simulink model "Adaptive_BS_jointspace"  (R2021b)
settings: Solver=VariableStepAuto  StartTime=0.0  StopTime=15.0  RelTol=1e1
undefined symbols (not defined in the file): Kd, l1, l2, l3, l4, l5, l6, lambda, m1, m2, m3, m4, m5, m6, q0, r
libraries: roblocks x3
(part 3 of 5)

== matlab function Adaptive_BS_jointspace/ABS control/reg2 ==
  data: q input; Yr output; qd input; qrd input; qrdd input
function Yr = reg(q, qd, qrd, qrdd)

q1 = q(1);
q2 = q(2);
q3 = q(3);
q4 = q(4);
q5 = q(5);
q6 = q(6);

qd1 = qd(1);
qd2 = qd(2);
qd3 = qd(3);
qd4 = qd(4);
qd5 = qd(5);
qd6 = qd(6);

qrd1 = qrd(1);
qrd2 = qrd(2);
qrd3 = qrd(3);
qrd4 = qrd(4);
qrd5 = qrd(5);
qrd6 = qrd(6);

qrdd1 = qrdd(1);
qrdd2 = qrdd(2);
qrdd3 = qrdd(3);
qrdd4 = qrdd(4);
qrdd5 = qrdd(5);
qrdd6 = qrdd(6);

%#codegen
%    This function was generated by the Symbolic Math Toolbox version 9.0.
%    01-Oct-2022 23:52:12

t2 = cos(q1);
t3 = cos(q2);
t4 = cos(q3);
t5 = cos(q4);
t6 = cos(q5);
t7 = cos(q6);
t8 = sin(q1);
t9 = sin(q2);
t10 = sin(q3);
t11 = sin(q4);
t12 = sin(q5);
t13 = sin(q6);
t14 = q2+q3;
t23 = -q5;
t15 = t2.^2;
t16 = t6.^2;
t17 = t8.^2;
t18 = t9.^2;
t19 = t12.^2;
t20 = cos(t14);
t21 = q4+t14;
t22 = sin(t14);
t24 = t2.*t6;
t26 = t2.*t12;
t27 = t6.*t8;
t30 = t8.*t12;
t33 = t3.*6.12e+3;
t34 = t9.*6.12e+3;
t56 = t3.*(1.53e+2./2.5e+2);
t57 = t2.*(1.53e+2./5.0e+2);
t63 = t9.*(1.53e+2./2.5e+2);
t64 = t8.*(1.53e+2./5.0e+2);
t90 = t2.*t3.*(-1.53e+2./2.5e+2);
t91 = t3.*t8.*(-1.53e+2./2.5e+2);
t92 = t2.*1.639e-1;
t93 = t2.*2.8615e-1;
t94 = t8.*1.639e-1;
t95 = t8.*2.8615e-1;
t119 = t3.*6.00372;
t138 = t8.*t9.*t10.*5.723e-1;
t148 = t2.*t3.*t4.*5.723e-1;
t152 = t2.*t3.*t10.*5.723e-1;
t153 = t2.*t4.*t9.*5.723e-1;
t154 = t3.*t4.*t8.*5.723e-1;
t157 = t2.*t9.*t10.*5.723e-1;
t158 = t3.*t8.*t10.*5.723e-1;
t159 = t4.*t8.*t9.*5.723e-1;
t25 = cos(t21);
t28 = q5+t21;
t29 = sin(t21);
t31 = t22.^2;
t41 = t21+t23;
t42 = t20.*5.723e+3;
t43 = t22.*5.723e+3;
t44 = t15+t17;
t71 = t2.*t56;
t74 = t2.*t63;
t75 = t8.*t56;
t79 = t8.*t63;
t109 = t20.*5.723e-1;
t110 = t24.*1.383e-1;
t111 = t24.*5.785e-2;
t112 = t22.*5.723e-1;
t113 = t26.*1.383e-1;
t114 = t27.*1.383e-1;
t115 = t26.*5.785e-2;
t116 = t27.*5.785e-2;
t117 = t30.*1.383e-1;
t118 = t30.*5.785e-2;
t122 = t5.*t20.*9.22e-2;
t123 = t11.*t20.*9.22e-2;
t124 = t5.*t22.*9.22e-2;
t125 = t11.*t22.*9.22e-2;
t127 = -t119;
t147 = t5.*t20.*1.157e-1;
t149 = t11.*t20.*1.157e-1;
t150 = t5.*t22.*1.157e-1;
t155 = t11.*t22.*1.157e-1;
t161 = -t138;
t173 = -t148;
t176 = t2.*t22.*(-5.723e-1);
t178 = t8.*t22.*(-5.723e-1);
t198 = t20.*5.614263;
t217 = t8.*t11.*t20.*(-1.157e-1);
t218 = t2.*t11.*t22.*(-1.157e-1);
t219 = t5.*t8.*t22.*(-1.157e-1);
t220 = t8.*t11.*t22.*(-1.157e-1);
t261 = t57+t91;
t331 = t17.*t20.*t22.*3.2752729e-1;
t338 = t15.*t20.*t22.*3.2752729e-1;
t32 = sin(t28);
t35 = t25.^2;
t36 = t29.^2;
t37 = t7.*t25;
t38 = t13.*t25;
t39 = t7.*t29;
t40 = t13.*t29;
t45 = sin(t41);
t46 = t24.*t25;
t49 = t25.*t26;
t50 = t25.*t27;
t58 = t25.*t30;
t87 = t25.*t29.*2.0;
t96 = t6.*t25.*t29;
t97 = t12.*t25.*t29;
t126 = -t109;
t128 = t25.*1.157e-1;
t129 = t25.*8.195e-2;
t130 = t29.*1.157e-1;
t131 = t29.*8.195e-2;
t137 = -t125;
t139 = t12.*t25.*4.61e-2;
t140 = t6.*t29.*4.61e-2;
t141 = t12.*t29.*4.61e-2;
t145 = t33+t42;
t146 = t34+t43;
t151 = t2.*t112;
t156 = t8.*t112;
t164 = t12.*t25.*5.785e-2;
t167 = t12.*t29.*5.785e-2;
t174 = -t149;
t175 = -t150;
t177 = -t155;
t179 = t15.*t112;
t180 = t17.*t112;
t182 = t8.*t29.*(-8.195e-2);
t184 = t2.*t147;
t185 = t2.*t149;
t186 = t8.*t147;
t187 = t2.*t150;
t188 = t8.*t149;
t189 = t2.*t155;
t190 = t8.*t150;
t193 = t8.*t155;
t208 = t29.*t113;
t210 = t29.*t115;
t211 = t29.*t117;
t212 = t29.*t118;
t213 = (t15.*t44)./5.0e+3;
t214 = (t17.*t44)./5.0e+3;
t222 = -t198;
t230 = t29.*1.135017;
t231 = t29.*8.039295e-1;
t236 = (t19.*t25.*t29)./2.5e+3;
t237 = (t19.*t25.*t29)./5.0e+3;
t253 = t64+t71;
t276 = t56+t109;
t277 = t63+t112;
t299 = t8.*t261;
t335 = t123+t124;
t346 = t15.*t25.*t29.*6.7158025e-3;
t348 = t17.*t25.*t29.*6.7158025e-3;
t376 = t74.*t261;
t377 = t79.*t261;
t487 = t25.*t29.*2.138600833333333e-3;
t508 = t25.*t29.*1.215540833333333e-3;
t509 = t25.*t29.*2.431081666666667e-3;
t513 = t15.*t44.*2.338600833333333e-3;
t514 = t17.*t44.*2.338600833333333e-3;
t47 = t2.*t37;
t48 = t6.*t37;
t51 = t2.*t38;
t52 = t8.*t37;
t53 = t2.*t39;
t54 = t6.*t38;
t55 = t6.*t39;
t59 = t8.*t38;
t60 = t2.*t40;
t61 = t8.*t39;
t62 = t6.*t40;
t65 = t8.*t40;
t66 = t6.*t35;
t67 = t12.*t35;
t68 = t6.*t36;
t69 = t12.*t36;
t70 = t24.*t39;
t72 = t24.*t40;
t73 = t27.*t39;
t76 = t15.*t36;
t78 = t27.*t40;
t80 = t17.*t36;
t81 = t19.*t36;
t82 = -t49;
t83 = -t50;
t98 = -t87;
t120 = t12.*t29.*t37;
t121 = t12.*t29.*t38;
t132 = t24+t58;
t133 = t30+t46;
t134 = t15.*t87;
t135 = t17.*t87;
t136 = t19.*t87;
t142 = -t128;
t143 = -t130;
t144 = -t131;
t163 = t2.*t129;
t165 = t8.*t129;
t166 = t2.*t131;
t168 = t8.*t131;
t181 = -t164;
t201 = t46.*1.383e-1;
t202 = t46.*5.785e-2;
t203 = t49.*1.383e-1;
t204 = t50.*1.383e-1;
t205 = t49.*5.785e-2;
t206 = t50.*5.785e-2;
t207 = t58.*1.383e-1;
t209 = t58.*5.785e-2;
t215 = t15.*t129;
t216 = t17.*t129;
t242 = t36.*t111;
t243 = t36.*t116;
t244 = -t236;
t245 = -t237;
t246 = t32.*6.783615e-1;
t247 = t32.*2.8375425e-1;
t252 = t27.*t36.*(-5.785e-2);
t266 = t45.*6.783615e-1;
t267 = t45.*2.8375425e-1;
t279 = t2.*t253;
t296 = (t2.*t145)./1.0e+4;
t297 = (t8.*t145)./1.0e+4;
t298 = (t2.*t146)./1.0e+4;
t301 = (t8.*t146)./1.0e+4;
t302 = t277.^2;
t317 = (t15.*t146)./1.0e+4;
t322 = (t17.*t146)./1.0e+4;
t324 = -t299;
t343 = t122+t137;
t347 = t112+t129;
t355 = t126+t131;
t359 = t6.*t335;
t360 = t12.*t335;
t363 = t128+t167;
t367 = t74.*t253;
t368 = t79.*t253;
t384 = t9.*t299.*(-1.53e+2./2.5e+2);
t390 = t179+t180;
t408 = t129+t277;
t447 = t180.*t277;
t454 = t15.*t109.*t277;
t459 = t17.*t109.*t277;
t460 = t179.*t277;
t479 = t35.*1.215540833333333e-3;
t490 = t2.*t36.*1.215540833333333e-3;
t492 = t8.*t36.*1.215540833333333e-3;
t510 = t16.*t36.*1.215540833333333e-3;
t516 = -t509;
t517 = -t508;
t527 = t2.*t508;
t528 = t8.*t508;
t542 = t16.*t508;
t543 = t16.*t509;
t567 = t184+t208+t218;
t568 = t184+t210+t218;
t569 = t186+t211+t220;
t570 = t186+t212+t220;
t638 = t92+t154+t161+t182;
t77 = -t48;
t84 = -t60;
t85 = -t61;
t86 = -t62;
t88 = -t68;
t89 = -t69;
t99 = t12.*t68.*2.0;
t100 = t17.*t69;
t101 = t13.*t81;
t102 = -t72;
t103 = -t78;
t105 = t15.*t68;
t106 = t17.*t68;
t107 = t15.*t69;
t108 = t7.*t81;
t160 = t132.^2;
t162 = t81./5.0e+3;
t169 = (t12.*t68)./2.5e+3;
t170 = (t12.*t68)./5.0e+3;
t171 = t26+t83;
t172 = t27+t82;
t191 = t2.*t132;
t192 = t7.*t133;
t194 = t38+t55;
t195 = t39+t54;
t196 = t8.*t133;
t197 = t13.*t133;
t223 = -t203;
t224 = -t204;
t225 = -t205;
t226 = -t206;
t251 = t51+t70;
t254 = t59+t73;
t257 = -t246;
t258 = -t247;
t259 = t8.*t81.*1.383e-1;
t260 = t8.*t29.*t132;
t262 = t2.*t25.*t133;
t263 = t2.*t81.*1.383e-1;
t264 = t8.*t25.*t132;
t265 = t2.*t29.*t133;
t280 = t61.*t132;
t284 = t65.*t132;
t300 = t29.*t30.*t132.*2.0;
t305 = -t297;
t310 = -t298;
t313 = -t301;
t325 = (t12.*t29.*t132)./5.0e+3;
t326 = (t12.*t29.*t133)./5.0e+3;
t329 = (t12.*t25.*t132)./5.0e+3;
t330 = (t6.*t29.*t132)./5.0e+3;
t342 = t35+t76+t80;
t358 = t347.^2;
t364 = t12.*t343;
t370 = t130+t181;
t371 = t110+t207;
t372 = t117+t201;
t373 = t118+t202;
t378 = t132.*t208;
t379 = t363.^2;
t403 = t95+t296;
t405 = t215+t216;
t423 = t144+t276;
t424 = t2.*t25.*t363;
t425 = t8.*t25.*t363;
t426 = t2.*t29.*t363;
t427 = t8.*t29.*t363;
t432 = t408.^2;
t434 = -t2.*(t298-t2.*t9.*(1.53e+2./2.5e+2));
t440 = -t8.*(t301-t8.*t9.*(1.53e+2./2.5e+2));
t462 = t98+t134+t135;
t480 = t112+t363;
t481 = t109+t143+t164;
t488 = t2.*t479;
t489 = t8.*t479;
t491 = t140+t359;
t493 = t215.*t347;
t494 = t216.*t347;
t495 = t15.*t131.*t347;
t497 = t17.*t131.*t347;
t498 = -t490;
t499 = -t492;
t500 = t152+t153+t163;
t503 = t215.*t355;
t504 = t216.*t355;
t507 = t158+t159+t165;
t518 = t12.*t68.*1.015540833333333e-3;
t529 = t279+t324;
t530 = t16.*t490;
t531 = t16.*t492;
t551 = t6.*t15.*t29.*t363.*5.785e-2;
t552 = t6.*t15.*t29.*t363.*2.8925e-2;
t553 = t6.*t17.*t29.*t363.*5.785e-2;
t554 = t6.*t17.*t29.*t363.*2.8925e-2;
t561 = t317+t322;
t574 = t277+t363;
t575 = t143+t164+t276;
t577 = t215.*t408;
t578 = t216.*t408;
t579 = t15.*t131.*t408;
t581 = t17.*t131.*t408;
t582 = t2.*t567;
t583 = t2.*t568;
t584 = t8.*t569;
t585 = t8.*t570;
t586 = t15.*t29.*t408.*(-8.195e-2);
t587 = t17.*t29.*t408.*(-8.195e-2);
t603 = t6.*t25.*t133.*1.215540833333333e-3;
t604 = t6.*t29.*t132.*1.015540833333333e-3;
t605 = t6.*t29.*t133.*1.215540833333333e-3;
t606 = t12.*t29.*t133.*1.015540833333333e-3;
t608 = t25.*t567;
t609 = t25.*t568;
t610 = t25.*t569;
t611 = t25.*t570;
t623 = t94+t157+t166+t173;
t631 = t8.*t29.*t567;
t632 = t8.*t29.*t568;
t634 = t2.*t29.*t569;
t635 = t2.*t29.*t570;
t643 = t15.*t347.*t355;
t646 = t17.*t347.*t355;
t650 = t8.*t638;
t668 = t368+t376;
t671 = t367+t384;
t686 = t111+t209+t217+t219;
t694 = t15.*t347.*t408;
t695 = t17.*t347.*t408;
t696 = t75+t638;
t702 = t15.*t355.*t408;
t703 = t17.*t355.*t408;
t763 = t141+t147+t177+t360;
t811 = t158+t159+t569;
t812 = t158+t159+t570;
t818 = t152+t153+t567;
t819 = t152+t153+t568;
t1021 = t236+t516+t543;
t104 = -t99;
t183 = -t170;
t199 = t172.^2;
t200 = t8.*t162;
t221 = t2.*t162;
t227 = t7.*t160;
t228 = t194.^2;
t229 = t13.*t160;
t232 = t7.*t191;
t233 = t13.*t191;
t234 = t2.*t171;
t235 = t7.*t171;
t238 = t37+t86;
t239 = t40+t77;
t240 = t8.*t172;
t241 = t13.*t171;
t268 = t25.*t194;
t269 = t25.*t195;
t270 = t29.*t194;
t271 = t47+t102;
t272 = t52+t103;
t273 = -t263;
t274 = t8.*t29.*t171;
t275 = -t260;
t278 = t8.*t251;
t281 = t2.*t254;
t282 = t2.*t25.*t172;
t283 = -t262;
t285 = t8.*t25.*t171;
t286 = t2.*t29.*t172;
t287 = -t264;
t288 = -t265;
t292 = t12.*t29.*t195;
t303 = t53.*t172;
t306 = t60.*t172;
t307 = t85.*t132;
t311 = -t300;
t312 = -t284;
t323 = t26.*t29.*t172.*2.0;
t327 = t53+t197;
t332 = -t325;
t333 = -t326;
t334 = t8.*t29.*t254;
t337 = t2.*t29.*t251;
t339 = -t329;
t340 = (t12.*t29.*t171)./5.0e+3;
t341 = (t12.*t29.*t172)./5.0e+3;
t344 = t84+t192;
t349 = (t12.*t25.*t172)./5.0e+3;
t350 = (t6.*t29.*t172)./5.0e+3;
t366 = -t8.*(t60-t192);
t374 = t132.*t171.*2.0;
t375 = t133.*t172.*2.0;
t380 = t113+t224;
t381 = t114+t223;
t382 = t115+t226;
t387 = t172.*t211;
t388 = t2.*t372;
t389 = t2.*t373;
t391 = t132.*t254;
t393 = -t2.*t25.*(t60-t192);
t395 = -t2.*t29.*(t60-t192);
t402 = t74+t310;
t404 = t79+t313;
t406 = t25.*t372;
t407 = t25.*t373;
t409 = t93+t305;
t410 = t172.*t251;
t413 = -t26.*t29.*(t60-t192);
t414 = t2.*t29.*(t60-t192);
t428 = t8.*t29.*t372;
t429 = t12.*t29.*t371;
t430 = t12.*t29.*t372;
t431 = t8.*t29.*t373;
t435 = t2.*t29.*t370;
t436 = t2.*t403;
t437 = t8.*t29.*t370;
t439 = t26.*t29.*(t60-t192);
t443 = t12.*t25.*t371;
t444 = t6.*t29.*t371;
t448 = -t424;
t449 = -t425;
t450 = -t426;
t464 = t26.*t29.*t371;
t475 = -t133.*(t60-t192);
t482 = -t172.*(t60-t192);
t483 = t133.*(t60-t192);
t496 = t480.^2;
t505 = t132.*t372;
t506 = t133.*t371;
t511 = t90+t403;
t525 = t172.*t371;
t540 = t2.*t500;
t541 = t8.*t507;
t555 = t8.*t109.*t403;
t556 = t151.*t403;
t558 = t156.*t403;
t572 = t2.*t29.*t491;
t573 = t8.*t29.*t491;
t580 = t574.^2;
t595 = t74+t500;
t596 = t79+t507;
t619 = -t603;
t620 = -t604;
t621 = -t605;
Yr = ft_1({qd1,qd2,qd3,qd4,qd5,qd6,qrd1,qrd2,qrd3,qrd4,qrd5,qrd6,qrdd1,qrdd2,qrdd3,qrdd4,qrdd5,qrdd6,t100,t101,t1021,t104,t105,t106,t107,t108,t109,t111,t112,t116,t12,t120,t121,t127,t13,t130,t132,t133,t136,t139,t142,t144,t146,t15,t151,t154,t156,t157,t160,t161,t162,t163,t165,t166,t168,t169,t17,t170,t171,t172,t173,t174,t175,t176,t178,t179,t18,t180,t183,t185,t187,t191,t192,t194,t195,t196,t199,t2,t20,t200,t213,t214,t215,t216,t217,t219,t221,t222,t225,t227,t228,t229,t230,t231,t232,t233,t234,t235,t237,t238,t239,t24,t240,t241,t242,t243,t244,t245,t25,t251,t252,t253,t254,t257,t258,t259,t26,t261,t263,t266,t267,t268,t269,t27,t270,t271,t272,t273,t274,t275,t276,t277,t278,t279,t281,t282,t283,t285,t286,t287,t288,t29,t292,t296,t298,t3,t30,t301,t302,t303,t305,t306,t307,t31,t311,t312,t323,t325,t326,t327,t330,t331,t332,t333,t334,t337,t338,t339,t340,t341,t342,t346,t347,t348,t349,t35,t350,t355,t358,t36,t363,t364,t366,t370,t371,t372,t373,t374,t375,t377,t378,t379,t380,t381,t382,t387,t388,t389,t39,t390,t391,t393,t40,t402,t403,t404,t405,t406,t407,t408,t409,t410,t414,t423,t424,t426,t427,t428,t429,t430,t431,t432,t434,t435,t436,t437,t439,t440,t443,t444,t447,t448,t449,t450,t454,t459,t460,t462,t464,t479,t480,t481,t482,t483,t487,t488,t489,t491,t493,t494,t495,t496,t497,t498,t499,t500,t503,t504,t505,t506,t507,t510,t511,t513,t514,t517,t518,t525,t527,t528,t529,t530,t531,t540,t541,t542,t551,t552,t553,t554,t555,t556,t558,t561,t567,t568,t569,t570,t572,t573,t574,t575,t577,t578,t579,t580,t581,t582,t583,t584,t585,t586,t587,t595,t596,t6,t60,t604,t606,t608,t609,t61,t610,t611,t619,t620,t621,t623,t63,t631,t632,t634,t635,t643,t646,t65,t650,t66,t668,t67,t68,t686,t694,t695,t696,t7,t702,t703,t71,t74,t75,t763,t79,t8,t81,t811,t812,t818,t819,t85,t88,t89,t9,t90,t92,t94,t96,t97});
end
function Yr = ft_1(ct)
qd1 = ct{1};
qd2 = ct{2};
qd3 = ct{3};
qd4 = ct{4};
qd5 = ct{5};
qd6 = ct{6};
qrd1 = ct{7};
qrd2 = ct{8};
qrd3 = ct{9};
qrd4 = ct{10};
qrd5 = ct{11};
qrd6 = ct{12};
qrdd1 = ct{13};
qrdd2 = ct{14};
qrdd3 = ct{15};
qrdd4 = ct{16};
qrdd5 = ct{17};
qrdd6 = ct{18};
t100 = ct{19};
t101 = ct{20};
t1021 = ct{21};
t104 = ct{22};
t105 = ct{23};
t106 = ct{24};
t107 = ct{25};
t108 = ct{26};
t109 = ct{27};
t111 = ct{28};
t112 = ct{29};
t116 = ct{30};
t12 = ct{31};
t120 = ct{32};
t121 = ct{33};
t127 = ct{34};
t13 = ct{35};
t130 = ct{36};
t132 = ct{37};
t133 = ct{38};
t136 = ct{39};
t139 = ct{40};
t142 = ct{41};
t144 = ct{42};
t146 = ct{43};
t15 = ct{44};
t151 = ct{45};
t154 = ct{46};
t156 = ct{47};
t157 = ct{48};
t160 = ct{49};
t161 = ct{50};
t162 = ct{51};
t163 = ct{52};
t165 = ct{53};
t166 = ct{54};
t168 = ct{55};
t169 = ct{56};
t17 = ct{57};
t170 = ct{58};
t171 = ct{59};
t172 = ct{60};
t173 = ct{61};
t174 = ct{62};
t175 = ct{63};
t176 = ct{64};
t178 = ct{65};
t179 = ct{66};
t18 = ct{67};
t180 = ct{68};
t183 = ct{69};
t185 = ct{70};
t187 = ct{71};
t191 = ct{72};
t192 = ct{73};
t194 = ct{74};
t195 = ct{75};
t196 = ct{76};
t199 = ct{77};
t2 = ct{78};
t20 = ct{79};
t200 = ct{80};
t213 = ct{81};
t214 = ct{82};
t215 = ct{83};
t216 = ct{84};
t217 = ct{85};
t219 = ct{86};
t221 = ct{87};
t222 = ct{88};
t225 = ct{89};
t227 = ct{90};
t228 = ct{91};
t229 = ct{92};
t230 = ct{93};
t231 = ct{94};
t232 = ct{95};
t233 = ct{96};
t234 = ct{97};
t235 = ct{98};
t237 = ct{99};
t238 = ct{100};
t239 = ct{101};
t24 = ct{102};
t240 = ct{103};
t241 = ct{104};
t242 = ct{105};
t243 = ct{106};
t244 = ct{107};
t245 = ct{108};
t25 = ct{109};
t251 = ct{110};
t252 = ct{111};
t253 = ct{112};
t254 = ct{113};
t257 = ct{114};
t258 = ct{115};
t259 = ct{116};
t26 = ct{117};
t261 = ct{118};
t263 = ct{119};
t266 = ct{120};
t267 = ct{121};
t268 = ct{122};
t269 = ct{123};
t27 = ct{124};
t270 = ct{125};
t271 = ct{126};
t272 = ct{127};
t273 = ct{128};
t274 = ct{129};
t275 = ct{130};
t276 = ct{131};
t277 = ct{132};
t278 = ct{133};
t279 = ct{134};
t281 = ct{135};
t282 = ct{136};
t283 = ct{137};
t285 = ct{138};
t286 = ct{139};
t287 = ct{140};
t288 = ct{141};
t29 = ct{142};
t292 = ct{143};
t296 = ct{144};
t298 = ct{145};
t3 = ct{146};
t30 = ct{147};
t301 = ct{148};
t302 = ct{149};
t303 = ct{150};
t305 = ct{151};
t306 = ct{152};
t307 = ct{153};
t31 = ct{154};
t311 = ct{155};
t312 = ct{156};
t323 = ct{157};
t325 = ct{158};
t326 = ct{159};
t327 = ct{160};
t330 = ct{161};
t331 = ct{162};
t332 = ct{163};
t333 = ct{164};
t334 = ct{165};
t337 = ct{166};
t338 = ct{167};
t339 = ct{168};
t340 = ct{169};
t341 = ct{170};
t342 = ct{171};
t346 = ct{172};
t347 = ct{173};
t348 = ct{174};
t349 = ct{175};
t35 = ct{176};
t350 = ct{177};
t355 = ct{178};
t358 = ct{179};
t36 = ct{180};
t363 = ct{181};
t364 = ct{182};
t366 = ct{183};
t370 = ct{184};
t371 = ct{185};
t372 = ct{186};
t373 = ct{187};
t374 = ct{188};
t375 = ct{189};
t377 = ct{190};
t378 = ct{191};
t379 = ct{192};
t380 = ct{193};
t381 = ct{194};
t382 = ct{195};
t387 = ct{196};
t388 = ct{197};
t389 = ct{198};
t39 = ct{199};
t390 = ct{200};
t391 = ct{201};
t393 = ct{202};
t40 = ct{203};
t402 = ct{204};
t403 = ct{205};
t404 = ct{206};
t405 = ct{207};
t406 = ct{208};
t407 = ct{209};
t408 = ct{210};
t409 = ct{211};
t410 = ct{212};
t414 = ct{213};
t423 = ct{214};
t424 = ct{215};
t426 = ct{216};
t427 = ct{217};
t428 = ct{218};
t429 = ct{219};
t430 = ct{220};
t431 = ct{221};
t432 = ct{222};
t434 = ct{223};
t435 = ct{224};
t436 = ct{225};
t437 = ct{226};
t439 = ct{227};
t440 = ct{228};
t443 = ct{229};
t444 = ct{230};
t447 = ct{231};
t448 = ct{232};
t449 = ct{233};
t450 = ct{234};
t454 = ct{235};
t459 = ct{236};
t460 = ct{237};
t462 = ct{238};
t464 = ct{239};
t479 = ct{240};
t480 = ct{241};
t481 = ct{242};
t482 = ct{243};
t483 = ct{244};
t487 = ct{245};
t488 = ct{246};
t489 = ct{247};
t491 = ct{248};
t493 = ct{249};
t494 = ct{250};
t495 = ct{251};
t496 = ct{252};
t497 = ct{253};
t498 = ct{254};
t499 = ct{255};
t500 = ct{256};
t503 = ct{257};
t504 = ct{258};
t505 = ct{259};
t506 = ct{260};
t507 = ct{261};
t510 = ct{262};
t511 = ct{263};
t513 = ct{264};
t514 = ct{265};
t517 = ct{266};
t518 = ct{267};
t525 = ct{268};
t527 = ct{269};
t528 = ct{270};
t529 = ct{271};
t530 = ct{272};
t531 = ct{273};
t540 = ct{274};
t541 = ct{275};
t542 = ct{276};
t551 = ct{277};
t552 = ct{278};
t553 = ct{279};
t554 = ct{280};
t555 = ct{281};
t556 = ct{282};
t558 = ct{283};
t561 = ct{284};
t567 = ct{285};
t568 = ct{286};
t569 = ct{287};
t570 = ct{288};
t572 = ct{289};
t573 = ct{290};
t574 = ct{291};
t575 = ct{292};
t577 = ct{293};
t578 = ct{294};
t579 = ct{295};
t580 = ct{296};
t581 = ct{297};
t582 = ct{298};
t583 = ct{299};
t584 = ct{300};
t585 = ct{301};
t586 = ct{302};
t587 = ct{303};
t595 = ct{304};
t596 = ct{305};
t6 = ct{306};
t60 = ct{307};
t604 = ct{308};
t606 = ct{309};
t608 = ct{310};
t609 = ct{311};
t61 = ct{312};
t610 = ct{313};
t611 = ct{314};
t619 = ct{315};
t620 = ct{316};
t621 = ct{317};
t623 = ct{318};
t63 = ct{319};
t631 = ct{320};
t632 = ct{321};
t634 = ct{322};
t635 = ct{323};
t643 = ct{324};
t646 = ct{325};
t65 = ct{326};
t650 = ct{327};
t66 = ct{328};
t668 = ct{329};
t67 = ct{330};
t68 = ct{331};
t686 = ct{332};
t694 = ct{333};
t695 = ct{334};
t696 = ct{335};
t7 = ct{336};
t702 = ct{337};
t703 = ct{338};
t71 = ct{339};
t74 = ct{340};
t75 = ct{341};
t763 = ct{342};
t79 = ct{343};
t8 = ct{344};
t81 = ct{345};
t811 = ct{346};
t812 = ct{347};
t818 = ct{348};
t819 = ct{349};
t85 = ct{350};
t88 = ct{351};
t89 = ct{352};
t9 = ct{353};
t90 = ct{354};
t92 = ct{355};
t94 = ct{356};
t96 = ct{357};
t97 = ct{358};
t626 = t6.*t25.*t171.*1.215540833333333e-3;
t627 = t6.*t29.*t171.*1.215540833333333e-3;
t628 = t6.*t29.*t172.*1.015540833333333e-3;
t629 = t298.*t403;
t630 = t12.*t29.*t171.*1.015540833333333e-3;
t633 = -t608;
t639 = t132.*t491;
t642 = t2.*t623;
t644 = t8.*t277.*t403;
t647 = -t634;
t648 = -t635;
t649 = t172.*t491;
t652 = t176+t500;
t653 = t178+t507;
t656 = t8.*t25.*t500.*4.0975e-2;
t657 = t12.*t39.*t194.*8.084033333333334e-4;
t658 = t12.*t39.*t194.*1.616806666666667e-3;
t659 = t2.*t25.*t507.*4.0975e-2;
t663 = t6.*t15.*t29.*t480.*5.785e-2;
t664 = t6.*t15.*t29.*t480.*2.8925e-2;
t666 = t6.*t17.*t29.*t480.*5.785e-2;
t667 = t6.*t17.*t29.*t480.*2.8925e-2;
t670 = -t650;
t681 = t116+t185+t187+t225;
t683 = t15.*t363.*t370;
t684 = t17.*t363.*t370;
t685 = t217+t219+t371;
t689 = (t8.*t363.*t373)./2.0;
t701 = t7.*t132.*t194.*8.084033333333334e-4;
t704 = t90+t623;
t705 = t25.*t342.*1.215540833333333e-3;
t706 = t29.*t342.*6.077704166666666e-4;
t707 = t29.*t342.*1.215540833333333e-3;
t719 = t6.*t15.*t29.*t574.*5.785e-2;
t720 = t6.*t15.*t29.*t574.*2.8925e-2;
t722 = t6.*t17.*t29.*t574.*5.785e-2;
t723 = t6.*t17.*t29.*t574.*2.8925e-2;
t726 = t7.*t172.*t194.*8.084033333333334e-4;
t730 = t25.*t686;
t733 = t29.*t686;
t739 = t8.*t696;
t751 = t12.*t39.*(t60-t192).*(-8.084033333333334e-4);
t760 = t194.*t251.*8.084033333333334e-4;
t761 = t194.*t254.*8.084033333333334e-4;
t766 = t763.^2;
t770 = t434+t440;
t774 = t139+t174+t175+t364;
t775 = t15.*t363.*t480;
t776 = t17.*t363.*t480;
t781 = t15.*t363.*t481;
t782 = t15.*t370.*t480;
t783 = t17.*t363.*t481;
t784 = t17.*t370.*t480;
t795 = (t8.*t373.*t480)./2.0;
t813 = t25.*t462.*6.077704166666666e-4;
t814 = t25.*t462.*1.215540833333333e-3;
t816 = t194.*(t60-t192).*(-8.084033333333334e-4);
t820 = t2.*t25.*t763;
t821 = t8.*t25.*t763;
t822 = t2.*t29.*t763;
t823 = t8.*t29.*t763;
t824 = t194.*(t60-t192).*8.084033333333334e-4;
t827 = t2.*t29.*t462.*1.215540833333333e-3;
t828 = t8.*t29.*t462.*1.215540833333333e-3;
t834 = t2.*t818;
t835 = t2.*t819;
t840 = t8.*t811;
t841 = t8.*t812;
t846 = t163.*t696;
t847 = t165.*t696;
t848 = t166.*t696;
t853 = t15.*t363.*t574;
t854 = t17.*t363.*t574;
t858 = (t2.*t408.*t507)./2.0;
t859 = t15.*t370.*t574;
t860 = t17.*t370.*t574;
t862 = (t8.*t408.*t500)./2.0;
t863 = t112+t763;
t864 = (t8.*t373.*t574)./2.0;
t882 = t142+t763;
t887 = t74+t818;
t888 = t74+t819;
t889 = t15.*t480.*t481;
t890 = t17.*t480.*t481;
t891 = t79+t811;
t892 = t79+t812;
t899 = t305+t696;
t911 = t178+t811;
t912 = t178+t812;
t914 = t277+t763;
t916 = t176+t818;
t917 = t176+t819;
t928 = t2.*t347.*t696;
t929 = t15.*t480.*t574;
t932 = t17.*t480.*t574;
t934 = t2.*t355.*t696;
t935 = t15.*t481.*t574;
t936 = t17.*t481.*t574;
t940 = (t8.*t480.*t568)./2.0;
t941 = (t2.*t480.*t570)./2.0;
t966 = t162+t479+t510;
t977 = t92+t154+t161+t686;
t983 = t2.*t408.*t696;
t985 = (t2.*t570.*t574)./2.0;
t992 = (t8.*t568.*t574)./2.0;
t993 = t582+t584;
t994 = t583+t585;
t1007 = (t8.*t372.*t763)./2.0;
t1027 = t507.*t696;
t1039 = (t8.*t363.*t819)./2.0;
t1041 = (t2.*t363.*t812)./2.0;
t1079 = (t25.*t1021)./2.0;
t1086 = t15.*t491.*t763;
t1087 = t17.*t491.*t763;
t1142 = (t2.*t574.*t812)./2.0;
t1146 = (t8.*t574.*t819)./2.0;
t1259 = (t8.*t763.*t818)./2.0;
t1260 = (t2.*t763.*t811)./2.0;
t248 = t7.*t199;
t249 = t238.^2;
t250 = t13.*t199;
t255 = t7.*t240;
t256 = t13.*t240;
t289 = t12.*t268;
t290 = t6.*t270;
t291 = t12.*t270;
t293 = t25.*t238;
t294 = t25.*t239;
t295 = t29.*t238;
t304 = t8.*t271;
t308 = t2.*t272;
t309 = -t281;
t319 = t12.*t29.*t239;
t321 = -t292;
t345 = t65+t235;
t351 = -t340;
t352 = t8.*t29.*t272;
t353 = -t334;
t354 = t8.*t327;
t356 = t2.*t29.*t271;
t357 = -t337;
t361 = t85+t241;
t383 = -t2.*(t61-t241);
t385 = t2.*t25.*t327;
t386 = t2.*t29.*t327;
t392 = t26.*t29.*t327;
t397 = t8.*t380;
t398 = t8.*t382;
t400 = t191+t240;
t401 = t196+t234;
t411 = t132.*t272;
t412 = -t391;
t416 = -t8.*t25.*(t61-t241);
t420 = -t8.*t29.*(t61-t241);
t421 = t25.*t380;
t422 = t25.*t382;
t433 = t172.*t271;
t441 = -t29.*t30.*(t61-t241);
t442 = t8.*t29.*(t61-t241);
t445 = t12.*t29.*t380;
t446 = t12.*t29.*t381;
t451 = t8.*t409;
t455 = t2.*t29.*t380;
t456 = t12.*t25.*t381;
t457 = t6.*t29.*t381;
t458 = t2.*t29.*t382;
t461 = -t429;
t463 = t29.*t30.*(t61-t241);
t465 = -t443;
t466 = -t444;
t468 = t133.*t327;
t470 = t29.*t30.*t381;
t473 = -t464;
t474 = t172.*t327;
t485 = -t132.*(t61-t241);
t486 = t81+t160+t199;
t501 = -t171.*(t61-t241);
t512 = t75+t409;
t515 = t132.*t381;
t522 = t171.*(t61-t241);
t526 = -t506;
t538 = t171.*t381;
t539 = t172.*t380;
t548 = t2.*t511;
t549 = -t525;
t563 = t2.*t109.*t409;
t564 = t151.*t409;
t565 = t156.*t409;
t571 = t178.*t409;
t576 = -t573;
t591 = t228.*8.084033333333334e-4;
t592 = t242+t407;
t612 = t96+t274+t288;
t615 = t97+t275+t286;
t625 = t8.*t596;
t636 = t2.*t595;
t640 = -t628;
t641 = t301.*t409;
t651 = t2.*t277.*t409;
t660 = t120+t303+t307;
t661 = t121+t306+t312;
t662 = -t656;
t665 = -t658;
t669 = -t659;
t672 = t12.*t40.*t238.*8.084033333333334e-4;
t673 = t12.*t40.*t238.*1.616806666666667e-3;
t674 = t136+t311+t323;
t677 = t2.*t652;
t678 = t8.*t653;
t680 = t185+t187+t381;
t691 = (t2.*t363.*t382)./2.0;
t692 = -t689;
t710 = -t701;
t712 = t25.*t681;
t714 = t29.*t681;
t715 = -t707;
t716 = -t706;
t727 = t12.*t40.*t327.*8.084033333333334e-4;
t728 = t13.*t132.*t238.*8.084033333333334e-4;
t729 = t25.*t685;
t731 = t2.*t705;
t732 = t29.*t685;
t734 = t8.*t705;
t735 = t2.*t707;
t736 = t8.*t707;
t737 = t2.*t704;
t738 = t2.*t25.*t596.*4.0975e-2;
t742 = -t726;
t746 = t194.*t239.*8.084033333333334e-4;
t747 = t194.*t239.*1.616806666666667e-3;
t748 = t195.*t238.*8.084033333333334e-4;
t749 = t195.*t238.*1.616806666666667e-3;
t750 = t8.*t25.*t595.*4.0975e-2;
t753 = t2.*t730;
t755 = t13.*t172.*t238.*8.084033333333334e-4;
t757 = t2.*t733;
t759 = -t739;
t762 = t12.*t40.*(t61-t241).*(-8.084033333333334e-4);
t764 = t104+t374+t375;
t768 = t238.*t271.*8.084033333333334e-4;
t769 = t238.*t272.*8.084033333333334e-4;
t796 = t195.*t327.*8.084033333333334e-4;
t801 = -t782;
t802 = (t2.*t382.*t480)./2.0;
t803 = -t784;
t804 = -t795;
t806 = t402+t500;
t809 = t404+t507;
t815 = t238.*t327.*8.084033333333334e-4;
t829 = t239.*(t60-t192).*(-8.084033333333334e-4);
t831 = t195.*(t61-t241).*(-8.084033333333334e-4);
t836 = t2.*t29.*t774;
t837 = t8.*t29.*t774;
t838 = -t821;
t839 = -t822;
t843 = t163.*t704;
t844 = t165.*t704;
t845 = t168.*t704;
t849 = t238.*(t61-t241).*(-8.084033333333334e-4);
t851 = t25.*t739.*(-8.195e-2);
t870 = -t862;
t871 = (t2.*t382.*t574)./2.0;
t872 = -t864;
t873 = t66+t88+t105+t106+t283+t285;
t875 = (t8.*t347.*t595)./2.0;
t876 = t67+t89+t100+t107+t282+t287;
t877 = t406+t572;
t878 = (t2.*t347.*t596)./2.0;
t879 = t109+t774;
t881 = t863.^2;
t885 = t130+t774;
t893 = t296+t704;
t900 = t2.*t887;
t901 = t2.*t888;
t902 = t8.*t891;
t903 = t8.*t892;
t909 = t8.*t899;
t919 = t540+t541;
t921 = t276+t774;
t922 = t26.*t29.*t882;
t923 = t914.^2;
t924 = t29.*t30.*t882;
t925 = t8.*t347.*t704;
t926 = t2.*t916;
t927 = t2.*t917;
t930 = t8.*t911;
t931 = t8.*t912;
t933 = t8.*t355.*t704;
t946 = -t940;
t960 = t132.*t882;
t961 = t133.*t882;
t968 = t94+t157+t173+t681;
t969 = t171.*t882;
t970 = t172.*t882;
t976 = t92+t154+t161+t685;
t982 = t8.*t408.*t704;
t990 = t427+t730;
t1000 = t8.*t977;
t1002 = -t992;
t1012 = (t2.*t380.*t763)./2.0;
t1013 = -t1007;
t1019 = (t29.*t966)./2.0;
t1028 = t404+t811;
t1029 = t404+t812;
t1033 = t500.*t704;
t1037 = t402+t818;
t1038 = t402+t819;
t1045 = -t1027;
t1047 = t620+t630;
t1050 = -t1039;
t1052 = t75+t977;
t1054 = -t1041;
t1077 = t2.*(t604-t630).*(-1.0./2.0);
t1080 = (t2.*(t604-t630))./2.0;
t1082 = (t8.*t372.*t863)./2.0;
t1085 = t642+t670;
t1090 = (t2.*t380.*t863)./2.0;
t1092 = t596.*t696;
t1095 = t595.*t704;
t1100 = (t8.*t363.*t888)./2.0;
t1101 = t1086./2.0;
t1103 = t1087./2.0;
t1104 = (t2.*t363.*t892)./2.0;
t1119 = (t8.*t372.*t914)./2.0;
t1120 = (t2.*t380.*t914)./2.0;
t1122 = t341+t527+t621;
t1123 = t332+t528+t627;
t1140 = t15.*t491.*t863;
t1141 = t17.*t491.*t863;
t1148 = -t1142;
t1151 = -t1146;
t1153 = (t8.*t480.*t888)./2.0;
t1156 = (t2.*t480.*t892)./2.0;
t1185 = (t8.*t567.*t863)./2.0;
t1188 = (t2.*t569.*t863)./2.0;
t1190 = t15.*t491.*t914;
t1192 = t17.*t491.*t914;
t1235 = (t8.*t567.*t914)./2.0;
t1236 = (t2.*t569.*t914)./2.0;
t1245 = t15.*t763.*t774;
t1246 = t17.*t763.*t774;
t1261 = -t1260;
t1294 = t15.*t763.*t863;
t1295 = t17.*t763.*t863;
t1297 = t834+t840;
t1298 = t835+t841;
t1304 = t15.*t774.*t863;
t1306 = t17.*t774.*t863;
t1321 = (t8.*t763.*t887)./2.0;
t1323 = (t2.*t763.*t891)./2.0;
t1331 = t15.*t763.*t914;
t1332 = t17.*t763.*t914;
t1336 = t17.*t774.*t914;
t1337 = t15.*t774.*t914;
t1350 = (t8.*t818.*t914)./2.0;
t1351 = (t2.*t811.*t914)./2.0;
t1356 = (t8.*t863.*t887)./2.0;
t1358 = (t2.*t863.*t891)./2.0;
t1364 = t15.*t863.*t914;
t1365 = t17.*t863.*t914;
t1414 = t437+t449+t611+t733;
t1503 = t221+t349+t488+t498+t530+t619;
t1505 = t200+t339+t489+t499+t531+t626;
t314 = t12.*t293;
t315 = t6.*t295;
t316 = -t290;
t318 = t12.*t295;
t320 = -t291;
t328 = -t308;
t336 = -t319;
t362 = -t352;
t365 = t2.*t345;
t369 = -t356;
t394 = -t385;
t396 = t8.*t25.*t345;
t399 = t8.*t29.*t345;
t415 = t29.*t30.*t345;
t418 = -t397;
t419 = -t398;
t438 = -t411;
t452 = t232+t255;
t453 = t233+t256;
t467 = -t446;
t469 = -t451;
t471 = -t456;
t472 = -t457;
t476 = -t468;
t477 = t132.*t345;
t478 = -t470;
t484 = t171.*t345;
t519 = t278+t309;
t520 = (t12.*t25.*t400)./5.0e+3;
t521 = (t6.*t29.*t400)./5.0e+3;
t523 = (t12.*t29.*t400)./5.0e+3;
t524 = (t12.*t29.*t401)./5.0e+3;
t533 = (t12.*t25.*t400)./1.0e+4;
t534 = (t6.*t29.*t400)./1.0e+4;
t537 = (t12.*t29.*t401)./1.0e+4;
t544 = (t26.*t29.*t400)./5.0e+3;
t545 = (t29.*t30.*t400)./5.0e+3;
t550 = t8.*t512;
t560 = -t539;
t588 = (t132.*t400)./5.0e+3;
t589 = (t133.*t400)./5.0e+3;
t590 = (t132.*t401)./5.0e+3;
t597 = (t12.*t25.*t486)./5.0e+3;
t598 = (t6.*t29.*t486)./5.0e+3;
t599 = (t12.*t29.*t486)./5.0e+3;
t600 = (t171.*t400)./5.0e+3;
t601 = (t172.*t400)./5.0e+3;
t602 = (t172.*t401)./5.0e+3;
t607 = t249.*8.084033333333334e-4;
t613 = (t12.*t25.*t486)./1.0e+4;
t614 = (t6.*t29.*t486)./1.0e+4;
t616 = t252+t422;
t622 = (t26.*t29.*t486)./5.0e+3;
t624 = (t29.*t30.*t486)./5.0e+3;
t645 = t146.*t451.*(-1.0e-4);
t654 = t354+t383;
t675 = (t132.*t486)./5.0e+3;
t676 = (t133.*t486)./5.0e+3;
t679 = -t672;
t687 = (t171.*t486)./5.0e+3;
t688 = (t172.*t486)./5.0e+3;
t693 = -t691;
t697 = (t12.*t25.*t615)./5.0e+3;
t698 = (t6.*t29.*t615)./5.0e+3;
t699 = (t12.*t29.*t612)./5.0e+3;
t700 = (t12.*t29.*t615)./5.0e+3;
t709 = (t12.*t25.*t615)./1.0e+4;
t711 = t25.*t680;
t713 = t29.*t680;
t721 = (t26.*t29.*t615)./5.0e+3;
t724 = (t29.*t30.*t615)./5.0e+3;
t741 = t8.*t712;
t744 = t8.*t714;
t745 = -t714;
t752 = t2.*t729;
t754 = t12.*t39.*t345.*8.084033333333334e-4;
t756 = t2.*t732;
t758 = -t750;
t765 = (t12.*t29.*t674)./5.0e+3;
t767 = (t12.*t29.*t674)./1.0e+4;
t771 = (t132.*t612)./5.0e+3;
t772 = (t132.*t615)./5.0e+3;
t773 = (t133.*t615)./5.0e+3;
t777 = t428+t455;
t778 = t431+t458;
t785 = t6.*t25.*t401.*6.077704166666666e-4;
t786 = t6.*t25.*t401.*1.215540833333333e-3;
t787 = t6.*t29.*t400.*5.077704166666666e-4;
t788 = t6.*t29.*t400.*1.015540833333333e-3;
t789 = t6.*t29.*t401.*1.215540833333333e-3;
t790 = (t172.*t612)./5.0e+3;
t791 = t12.*t29.*t401.*5.077704166666666e-4;
t792 = t12.*t29.*t401.*1.015540833333333e-3;
t793 = (t171.*t615)./5.0e+3;
t794 = (t172.*t615)./5.0e+3;
t805 = -t796;
t807 = t24.*t29.*t401.*1.215540833333333e-3;
t808 = t27.*t29.*t401.*1.215540833333333e-3;
t810 = -t802;
t817 = t194.*t345.*8.084033333333334e-4;
t826 = t8.*t809;
t830 = t239.*t345.*8.084033333333334e-4;
t832 = t2.*t806;
t833 = (t132.*t674)./5.0e+3;
t850 = (t172.*t674)./5.0e+3;
t852 = -t837;
t855 = t133.*t400.*1.015540833333333e-3;
t856 = t132.*t401.*1.015540833333333e-3;
t857 = t133.*t401.*1.215540833333333e-3;
t861 = (t12.*t29.*t764)./5.0e+3;
t865 = t171.*t400.*1.015540833333333e-3;
t866 = t171.*t401.*1.215540833333333e-3;
t867 = t172.*t401.*1.015540833333333e-3;
t869 = (t12.*t29.*t764)./1.0e+4;
t880 = -t871;
t883 = -t875;
t884 = -t878;
t886 = t421+t576;
t906 = (t132.*t764)./5.0e+3;
t907 = t293+t386+t442;
t908 = t2.*t893;
t913 = (t172.*t764)./5.0e+3;
t915 = t515+t549;
t937 = t6.*t25.*t612.*6.077704166666666e-4;
t938 = t6.*t25.*t612.*1.215540833333333e-3;
t939 = t6.*t29.*t612.*1.215540833333333e-3;
t942 = -t924;
t945 = (t12.*t29.*t876)./5.0e+3;
t948 = t558+t564;
t950 = (t12.*t29.*t876)./1.0e+4;
t951 = t24.*t29.*t612.*1.215540833333333e-3;
t952 = t27.*t29.*t612.*1.215540833333333e-3;
t954 = t555+t563;
t955 = t556+t571;
t962 = t132.*t885;
t967 = t94+t157+t173+t680;
t971 = -t961;
Yr = ft_2({qd1,qd2,qd3,qd4,qd5,qd6,qrd1,qrd2,qrd3,qrd4,qrd5,qrd6,qrdd1,qrdd2,qrdd3,qrdd4,qrdd5,qrdd6,t1000,t1002,t1007,t101,t1012,t1013,t1019,t1028,t1029,t1033,t1037,t1038,t1039,t1041,t1045,t1050,t1052,t1054,t1077,t1079,t108,t1082,t1085,t1086,t1087,t1090,t1092,t1095,t1100,t1101,t1103,t1104,t111,t1119,t1120,t1122,t1123,t1140,t1141,t1142,t1146,t1148,t1151,t1153,t1156,t116,t1185,t1188,t1190,t1192,t12,t1235,t1236,t1245,t1246,t1259,t1260,t1261,t127,t1294,t1295,t1297,t1298,t13,t1304,t1306,t132,t1321,t1323,t133,t1331,t1332,t1336,t1337,t1350,t1351,t1356,t1358,t1364,t1365,t1414,t144,t15,t1503,t1505,t162,t169,t17,t170,t171,t172,t179,t18,t180,t183,t192,t194,t195,t2,t20,t200,t213,t214,t215,t216,t221,t222,t227,t229,t230,t231,t237,t238,t239,t24,t241,t243,t244,t245,t248,t25,t250,t251,t253,t254,t257,t258,t259,t26,t261,t263,t266,t267,t268,t269,t27,t270,t271,t272,t273,t276,t277,t279,t289,t29,t291,t294,t295,t296,t298,t3,t30,t301,t302,t304,t305,t31,t314,t315,t316,t318,t320,t321,t325,t326,t327,t328,t330,t331,t332,t333,t334,t336,t337,t338,t339,t341,t345,t346,t347,t348,t349,t35,t350,t351,t352,t353,t356,t357,t358,t36,t362,t363,t365,t366,t369,t370,t372,t373,t377,t378,t379,t380,t382,t385,t387,t388,t389,t39,t390,t392,t393,t394,t396,t399,t40,t403,t405,t408,t409,t410,t412,t414,t415,t416,t418,t419,t422,t423,t424,t426,t429,t430,t432,t433,t435,t436,t438,t439,t444,t445,t446,t447,t448,t450,t452,t453,t454,t456,t459,t460,t461,t463,t465,t466,t467,t469,t471,t472,t473,t474,t476,t477,t478,t480,t481,t482,t483,t484,t485,t487,t491,t493,t494,t495,t496,t497,t500,t503,t504,t505,t507,t513,t514,t517,t518,t519,t520,t521,t522,t523,t524,t526,t529,t533,t534,t537,t538,t542,t544,t545,t548,t550,t551,t552,t553,t554,t560,t561,t567,t568,t569,t570,t574,t575,t577,t578,t579,t580,t581,t586,t587,t588,t589,t590,t591,t592,t595,t596,t597,t598,t599,t6,t60,t600,t601,t602,t604,t606,t607,t609,t61,t610,t612,t613,t614,t615,t622,t624,t625,t629,t63,t630,t631,t632,t633,t636,t639,t640,t643,t644,t645,t646,t647,t648,t649,t651,t654,t656,t657,t659,t660,t661,t662,t663,t664,t665,t666,t667,t668,t669,t673,t675,t676,t677,t678,t679,t68,t683,t684,t687,t688,t689,t691,t692,t693,t694,t695,t696,t697,t698,t699,t7,t700,t702,t703,t704,t705,t706,t709,t71,t710,t711,t712,t713,t714,t715,t716,t719,t720,t721,t722,t723,t724,t726,t727,t728,t729,t731,t732,t734,t735,t736,t737,t738,t741,t742,t744,t745,t746,t747,t748,t749,t75,t751,t752,t753,t754,t755,t756,t757,t758,t759,t760,t761,t762,t763,t765,t766,t767,t768,t769,t771,t772,t773,t774,t775,t776,t777,t778,t781,t782,t783,t784,t785,t786,t787,t788,t789,t790,t791,t792,t793,t794,t795,t8,t801,t802,t803,t804,t805,t807,t808,t810,t811,t812,t813,t814,t815,t817,t818,t819,t820,t823,t824,t826,t827,t828,t829,t830,t831,t832,t833,t836,t838,t839,t843,t844,t845,t846,t848,t849,t850,t851,t852,t853,t854,t855,t856,t857,t858,t859,t860,t861,t863,t864,t865,t866,t867,t869,t870,t871,t872,t873,t875,t876,t877,t878,t879,t880,t881,t883,t884,t885,t886,t887,t888,t889,t890,t891,t892,t9,t90,t900,t901,t902,t903,t906,t907,t908,t909,t913,t914,t915,t919,t921,t922,t923,t925,t926,t927,t928,t929,t930,t931,t932,t933,t934,t935,t936,t937,t938,t939,t940,t941,t942,t945,t946,t948,t950,t951,t952,t954,t955,t960,t962,t966,t967,t968,t969,t970,t971,t976,t982,t983,t985,t990,t992,t993,t994});
end
function Yr = ft_2(ct)
qd1 = ct{1};
qd2 = ct{2};
qd3 = ct{3};
qd4 = ct{4};
qd5 = ct{5};
qd6 = ct{6};
qrd1 = ct{7};
qrd2 = ct{8};
qrd3 = ct{9};
qrd4 = ct{10};
qrd5 = ct{11};
qrd6 = ct{12};
qrdd1 = ct{13};
qrdd2 = ct{14};
qrdd3 = ct{15};
qrdd4 = ct{16};
qrdd5 = ct{17};
qrdd6 = ct{18};
t1000 = ct{19};
t1002 = ct{20};
t1007 = ct{21};
t101 = ct{22};
t1012 = ct{23};
t1013 = ct{24};
t1019 = ct{25};
t1028 = ct{26};
t1029 = ct{27};
t1033 = ct{28};
t1037 = ct{29};
t1038 = ct{30};
t1039 = ct{31};
t1041 = ct{32};
t1045 = ct{33};
t1050 = ct{34};
t1052 = ct{35};
t1054 = ct{36};
t1077 = ct{37};
t1079 = ct{38};
t108 = ct{39};
t1082 = ct{40};
t1085 = ct{41};
t1086 = ct{42};
t1087 = ct{43};
t1090 = ct{44};
t1092 = ct{45};
t1095 = ct{46};
t1100 = ct{47};
t1101 = ct{48};
t1103 = ct{49};
t1104 = ct{50};
t111 = ct{51};
t1119 = ct{52};
t1120 = ct{53};
t1122 = ct{54};
t1123 = ct{55};
t1140 = ct{56};
t1141 = ct{57};
t1142 = ct{58};
t1146 = ct{59};
t1148 = ct{60};
t1151 = ct{61};
t1153 = ct{62};
t1156 = ct{63};
t116 = ct{64};
t1185 = ct{65};
t1188 = ct{66};
t1190 = ct{67};
t1192 = ct{68};
t12 = ct{69};
t1235 = ct{70};
t1236 = ct{71};
t1245 = ct{72};
t1246 = ct{73};
t1259 = ct{74};
t1260 = ct{75};
t1261 = ct{76};
t127 = ct{77};
t1294 = ct{78};
t1295 = ct{79};
t1297 = ct{80};
t1298 = ct{81};
t13 = ct{82};
t1304 = ct{83};
t1306 = ct{84};
t132 = ct{85};
t1321 = ct{86};
t1323 = ct{87};
t133 = ct{88};
t1331 = ct{89};
t1332 = ct{90};
t1336 = ct{91};
t1337 = ct{92};
t1350 = ct{93};
t1351 = ct{94};
t1356 = ct{95};
t1358 = ct{96};
t1364 = ct{97};
t1365 = ct{98};
t1414 = ct{99};
t144 = ct{100};
t15 = ct{101};
t1503 = ct{102};
t1505 = ct{103};
t162 = ct{104};
t169 = ct{105};
t17 = ct{106};
t170 = ct{107};
t171 = ct{108};
t172 = ct{109};
t179 = ct{110};
t18 = ct{111};
t180 = ct{112};
t183 = ct{113};
t192 = ct{114};
t194 = ct{115};
t195 = ct{116};
t2 = ct{117};
t20 = ct{118};
t200 = ct{119};
t213 = ct{120};
t214 = ct{121};
t215 = ct{122};
t216 = ct{123};
t221 = ct{124};
t222 = ct{125};
t227 = ct{126};
t229 = ct{127};
t230 = ct{128};
t231 = ct{129};
t237 = ct{130};
t238 = ct{131};
t239 = ct{132};
t24 = ct{133};
t241 = ct{134};
t243 = ct{135};
t244 = ct{136};
t245 = ct{137};
t248 = ct{138};
t25 = ct{139};
t250 = ct{140};
t251 = ct{141};
t253 = ct{142};
t254 = ct{143};
t257 = ct{144};
t258 = ct{145};
t259 = ct{146};
t26 = ct{147};
t261 = ct{148};
t263 = ct{149};
t266 = ct{150};
t267 = ct{151};
t268 = ct{152};
t269 = ct{153};
t27 = ct{154};
t270 = ct{155};
t271 = ct{156};
t272 = ct{157};
t273 = ct{158};
t276 = ct{159};
t277 = ct{160};
t279 = ct{161};
t289 = ct{162};
t29 = ct{163};
t291 = ct{164};
t294 = ct{165};
t295 = ct{166};
t296 = ct{167};
t298 = ct{168};
t3 = ct{169};
t30 = ct{170};
t301 = ct{171};
t302 = ct{172};
t304 = ct{173};
t305 = ct{174};
t31 = ct{175};
t314 = ct{176};
t315 = ct{177};
t316 = ct{178};
t318 = ct{179};
t320 = ct{180};
t321 = ct{181};
t325 = ct{182};
t326 = ct{183};
t327 = ct{184};
t328 = ct{185};
t330 = ct{186};
t331 = ct{187};
t332 = ct{188};
t333 = ct{189};
t334 = ct{190};
t336 = ct{191};
t337 = ct{192};
t338 = ct{193};
t339 = ct{194};
t341 = ct{195};
t345 = ct{196};
t346 = ct{197};
t347 = ct{198};
t348 = ct{199};
t349 = ct{200};
t35 = ct{201};
t350 = ct{202};
t351 = ct{203};
t352 = ct{204};
t353 = ct{205};
t356 = ct{206};
t357 = ct{207};
t358 = ct{208};
t36 = ct{209};
t362 = ct{210};
t363 = ct{211};
t365 = ct{212};
t366 = ct{213};
t369 = ct{214};
t370 = ct{215};
t372 = ct{216};
t373 = ct{217};
t377 = ct{218};
t378 = ct{219};
t379 = ct{220};
t380 = ct{221};
t382 = ct{222};
t385 = ct{223};
t387 = ct{224};
t388 = ct{225};
t389 = ct{226};
t39 = ct{227};
t390 = ct{228};
t392 = ct{229};
t393 = ct{230};
t394 = ct{231};
t396 = ct{232};
t399 = ct{233};
t40 = ct{234};
t403 = ct{235};
t405 = ct{236};
t408 = ct{237};
t409 = ct{238};
t410 = ct{239};
t412 = ct{240};
t414 = ct{241};
t415 = ct{242};
t416 = ct{243};
t418 = ct{244};
t419 = ct{245};
t422 = ct{246};
t423 = ct{247};
t424 = ct{248};
t426 = ct{249};
t429 = ct{250};
t430 = ct{251};
t432 = ct{252};
t433 = ct{253};
t435 = ct{254};
t436 = ct{255};
t438 = ct{256};
t439 = ct{257};
t444 = ct{258};
t445 = ct{259};
t446 = ct{260};
t447 = ct{261};
t448 = ct{262};
t450 = ct{263};
t452 = ct{264};
t453 = ct{265};
t454 = ct{266};
t456 = ct{267};
t459 = ct{268};
t460 = ct{269};
t461 = ct{270};
t463 = ct{271};
t465 = ct{272};
t466 = ct{273};
t467 = ct{274};
t469 = ct{275};
t471 = ct{276};
t472 = ct{277};
t473 = ct{278};
t474 = ct{279};
t476 = ct{280};
t477 = ct{281};
t478 = ct{282};
t480 = ct{283};
t481 = ct{284};
t482 = ct{285};
t483 = ct{286};
t484 = ct{287};
t485 = ct{288};
t487 = ct{289};
t491 = ct{290};
t493 = ct{291};
t494 = ct{292};
t495 = ct{293};
t496 = ct{294};
t497 = ct{295};
t500 = ct{296};
t503 = ct{297};
t504 = ct{298};
t505 = ct{299};
t507 = ct{300};
t513 = ct{301};
t514 = ct{302};
t517 = ct{303};
t518 = ct{304};
t519 = ct{305};
t520 = ct{306};
t521 = ct{307};
t522 = ct{308};
t523 = ct{309};
t524 = ct{310};
t526 = ct{311};
t529 = ct{312};
t533 = ct{313};
t534 = ct{314};
t537 = ct{315};
t538 = ct{316};
t542 = ct{317};
t544 = ct{318};
t545 = ct{319};
t548 = ct{320};
t550 = ct{321};
t551 = ct{322};
t552 = ct{323};
t553 = ct{324};
t554 = ct{325};
t560 = ct{326};
t561 = ct{327};
t567 = ct{328};
t568 = ct{329};
t569 = ct{330};
t570 = ct{331};
t574 = ct{332};
t575 = ct{333};
t577 = ct{334};
t578 = ct{335};
t579 = ct{336};
t580 = ct{337};
t581 = ct{338};
t586 = ct{339};
t587 = ct{340};
t588 = ct{341};
t589 = ct{342};
t590 = ct{343};
t591 = ct{344};
t592 = ct{345};
t595 = ct{346};
t596 = ct{347};
t597 = ct{348};
t598 = ct{349};
t599 = ct{350};
t6 = ct{351};
t60 = ct{352};
t600 = ct{353};
t601 = ct{354};
t602 = ct{355};
t604 = ct{356};
t606 = ct{357};
t607 = ct{358};
t609 = ct{359};
t61 = ct{360};
t610 = ct{361};
t612 = ct{362};
t613 = ct{363};
t614 = ct{364};
t615 = ct{365};
t622 = ct{366};
t624 = ct{367};
t625 = ct{368};
t629 = ct{369};
t63 = ct{370};
t630 = ct{371};
t631 = ct{372};
t632 = ct{373};
t633 = ct{374};
t636 = ct{375};
t639 = ct{376};
t640 = ct{377};
t643 = ct{378};
t644 = ct{379};
t645 = ct{380};
t646 = ct{381};
t647 = ct{382};
t648 = ct{383};
t649 = ct{384};
t651 = ct{385};
t654 = ct{386};
t656 = ct{387};
t657 = ct{388};
t659 = ct{389};
t660 = ct{390};
t661 = ct{391};
t662 = ct{392};
t663 = ct{393};
t664 = ct{394};
t665 = ct{395};
t666 = ct{396};
t667 = ct{397};
t668 = ct{398};
t669 = ct{399};
t673 = ct{400};
t675 = ct{401};
t676 = ct{402};
t677 = ct{403};
t678 = ct{404};
t679 = ct{405};
t68 = ct{406};
t683 = ct{407};
t684 = ct{408};
t687 = ct{409};
t688 = ct{410};
t689 = ct{411};
t691 = ct{412};
t692 = ct{413};
t693 = ct{414};
t694 = ct{415};
t695 = ct{416};
t696 = ct{417};
t697 = ct{418};
t698 = ct{419};
t699 = ct{420};
t7 = ct{421};
t700 = ct{422};
t702 = ct{423};
t703 = ct{424};
t704 = ct{425};
t705 = ct{426};
t706 = ct{427};
t709 = ct{428};
t71 = ct{429};
t710 = ct{430};
t711 = ct{431};
t712 = ct{432};
t713 = ct{433};
t714 = ct{434};
t715 = ct{435};
t716 = ct{436};
t719 = ct{437};
t720 = ct{438};
t721 = ct{439};
t722 = ct{440};
t723 = ct{441};
t724 = ct{442};
t726 = ct{443};
t727 = ct{444};
t728 = ct{445};
t729 = ct{446};
t731 = ct{447};
t732 = ct{448};
t734 = ct{449};
t735 = ct{450};
t736 = ct{451};
t737 = ct{452};
t738 = ct{453};
t741 = ct{454};
t742 = ct{455};
t744 = ct{456};
t745 = ct{457};
t746 = ct{458};
t747 = ct{459};
t748 = ct{460};
t749 = ct{461};
t75 = ct{462};
t751 = ct{463};
t752 = ct{464};
t753 = ct{465};
t754 = ct{466};
t755 = ct{467};
t756 = ct{468};
t757 = ct{469};
t758 = ct{470};
t759 = ct{471};
t760 = ct{472};
t761 = ct{473};
t762 = ct{474};
t763 = ct{475};
t765 = ct{476};
t766 = ct{477};
t767 = ct{478};
t768 = ct{479};
t769 = ct{480};
t771 = ct{481};
t772 = ct{482};
t773 = ct{483};
t774 = ct{484};
t775 = ct{485};
t776 = ct{486};
t777 = ct{487};
t778 = ct{488};
t781 = ct{489};
t782 = ct{490};
t783 = ct{491};
t784 = ct{492};
t785 = ct{493};
t786 = ct{494};
t787 = ct{495};
t788 = ct{496};
t789 = ct{497};
t790 = ct{498};
t791 = ct{499};
t792 = ct{500};
t793 = ct{501};
t794 = ct{502};
t795 = ct{503};
t8 = ct{504};
t801 = ct{505};
t802 = ct{506};
t803 = ct{507};
t804 = ct{508};
t805 = ct{509};
t807 = ct{510};
t808 = ct{511};
t810 = ct{512};
t811 = ct{513};
t812 = ct{514};
t813 = ct{515};
t814 = ct{516};
t815 = ct{517};
t817 = ct{518};
t818 = ct{519};
t819 = ct{520};
t820 = ct{521};
t823 = ct{522};
t824 = ct{523};
t826 = ct{524};
t827 = ct{525};
t828 = ct{526};
t829 = ct{527};
t830 = ct{528};
t831 = ct{529};
t832 = ct{530};
t833 = ct{531};
t836 = ct{532};
t838 = ct{533};
t839 = ct{534};
t843 = ct{535};
t844 = ct{536};
t845 = ct{537};
t846 = ct{538};
t848 = ct{539};
t849 = ct{540};
t850 = ct{541};
t851 = ct{542};
t852 = ct{543};
t853 = ct{544};
t854 = ct{545};
t855 = ct{546};
t856 = ct{547};
t857 = ct{548};
t858 = ct{549};
t859 = ct{550};
t860 = ct{551};
t861 = ct{552};
t863 = ct{553};
t864 = ct{554};
t865 = ct{555};
t866 = ct{556};
t867 = ct{557};
t869 = ct{558};
t870 = ct{559};
t871 = ct{560};
t872 = ct{561};
t873 = ct{562};
t875 = ct{563};
t876 = ct{564};
t877 = ct{565};
t878 = ct{566};
t879 = ct{567};
t880 = ct{568};
t881 = ct{569};
t883 = ct{570};
t884 = ct{571};
t885 = ct{572};
t886 = ct{573};
t887 = ct{574};
t888 = ct{575};
t889 = ct{576};
t890 = ct{577};
t891 = ct{578};
t892 = ct{579};
t9 = ct{580};
t90 = ct{581};
t900 = ct{582};
t901 = ct{583};
t902 = ct{584};
t903 = ct{585};
t906 = ct{586};
t907 = ct{587};
t908 = ct{588};
t909 = ct{589};
t913 = ct{590};
t914 = ct{591};
t915 = ct{592};
t919 = ct{593};
t921 = ct{594};
t922 = ct{595};
t923 = ct{596};
t925 = ct{597};
t926 = ct{598};
t927 = ct{599};
t928 = ct{600};
t929 = ct{601};
t930 = ct{602};
t931 = ct{603};
t932 = ct{604};
t933 = ct{605};
t934 = ct{606};
t935 = ct{607};
t936 = ct{608};
t937 = ct{609};
t938 = ct{610};
t939 = ct{611};
t940 = ct{612};
t941 = ct{613};
t942 = ct{614};
t945 = ct{615};
t946 = ct{616};
t948 = ct{617};
t950 = ct{618};
t951 = ct{619};
t952 = ct{620};
t954 = ct{621};
t955 = ct{622};
t960 = ct{623};
t962 = ct{624};
t966 = ct{625};
t967 = ct{626};
t968 = ct{627};
t969 = ct{628};
t970 = ct{629};
t971 = ct{630};
t976 = ct{631};
t982 = ct{632};
t983 = ct{633};
t985 = ct{634};
t990 = ct{635};
t992 = ct{636};
t993 = ct{637};
t994 = ct{638};
t978 = t172.*t885;
t979 = t132.*t612.*1.015540833333333e-3;
t980 = t133.*t612.*1.215540833333333e-3;
t981 = t133.*t615.*1.015540833333333e-3;
t984 = -t969;
t989 = t2.*t968;
t991 = (t132.*t876)./5.0e+3;
t995 = t171.*t612.*1.215540833333333e-3;
t996 = t172.*t612.*1.015540833333333e-3;
t997 = t171.*t615.*1.015540833333333e-3;
t998 = t450+t712;
t999 = t8.*t976;
t1004 = (t172.*t876)./5.0e+3;
t1006 = -t1000;
t1015 = -t1012;
t1022 = -t1019;
t1031 = t194.*t660.*8.084033333333334e-4;
t1046 = t606+t640;
t1049 = t90+t968;
t1051 = t75+t976;
t1053 = t238.*t661.*8.084033333333334e-4;
t1057 = t2.*t1037;
t1058 = t2.*t1038;
t1059 = t625+t636;
t1061 = t8.*t1028;
t1062 = t8.*t1029;
t1073 = t8.*t1052;
t1076 = t644+t651;
t1083 = t656+t669;
t1088 = -t1082;
t1089 = t327.*t661.*8.084033333333334e-4;
t1096 = t29.*t111.*t990;
t1097 = -t1090;
t1098 = t660.*(t60-t192).*(-8.084033333333334e-4);
t1099 = t345.*t660.*8.084033333333334e-4;
t1102 = -t29.*t116.*(t426-t712);
t1105 = -t1092;
t1107 = -t1100;
t1110 = -t1104;
t1111 = t661.*(t61-t241).*(-8.084033333333334e-4);
t1113 = t677+t678;
t1116 = t6.*t29.*t873.*6.077704166666666e-4;
t1117 = t6.*t29.*t873.*1.215540833333333e-3;
t1121 = -t1119;
t1124 = -t1120;
t1126 = t24.*t29.*t1052.*2.8925e-2;
t1135 = t2.*t1123;
t1136 = t8.*t1122;
t1154 = t1140./2.0;
t1155 = t1141./2.0;
t1157 = t133.*t873.*1.215540833333333e-3;
t1161 = -t1156;
t1164 = t2.*t363.*t990;
t1166 = t305+t1052;
t1168 = t169+t665+t673;
t1170 = t171.*t873.*1.215540833333333e-3;
t1171 = -t8.*t363.*(t426-t712);
t1172 = t2.*t370.*t990;
t1173 = -t8.*t370.*(t426-t712);
t1176 = (t2.*t25.*t1122)./2.0;
t1177 = (t8.*t25.*t1123)./2.0;
t1183 = t8.*t370.*(t426-t712);
t1189 = t461+t960;
t1193 = -t1185;
t1194 = -t1188;
t1197 = t737+t759;
t1207 = t1190./2.0;
t1209 = t1192./2.0;
t1221 = t382.*t1052;
t1223 = t2.*t363.*t1052;
t1228 = t2.*t370.*t1052;
t1234 = t729+t823;
t1237 = t2.*t480.*t990;
t1240 = -t1235;
t1241 = -t1236;
t1242 = -t8.*t480.*(t426-t712);
t1243 = t2.*t481.*t990;
t1244 = -t8.*t481.*(t426-t712);
t1257 = t405.*t1085;
t1263 = t2.*t480.*t1052;
t1264 = t244+t747+t749;
t1265 = t2.*t574.*t990;
t1268 = (t570.*t990)./2.0;
t1269 = -t8.*t574.*(t426-t712);
t1273 = t2.*t481.*t1052;
t1274 = t568.*(t426-t712).*(-1.0./2.0);
t1303 = t15.*t763.*t879;
t1305 = t17.*t763.*t879;
t1308 = t570.*t1052;
t1312 = t844+t846;
t1320 = t2.*t574.*t1052;
t1326 = -t1323;
t1342 = t380.*(t429-t960).*(-1.0./2.0);
t1344 = t15.*t863.*t879;
t1346 = t17.*t863.*t879;
t1349 = t372.*(t446-t970).*(-1.0./2.0);
t1352 = -t1350;
t1354 = -t1351;
t1362 = -t1358;
t1366 = t900+t902;
t1367 = t901+t903;
t1368 = t17.*t879.*t914;
t1369 = t15.*t879.*t914;
t1370 = t341+t815+t824;
t1372 = (t812.*t990)./2.0;
t1378 = t819.*(t426-t712).*(-1.0./2.0);
t1379 = t2.*t491.*(t429-t960).*(-1.0./2.0);
t1385 = t8.*t491.*(t446-t970).*(-1.0./2.0);
t1388 = t812.*t1052;
t1391 = t925+t928;
t1392 = t926+t930;
t1393 = t927+t931;
t1394 = t569.*(t429-t960).*(-1.0./2.0);
t1397 = (t569.*(t429-t960))./2.0;
t1403 = t567.*(t446-t970).*(-1.0./2.0);
t1407 = (t567.*(t446-t970))./2.0;
t1408 = (t892.*t990)./2.0;
t1413 = t888.*(t426-t712).*(-1.0./2.0);
t1422 = t892.*t1052;
t1435 = t487+t843+t851;
t1438 = t982+t983;
t1453 = t919.*t1085;
t1454 = -t2.*t763.*(t429-t960);
t1457 = -t2.*t774.*(t429-t960);
t1461 = -t8.*t763.*(t446-t970);
t1462 = -t8.*t774.*(t446-t970);
t1463 = t990.*t1052;
t1469 = t811.*(t429-t960).*(-1.0./2.0);
t1470 = (t811.*(t429-t960))./2.0;
t1474 = t818.*(t446-t970).*(-1.0./2.0);
t1476 = t238.*(-t269-t295+t352+t356+t385+t8.*t25.*(t61-t241)).*(-4.042016666666667e-4);
t1477 = t238.*(-t269-t295+t352+t356+t385+t8.*t25.*(t61-t241)).*(-8.084033333333334e-4);
t1479 = (t818.*(t446-t970))./2.0;
t1483 = -t2.*t863.*(t429-t960);
t1484 = -t2.*t879.*(t429-t960);
t1488 = -t8.*t863.*(t446-t970);
t1494 = -t8.*t879.*(t446-t970);
t1495 = t327.*(-t269-t295+t352+t356+t385+t8.*t25.*(t61-t241)).*(-8.084033333333334e-4);
t1497 = t891.*(t429-t960).*(-1.0./2.0);
t1498 = t327.*(-t269-t295+t352+t356+t385+t8.*t25.*(t61-t241)).*8.084033333333334e-4;
t1499 = (t2.*t363.*t1414)./2.0;
t1500 = (t891.*(t429-t960))./2.0;
t1501 = t8.*t363.*(t424-t435-t609+t714).*(-1.0./2.0);
t1504 = (t8.*t363.*(t424-t435-t609+t714))./2.0;
t1506 = t887.*(t446-t970).*(-1.0./2.0);
t1510 = (t887.*(t446-t970))./2.0;
t1511 = (t61-t241).*(-t269-t295+t352+t356+t385+t8.*t25.*(t61-t241)).*8.084033333333334e-4;
t1513 = -t2.*t914.*(t429-t960);
t1515 = t8.*t1503;
t1516 = t2.*t1505;
t1525 = -t8.*t914.*(t446-t970);
t1537 = (t2.*t29.*t1503)./2.0;
t1538 = (t8.*t29.*t1505)./2.0;
t1542 = (t2.*t480.*t1414)./2.0;
t1543 = t8.*t480.*(t424-t435-t609+t714).*(-1.0./2.0);
t1545 = (t8.*t480.*(t424-t435-t609+t714))./2.0;
t1558 = (t2.*t574.*t1414)./2.0;
t1561 = t8.*t574.*(t424-t435-t609+t714).*(-1.0./2.0);
t1568 = (t8.*t574.*(t424-t435-t609+t714))./2.0;
t1579 = t487+t1033+t1045;
t1600 = t659+t662+t845+t848;
t1628 = t990.*t1414;
t1635 = (t426-t712).*(t424-t435-t609+t714);
t1654 = (t1052.*t1414)./2.0;
t1658 = t2.*t763.*(t444-t445-t639+t969).*(-1.0./2.0);
t1671 = t2.*t863.*(t444-t445-t639+t969).*(-1.0./2.0);
t1676 = t333+t350+t727+t742+t751+t755;
t1685 = t8.*(t326-t350+t726-t727-t755+t12.*t39.*(t60-t192).*8.084033333333334e-4).*(-1.0./2.0);
t1687 = t2.*t914.*(t444-t445-t639+t969).*(-1.0./2.0);
t1691 = (t8.*(t326-t350+t726-t727-t755+t12.*t39.*(t60-t192).*8.084033333333334e-4))./2.0;
t1712 = t172.*(t326-t350+t726-t727-t755+t12.*t39.*(t60-t192).*8.084033333333334e-4).*(-1.0./2.0);
t1777 = (t429-t960).*(t444-t445-t639+t969);
t1831 = t941+t946+t1039+t1054;
t1836 = -qd1.*(t940-t941+t1041+t1050);
t417 = -t396;
t502 = -t484;
t532 = -t520;
t535 = -t523;
t536 = -t524;
t546 = -t533;
t547 = -t537;
t557 = -t544;
t559 = -t545;
t562 = t304+t328;
t566 = -t550;
t593 = -t589;
t594 = -t590;
t617 = -t600;
t618 = -t602;
t637 = -t624;
t655 = t365+t366;
t682 = -t676;
t690 = -t687;
t708 = -t697;
t717 = t388+t418;
t718 = t389+t419;
t725 = -t709;
t740 = t8.*t711;
t743 = t8.*t713;
t779 = -t772;
t780 = -t773;
t797 = t436+t469;
t798 = -t792;
t799 = -t791;
t800 = -t793;
t825 = -t817;
t842 = -t830;
t868 = -t861;
t874 = -t869;
t894 = t194.*t452.*4.042016666666667e-4;
t895 = t194.*t452.*8.084033333333334e-4;
t896 = t268+t399+t414;
t904 = t238.*t453.*4.042016666666667e-4;
t905 = t238.*t453.*8.084033333333334e-4;
t910 = -t906;
t918 = -t908;
t920 = -t913;
t943 = t194.*t519.*4.042016666666667e-4;
t944 = t194.*t519.*8.084033333333334e-4;
t949 = -t945;
t953 = t327.*t453.*8.084033333333334e-4;
t956 = -t950;
t957 = t452.*(t60-t192).*(-8.084033333333334e-4);
t958 = t345.*t452.*8.084033333333334e-4;
t959 = qd3.*t954;
t963 = t453.*(t61-t241).*(-8.084033333333334e-4);
t974 = t12.*t40.*t654.*4.042016666666667e-4;
t975 = t12.*t40.*t654.*8.084033333333334e-4;
t986 = -t980;
t987 = -t981;
t988 = t2.*t967;
t1001 = -t991;
t1003 = -t997;
t1005 = -t999;
t1008 = t519.*(t60-t192).*(-8.084033333333334e-4);
t1009 = t318+t474+t485;
t1010 = t320+t477+t482;
t1011 = t345.*t519.*8.084033333333334e-4;
t1014 = t519.*(t60-t192).*8.084033333333334e-4;
t1018 = t13.*t132.*t654.*8.084033333333334e-4;
t1023 = t195.*t654.*4.042016666666667e-4;
t1024 = t195.*t654.*8.084033333333334e-4;
t1032 = t13.*t172.*t654.*8.084033333333334e-4;
t1040 = -t1031;
t1042 = t238.*t654.*8.084033333333334e-4;
t1048 = t90+t967;
t1067 = t629+t645;
t1069 = t2.*t1049;
t1070 = t271.*t654.*8.084033333333334e-4;
t1071 = t272.*t654.*8.084033333333334e-4;
t1072 = t8.*t1051;
t1075 = -t1073;
t1078 = (t8.*t1046)./2.0;
t1084 = t327.*t654.*8.084033333333334e-4;
t1091 = qd1.*t1083;
t1106 = t654.*(t61-t241).*(-8.084033333333334e-4);
t1112 = t162+t591+t607;
t1118 = -t25.*(t523-t789);
t1125 = t27.*t29.*t1049.*2.8925e-2;
t1127 = t25.*(t520-t786).*(-1.0./2.0);
t1129 = t29.*(t523-t789).*(-1.0./2.0);
t1131 = -t1126;
t1132 = (t25.*(t520-t786))./2.0;
t1133 = t8.*(t544-t807).*(-1.0./2.0);
t1134 = t2.*(t545-t808).*(-1.0./2.0);
t1138 = (t8.*(t544-t807))./2.0;
t1139 = (t2.*(t545-t808))./2.0;
t1147 = -t1136;
t1152 = t12.*t40.*t907.*8.084033333333334e-4;
t1159 = t296+t1049;
t1160 = t2.*t29.*(t544-t807).*(-1.0./2.0);
t1162 = t8.*t29.*(t545-t808).*(-1.0./2.0);
t1163 = -t1157;
t1165 = t305+t1051;
t1167 = (t2.*t29.*(t544-t807))./2.0;
t1169 = (t8.*t29.*(t545-t808))./2.0;
t1178 = t588+t866;
t1179 = t601+t857;
t1180 = -t1172;
t1182 = t8.*t1166;
t1184 = t738+t758;
t1187 = t744+t757;
t1204 = t13.*t132.*t907.*8.084033333333334e-4;
t1205 = t467+t970;
t1206 = t378+t387+t473+t478;
t1210 = t195.*t907.*4.042016666666667e-4;
t1211 = t195.*t907.*8.084033333333334e-4;
t1214 = t13.*t172.*t907.*8.084033333333334e-4;
t1216 = t373.*t1049;
t1219 = t238.*t907.*8.084033333333334e-4;
t1220 = t380.*t1051;
t1222 = t8.*t363.*t1049;
t1224 = (t12.*t29.*t1168)./2.0;
t1227 = t8.*t370.*t1049;
t1230 = t271.*t907.*8.084033333333334e-4;
t1231 = t272.*t907.*8.084033333333334e-4;
t1238 = t711+t839;
t1247 = t12.*t39.*(t291-t477+t172.*(t60-t192)).*(-4.042016666666667e-4);
t1248 = t12.*t39.*(t291-t477+t172.*(t60-t192)).*(-8.084033333333334e-4);
t1251 = t327.*t907.*8.084033333333334e-4;
t1258 = t907.*(t61-t241).*(-8.084033333333334e-4);
t1262 = -t1257;
t1266 = t1257./2.0;
t1267 = t8.*t480.*t1049;
t1272 = t8.*t481.*t1049;
t1275 = t7.*t132.*(t291-t477+t172.*(t60-t192)).*(-8.084033333333334e-4);
t1276 = -t1268;
t1279 = t101+t229+t250+t315+t476+t522;
t1280 = t194.*(t291-t477+t172.*(t60-t192)).*(-8.084033333333334e-4);
t1283 = t826+t832;
t1284 = t7.*t172.*(t291-t477+t172.*(t60-t192)).*(-8.084033333333334e-4);
t1287 = t194.*(t291-t477+t172.*(t60-t192)).*8.084033333333334e-4;
t1292 = t239.*(t291-t477+t172.*(t60-t192)).*(-4.042016666666667e-4);
t1293 = t239.*(t291-t477+t172.*(t60-t192)).*(-8.084033333333334e-4);
t1296 = (t2.*t491.*t1051)./2.0;
t1301 = t251.*(t291-t477+t172.*(t60-t192)).*(-8.084033333333334e-4);
t1302 = t254.*(t291-t477+t172.*(t60-t192)).*(-8.084033333333334e-4);
t1307 = t569.*t1051;
t1309 = t251.*(t291-t477+t172.*(t60-t192)).*8.084033333333334e-4;
t1311 = t568.*t1049;
t1316 = (t25.*t1264)./2.0;
t1317 = t8.*t574.*t1049;
t1318 = -t1308;
t1325 = (t12.*t29.*t1264)./2.0;
t1329 = t855+t867;
t1330 = t856+t865;
t1333 = (t60-t192).*(t291-t477+t172.*(t60-t192)).*8.084033333333334e-4;
t1334 = t345.*(t291-t477+t172.*(t60-t192)).*(-8.084033333333334e-4);
t1335 = t269+t295+t362+t369+t394+t416;
t1348 = t405.*t1197;
t1371 = t505+t526+t538+t560;
t1375 = -t1372;
t1377 = t8.*t1370;
t1381 = t2.*t763.*t1051;
t1382 = -t2.*(t332+t817+t238.*(t61-t241).*8.084033333333334e-4);
t1384 = t2.*t774.*t1051;
t1386 = t289+t336+t410+t412+t415+t439;
t1387 = t811.*t1051;
t1390 = t819.*t1049;
t1395 = -t1388;
t1398 = (t2.*t25.*t1370)./2.0;
t1399 = t314+t321+t392+t433+t438+t463;
t1400 = t2.*t491.*t1234;
t1404 = (t26.*t29.*t1370)./2.0;
t1406 = t8.*t25.*(t332+t817+t238.*(t61-t241).*8.084033333333334e-4).*(-1.0./2.0);
t1411 = -t1408;
t1412 = t29.*t30.*(t332+t817+t238.*(t61-t241).*8.084033333333334e-4).*(-1.0./2.0);
t1415 = t435+t448+t609+t745;
t1417 = t2.*t863.*t1051;
t1418 = (t569.*t1234)./2.0;
t1419 = (t133.*t1370)./2.0;
t1420 = (t915.*t993)./2.0;
t1421 = t891.*t1051;
t1426 = t888.*t1049;
t1427 = t2.*t879.*t1051;
t1431 = -t1422;
t1433 = t171.*(t332+t817+t238.*(t61-t241).*8.084033333333334e-4).*(-1.0./2.0);
t1434 = (t171.*(t332+t817+t238.*(t61-t241).*8.084033333333334e-4))./2.0;
t1439 = t2.*t914.*t1051;
t1440 = qd1.*t1435;
t1452 = t989+t1006;
t1455 = -t1453;
t1458 = t8.*(t981-t996).*(-1.0./2.0);
t1460 = (t8.*(t981-t996))./2.0;
t1464 = t194.*(-t270-t294+t334+t337+t396+t2.*t25.*(t60-t192)).*(-4.042016666666667e-4);
t1465 = t194.*(-t270-t294+t334+t337+t396+t2.*t25.*(t60-t192)).*(-8.084033333333334e-4);
t1466 = -t1049.*(t426-t712);
t1468 = -t405.*(t908-t909);
t1473 = t2.*t763.*t1234;
t1481 = t2.*t774.*t1234;
t1485 = t1057+t1061;
t1486 = t1058+t1062;
t1487 = (t811.*t1234)./2.0;
t1489 = (t60-t192).*(-t270-t294+t334+t337+t396+t2.*t25.*(t60-t192)).*8.084033333333334e-4;
t1490 = t345.*(-t270-t294+t334+t337+t396+t2.*t25.*(t60-t192)).*(-8.084033333333334e-4);
t1491 = t700+t705+t939;
t1492 = t345.*(-t270-t294+t334+t337+t396+t2.*t25.*(t60-t192)).*8.084033333333334e-4;
t1502 = -t1499;
t1512 = t919.*t1197;
t1514 = t2.*t863.*t1234;
t1518 = t915.*(t387+t473+t478+t26.*t29.*t132.*1.383e-1);
t1520 = t2.*t879.*t1234;
t1521 = t445+t466+t639+t984;
t1522 = t430+t472+t649+t971;
t1523 = -t1515;
t1524 = -t1516;
t1528 = t1515./2.0;
t1529 = t1516./2.0;
t1531 = (t891.*t1234)./2.0;
t1539 = t2.*t914.*t1234;
t1544 = -t1542;
t1563 = -t1051.*(t429-t960);
t1564 = -t1558;
t1567 = t632+t648+t741+t753;
t1569 = t915.*t1297;
t1571 = t259+t465+t942+t962;
t1574 = t273+t471+t922+t978;
t1576 = t1085.*t1197;
t1577 = t1051.*t1234;
t1580 = (t1113.*t1197)./2.0;
t1582 = qd1.*t1579;
t1597 = -t919.*(t908-t909);
t1608 = t633+t713+t820+t836;
t1612 = t610+t732+t838+t852;
t1614 = t487+t1095+t1105;
t1615 = (t915.*t1392)./2.0;
t1616 = -t1234.*(t429-t960);
t1634 = -t1628;
t1641 = -t1085.*(t908-t909);
t1645 = t1085.*(t908-t909);
t1650 = -t1113.*(t908-t909);
t1656 = -t1654;
t1657 = t1049.*(t424-t435-t609+t714).*(-1.0./2.0);
t1673 = -t1197.*(t908-t909);
t1675 = t1197.*(t908-t909);
t1677 = t330+t351+t710+t728+t754+t762;
t1693 = t8.*t763.*(t263+t456-t922-t978).*(-1.0./2.0);
t1695 = (t8.*t763.*(t263+t456-t922-t978))./2.0;
t1698 = t858+t870+t875+t884;
t1705 = t221+t349+t760+t768+t805+t829;
t1711 = t8.*t863.*(t263+t456-t922-t978).*(-1.0./2.0);
t1716 = (t8.*t863.*(t263+t456-t922-t978))./2.0;
t1733 = t1051.*(t444-t445-t639+t969).*(-1.0./2.0);
t1735 = (t1051.*(t444-t445-t639+t969))./2.0;
t1740 = t8.*t914.*(t263+t456-t922-t978).*(-1.0./2.0);
t1811 = (t446-t970).*(t263+t456-t922-t978);
t1867 = t985+t1002+t1100+t1110;
t1921 = t697+t715+t814+t938+t945+t1117;
t1922 = t858+t870+t878+t883+t933+t934;
t1930 = t1142+t1151+t1153+t1161;
t1956 = t1188+t1193+t1259+t1261;
t1957 = -qd1.*(t1185+t1194-t1259+t1260);
t1960 = t1236+t1240+t1321+t1326;
t1961 = -qd1.*(t1235+t1241-t1321+t1323);
t1966 = t1351+t1352+t1356+t1362;
t1967 = -qd1.*(t1350+t1354-t1356+t1358);
t897 = -t895;
t898 = -t894;
t947 = t548+t566;
t964 = t238.*t562.*4.042016666666667e-4;
t965 = t238.*t562.*8.084033333333334e-4;
t972 = t12.*t39.*t655.*4.042016666666667e-4;
t973 = t12.*t39.*t655.*8.084033333333334e-4;
t1016 = t390.*t797;
t1017 = t7.*t132.*t655.*8.084033333333334e-4;
t1020 = t327.*t562.*8.084033333333334e-4;
t1025 = t194.*t655.*8.084033333333334e-4;
t1030 = t7.*t172.*t655.*8.084033333333334e-4;
t1034 = -t1024;
t1035 = -t1023;
t1043 = t239.*t655.*4.042016666666667e-4;
t1044 = t239.*t655.*8.084033333333334e-4;
t1055 = t562.*(t61-t241).*(-8.084033333333334e-4);
t1056 = -t1042;
t1060 = t251.*t655.*8.084033333333334e-4;
t1063 = t254.*t655.*8.084033333333334e-4;
t1064 = t562.*(t61-t241).*8.084033333333334e-4;
t1068 = t2.*t1048;
t1074 = -t1072;
t1081 = -t1078;
t1093 = t655.*(t60-t192).*(-8.084033333333334e-4);
t1094 = t345.*t655.*8.084033333333334e-4;
t1108 = t532+t786;
t1109 = t535+t789;
t1114 = t557+t807;
t1115 = t559+t808;
t1130 = -t1125;
t1137 = (t29.*t1112)./2.0;
t1143 = t12.*t39.*t896.*8.084033333333334e-4;
t1144 = (t12.*t25.*t1112)./2.0;
t1158 = t296+t1048;
t1175 = t2.*t1159;
t1181 = t8.*t1165;
t1186 = t743+t756;
t1191 = t7.*t132.*t896.*8.084033333333334e-4;
t1196 = -t1182;
t1199 = t2.*t1178;
t1200 = qd1.*t1184;
t1201 = t8.*t1179;
t1202 = t194.*t896.*8.084033333333334e-4;
t1203 = t7.*t172.*t896.*8.084033333333334e-4;
t1212 = t239.*t896.*4.042016666666667e-4;
t1213 = t239.*t896.*8.084033333333334e-4;
t1215 = t372.*t1048;
t1217 = t251.*t896.*8.084033333333334e-4;
t1218 = t254.*t896.*8.084033333333334e-4;
t1225 = t2.*t29.*t1179;
t1226 = t8.*t29.*t1178;
t1232 = (t2.*t25.*t1179)./2.0;
t1233 = (t8.*t25.*t1178)./2.0;
t1249 = t12.*t40.*t1009.*4.042016666666667e-4;
t1250 = t12.*t40.*t1009.*8.084033333333334e-4;
t1252 = t896.*(t60-t192).*(-8.084033333333334e-4);
t1253 = t345.*t896.*8.084033333333334e-4;
t1254 = t896.*(t60-t192).*8.084033333333334e-4;
t1255 = t788+t798;
t1271 = -t1266;
t1277 = t13.*t132.*t1009.*8.084033333333334e-4;
t1278 = t108+t227+t248+t316+t483+t502;
t1281 = t195.*t1009.*4.042016666666667e-4;
Yr = ft_3({qd1,qd2,qd3,qd4,qd5,qd6,qrd1,qrd2,qrd3,qrd4,qrd5,qrd6,qrdd1,qrdd2,qrdd3,qrdd4,qrdd5,qrdd6,t1001,t1002,t1003,t1004,t1005,t1007,t1009,t1011,t1012,t1013,t1014,t1015,t1016,t1017,t1018,t1019,t1020,t1022,t1025,t1030,t1032,t1034,t1035,t1040,t1041,t1042,t1043,t1044,t1046,t1048,t1049,t1050,t1051,t1052,t1053,t1056,t1059,t1060,t1063,t1064,t1067,t1068,t1069,t1070,t1071,t1074,t1075,t1076,t1077,t1078,t1079,t1082,t1083,t1084,t1085,t1086,t1087,t1088,t1089,t1090,t1091,t1093,t1094,t1096,t1097,t1098,t1099,t1101,t1102,t1103,t1104,t1106,t1107,t1109,t1111,t1112,t1113,t1116,t1118,t1119,t1120,t1121,t1122,t1123,t1124,t1125,t1126,t1129,t1130,t1131,t1132,t1133,t1134,t1135,t1137,t1138,t1139,t1140,t1141,t1143,t1144,t1146,t1147,t1148,t1152,t1153,t1154,t1155,t1156,t1158,t1161,t1163,t1164,t1167,t1168,t1169,t1170,t1171,t1175,t1176,t1177,t1180,t1181,t1183,t1184,t1185,t1186,t1187,t1190,t1191,t1192,t1194,t1196,t1197,t1199,t12,t1200,t1201,t1202,t1203,t1204,t1207,t1209,t1210,t1211,t1212,t1213,t1214,t1215,t1216,t1217,t1218,t1219,t1220,t1221,t1222,t1223,t1224,t1225,t1226,t1227,t1228,t1230,t1231,t1232,t1233,t1234,t1235,t1237,t1238,t1241,t1242,t1243,t1244,t1245,t1246,t1247,t1248,t1249,t1250,t1251,t1253,t1254,t1255,t1257,t1258,t1259,t1260,t1261,t1262,t1263,t1265,t1266,t1267,t1268,t1269,t127,t1271,t1272,t1273,t1274,t1275,t1276,t1277,t1278,t1279,t1281,t1283,t1284,t1287,t1292,t1293,t1294,t1295,t1296,t1297,t1298,t13,t1302,t1303,t1304,t1305,t1306,t1307,t1309,t1311,t1312,t1316,t1317,t1318,t132,t1320,t1321,t1323,t1325,t1326,t1329,t133,t1330,t1331,t1332,t1333,t1334,t1336,t1337,t1342,t1344,t1346,t1348,t1349,t1350,t1354,t1356,t1358,t1362,t1364,t1365,t1366,t1367,t1368,t1369,t1370,t1371,t1372,t1375,t1377,t1378,t1379,t1381,t1384,t1385,t1386,t1387,t1390,t1391,t1392,t1393,t1394,t1395,t1397,t1398,t1399,t1400,t1403,t1404,t1406,t1407,t1408,t1411,t1412,t1413,t1414,t1417,t1418,t1419,t1420,t1421,t1426,t1427,t1431,t1434,t1435,t1438,t1439,t144,t1440,t1452,t1454,t1455,t1457,t1460,t1461,t1462,t1463,t1464,t1465,t1466,t1468,t1469,t1470,t1473,t1474,t1476,t1477,t1479,t1481,t1483,t1484,t1485,t1486,t1487,t1488,t1489,t1491,t1492,t1494,t1497,t1498,t1499,t15,t1500,t1501,t1502,t1504,t1506,t1510,t1511,t1512,t1513,t1514,t1515,t1516,t1518,t1520,t1522,t1523,t1524,t1525,t1528,t1529,t1531,t1537,t1538,t1539,t1542,t1543,t1544,t1545,t1558,t1561,t1564,t1567,t1568,t1569,t1571,t1576,t1577,t1579,t1580,t1582,t1597,t1600,t1608,t1612,t1614,t1615,t1634,t1635,t1645,t1650,t1654,t1656,t1657,t1658,t1671,t1675,t1677,t1685,t1687,t1691,t1693,t1695,t1698,t17,t170,t1705,t171,t1711,t1712,t1716,t172,t1733,t1735,t1740,t1777,t179,t18,t180,t1811,t183,t1831,t1836,t1867,t192,t1921,t1922,t1930,t194,t195,t1956,t1957,t1960,t1961,t1966,t1967,t2,t20,t200,t213,t214,t215,t216,t222,t230,t231,t237,t238,t241,t243,t245,t25,t253,t254,t257,t258,t26,t261,t263,t266,t267,t269,t270,t271,t272,t276,t277,t279,t29,t291,t294,t295,t298,t3,t30,t301,t302,t31,t325,t326,t327,t331,t332,t334,t337,t338,t339,t345,t346,t347,t348,t35,t350,t352,t353,t356,t357,t358,t36,t363,t372,t373,t377,t379,t380,t382,t385,t387,t39,t390,t393,t396,t40,t403,t408,t409,t417,t422,t423,t424,t426,t429,t432,t435,t444,t445,t446,t447,t452,t453,t454,t456,t459,t460,t473,t477,t478,t480,t491,t493,t494,t495,t496,t497,t500,t503,t504,t507,t513,t514,t517,t518,t520,t521,t523,t529,t533,t534,t535,t536,t542,t544,t545,t546,t547,t551,t552,t553,t554,t561,t567,t568,t569,t570,t574,t575,t577,t578,t579,t580,t581,t586,t587,t588,t589,t590,t592,t593,t594,t595,t596,t597,t598,t599,t6,t60,t600,t601,t602,t604,t609,t61,t612,t613,t614,t615,t617,t618,t622,t624,t63,t630,t631,t637,t639,t643,t646,t647,t657,t660,t661,t663,t664,t666,t667,t668,t675,t676,t679,t68,t682,t683,t684,t687,t688,t689,t690,t691,t692,t693,t694,t695,t696,t697,t698,t699,t7,t700,t702,t703,t704,t706,t708,t709,t71,t712,t714,t716,t717,t718,t719,t720,t721,t722,t723,t724,t725,t726,t727,t731,t734,t735,t736,t740,t746,t748,t75,t752,t755,t761,t763,t765,t766,t767,t769,t771,t772,t773,t774,t775,t776,t777,t778,t779,t780,t781,t782,t783,t784,t785,t787,t789,t790,t791,t794,t795,t797,t799,t8,t800,t801,t802,t803,t804,t810,t811,t812,t813,t817,t818,t819,t825,t827,t828,t831,t833,t842,t845,t848,t849,t850,t853,t854,t859,t860,t863,t864,t868,t869,t871,t872,t874,t877,t879,t880,t881,t886,t887,t888,t889,t890,t891,t892,t896,t897,t898,t9,t904,t905,t906,t907,t908,t909,t910,t913,t914,t915,t918,t920,t921,t922,t923,t929,t932,t933,t934,t935,t936,t937,t940,t941,t943,t944,t945,t946,t947,t948,t949,t950,t951,t952,t953,t954,t955,t956,t957,t958,t959,t960,t963,t964,t965,t966,t969,t970,t972,t973,t974,t975,t978,t979,t981,t985,t986,t987,t988,t990,t992,t993,t994,t995,t996});
end
function Yr = ft_3(ct)
qd1 = ct{1};
qd2 = ct{2};
qd3 = ct{3};
qd4 = ct{4};
qd5 = ct{5};
qd6 = ct{6};
qrd1 = ct{7};
qrd2 = ct{8};
qrd3 = ct{9};
qrd4 = ct{10};
qrd5 = ct{11};
qrd6 = ct{12};
qrdd1 = ct{13};
qrdd2 = ct{14};
qrdd3 = ct{15};
qrdd4 = ct{16};
qrdd5 = ct{17};
qrdd6 = ct{18};
t1001 = ct{19};
t1002 = ct{20};
t1003 = ct{21};
t1004 = ct{22};
t1005 = ct{23};
t1007 = ct{24};
t1009 = ct{25};
t1011 = ct{26};
t1012 = ct{27};
t1013 = ct{28};
t1014 = ct{29};
t1015 = ct{30};
t1016 = ct{31};
t1017 = ct{32};
t1018 = ct{33};
t1019 = ct{34};
t1020 = ct{35};
t1022 = ct{36};
t1025 = ct{37};
t1030 = ct{38};
t1032 = ct{39};
t1034 = ct{40};
t1035 = ct{41};
t1040 = ct{42};
t1041 = ct{43};
t1042 = ct{44};
t1043 = ct{45};
t1044 = ct{46};
t1046 = ct{47};
t1048 = ct{48};
t1049 = ct{49};
t1050 = ct{50};
t1051 = ct{51};
t1052 = ct{52};
t1053 = ct{53};
t1056 = ct{54};
t1059 = ct{55};
t1060 = ct{56};
t1063 = ct{57};
t1064 = ct{58};
t1067 = ct{59};
t1068 = ct{60};
t1069 = ct{61};
t1070 = ct{62};
t1071 = ct{63};
t1074 = ct{64};
t1075 = ct{65};
t1076 = ct{66};
t1077 = ct{67};
t1078 = ct{68};
t1079 = ct{69};
t1082 = ct{70};
t1083 = ct{71};
t1084 = ct{72};
t1085 = ct{73};
t1086 = ct{74};
t1087 = ct{75};
t1088 = ct{76};
t1089 = ct{77};
t1090 = ct{78};
t1091 = ct{79};
t1093 = ct{80};
t1094 = ct{81};
t1096 = ct{82};
t1097 = ct{83};
t1098 = ct{84};
t1099 = ct{85};
t1101 = ct{86};
t1102 = ct{87};
t1103 = ct{88};
t1104 = ct{89};
t1106 = ct{90};
t1107 = ct{91};
t1109 = ct{92};
t1111 = ct{93};
t1112 = ct{94};
t1113 = ct{95};
t1116 = ct{96};
t1118 = ct{97};
t1119 = ct{98};
t1120 = ct{99};
t1121 = ct{100};
t1122 = ct{101};
t1123 = ct{102};
t1124 = ct{103};
t1125 = ct{104};
t1126 = ct{105};
t1129 = ct{106};
t1130 = ct{107};
t1131 = ct{108};
t1132 = ct{109};
t1133 = ct{110};
t1134 = ct{111};
t1135 = ct{112};
t1137 = ct{113};
t1138 = ct{114};
t1139 = ct{115};
t1140 = ct{116};
t1141 = ct{117};
t1143 = ct{118};
t1144 = ct{119};
t1146 = ct{120};
t1147 = ct{121};
t1148 = ct{122};
t1152 = ct{123};
t1153 = ct{124};
t1154 = ct{125};
t1155 = ct{126};
t1156 = ct{127};
t1158 = ct{128};
t1161 = ct{129};
t1163 = ct{130};
t1164 = ct{131};
t1167 = ct{132};
t1168 = ct{133};
t1169 = ct{134};
t1170 = ct{135};
t1171 = ct{136};
t1175 = ct{137};
t1176 = ct{138};
t1177 = ct{139};
t1180 = ct{140};
t1181 = ct{141};
t1183 = ct{142};
t1184 = ct{143};
t1185 = ct{144};
t1186 = ct{145};
t1187 = ct{146};
t1190 = ct{147};
t1191 = ct{148};
t1192 = ct{149};
t1194 = ct{150};
t1196 = ct{151};
t1197 = ct{152};
t1199 = ct{153};
t12 = ct{154};
t1200 = ct{155};
t1201 = ct{156};
t1202 = ct{157};
t1203 = ct{158};
t1204 = ct{159};
t1207 = ct{160};
t1209 = ct{161};
t1210 = ct{162};
t1211 = ct{163};
t1212 = ct{164};
t1213 = ct{165};
t1214 = ct{166};
t1215 = ct{167};
t1216 = ct{168};
t1217 = ct{169};
t1218 = ct{170};
t1219 = ct{171};
t1220 = ct{172};
t1221 = ct{173};
t1222 = ct{174};
t1223 = ct{175};
t1224 = ct{176};
t1225 = ct{177};
t1226 = ct{178};
t1227 = ct{179};
t1228 = ct{180};
t1230 = ct{181};
t1231 = ct{182};
t1232 = ct{183};
t1233 = ct{184};
t1234 = ct{185};
t1235 = ct{186};
t1237 = ct{187};
t1238 = ct{188};
t1241 = ct{189};
t1242 = ct{190};
t1243 = ct{191};
t1244 = ct{192};
t1245 = ct{193};
t1246 = ct{194};
t1247 = ct{195};
t1248 = ct{196};
t1249 = ct{197};
t1250 = ct{198};
t1251 = ct{199};
t1253 = ct{200};
t1254 = ct{201};
t1255 = ct{202};
t1257 = ct{203};
t1258 = ct{204};
t1259 = ct{205};
t1260 = ct{206};
t1261 = ct{207};
t1262 = ct{208};
t1263 = ct{209};
t1265 = ct{210};
t1266 = ct{211};
t1267 = ct{212};
t1268 = ct{213};
t1269 = ct{214};
t127 = ct{215};
t1271 = ct{216};
t1272 = ct{217};
t1273 = ct{218};
t1274 = ct{219};
t1275 = ct{220};
t1276 = ct{221};
t1277 = ct{222};
t1278 = ct{223};
t1279 = ct{224};
t1281 = ct{225};
t1283 = ct{226};
t1284 = ct{227};
t1287 = ct{228};
t1292 = ct{229};
t1293 = ct{230};
t1294 = ct{231};
t1295 = ct{232};
t1296 = ct{233};
t1297 = ct{234};
t1298 = ct{235};
t13 = ct{236};
t1302 = ct{237};
t1303 = ct{238};
t1304 = ct{239};
t1305 = ct{240};
t1306 = ct{241};
t1307 = ct{242};
t1309 = ct{243};
t1311 = ct{244};
t1312 = ct{245};
t1316 = ct{246};
t1317 = ct{247};
t1318 = ct{248};
t132 = ct{249};
t1320 = ct{250};
t1321 = ct{251};
t1323 = ct{252};
t1325 = ct{253};
t1326 = ct{254};
t1329 = ct{255};
t133 = ct{256};
t1330 = ct{257};
t1331 = ct{258};
t1332 = ct{259};
t1333 = ct{260};
t1334 = ct{261};
t1336 = ct{262};
t1337 = ct{263};
t1342 = ct{264};
t1344 = ct{265};
t1346 = ct{266};
t1348 = ct{267};
t1349 = ct{268};
t1350 = ct{269};
t1354 = ct{270};
t1356 = ct{271};
t1358 = ct{272};
t1362 = ct{273};
t1364 = ct{274};
t1365 = ct{275};
t1366 = ct{276};
t1367 = ct{277};
t1368 = ct{278};
t1369 = ct{279};
t1370 = ct{280};
t1371 = ct{281};
t1372 = ct{282};
t1375 = ct{283};
t1377 = ct{284};
t1378 = ct{285};
t1379 = ct{286};
t1381 = ct{287};
t1384 = ct{288};
t1385 = ct{289};
t1386 = ct{290};
t1387 = ct{291};
t1390 = ct{292};
t1391 = ct{293};
t1392 = ct{294};
t1393 = ct{295};
t1394 = ct{296};
t1395 = ct{297};
t1397 = ct{298};
t1398 = ct{299};
t1399 = ct{300};
t1400 = ct{301};
t1403 = ct{302};
t1404 = ct{303};
t1406 = ct{304};
t1407 = ct{305};
t1408 = ct{306};
t1411 = ct{307};
t1412 = ct{308};
t1413 = ct{309};
t1414 = ct{310};
t1417 = ct{311};
t1418 = ct{312};
t1419 = ct{313};
t1420 = ct{314};
t1421 = ct{315};
t1426 = ct{316};
t1427 = ct{317};
t1431 = ct{318};
t1434 = ct{319};
t1435 = ct{320};
t1438 = ct{321};
t1439 = ct{322};
t144 = ct{323};
t1440 = ct{324};
t1452 = ct{325};
t1454 = ct{326};
t1455 = ct{327};
t1457 = ct{328};
t1460 = ct{329};
t1461 = ct{330};
t1462 = ct{331};
t1463 = ct{332};
t1464 = ct{333};
t1465 = ct{334};
t1466 = ct{335};
t1468 = ct{336};
t1469 = ct{337};
t1470 = ct{338};
t1473 = ct{339};
t1474 = ct{340};
t1476 = ct{341};
t1477 = ct{342};
t1479 = ct{343};
t1481 = ct{344};
t1483 = ct{345};
t1484 = ct{346};
t1485 = ct{347};
t1486 = ct{348};
t1487 = ct{349};
t1488 = ct{350};
t1489 = ct{351};
t1491 = ct{352};
t1492 = ct{353};
t1494 = ct{354};
t1497 = ct{355};
t1498 = ct{356};
t1499 = ct{357};
t15 = ct{358};
t1500 = ct{359};
t1501 = ct{360};
t1502 = ct{361};
t1504 = ct{362};
t1506 = ct{363};
t1510 = ct{364};
t1511 = ct{365};
t1512 = ct{366};
t1513 = ct{367};
t1514 = ct{368};
t1515 = ct{369};
t1516 = ct{370};
t1518 = ct{371};
t1520 = ct{372};
t1522 = ct{373};
t1523 = ct{374};
t1524 = ct{375};
t1525 = ct{376};
t1528 = ct{377};
t1529 = ct{378};
t1531 = ct{379};
t1537 = ct{380};
t1538 = ct{381};
t1539 = ct{382};
t1542 = ct{383};
t1543 = ct{384};
t1544 = ct{385};
t1545 = ct{386};
t1558 = ct{387};
t1561 = ct{388};
t1564 = ct{389};
t1567 = ct{390};
t1568 = ct{391};
t1569 = ct{392};
t1571 = ct{393};
t1576 = ct{394};
t1577 = ct{395};
t1579 = ct{396};
t1580 = ct{397};
t1582 = ct{398};
t1597 = ct{399};
t1600 = ct{400};
t1608 = ct{401};
t1612 = ct{402};
t1614 = ct{403};
t1615 = ct{404};
t1634 = ct{405};
t1635 = ct{406};
t1645 = ct{407};
t1650 = ct{408};
t1654 = ct{409};
t1656 = ct{410};
t1657 = ct{411};
t1658 = ct{412};
t1671 = ct{413};
t1675 = ct{414};
t1677 = ct{415};
t1685 = ct{416};
t1687 = ct{417};
t1691 = ct{418};
t1693 = ct{419};
t1695 = ct{420};
t1698 = ct{421};
t17 = ct{422};
t170 = ct{423};
t1705 = ct{424};
t171 = ct{425};
t1711 = ct{426};
t1712 = ct{427};
t1716 = ct{428};
t172 = ct{429};
t1733 = ct{430};
t1735 = ct{431};
t1740 = ct{432};
t1777 = ct{433};
t179 = ct{434};
t18 = ct{435};
t180 = ct{436};
t1811 = ct{437};
t183 = ct{438};
t1831 = ct{439};
t1836 = ct{440};
t1867 = ct{441};
t192 = ct{442};
t1921 = ct{443};
t1922 = ct{444};
t1930 = ct{445};
t194 = ct{446};
t195 = ct{447};
t1956 = ct{448};
t1957 = ct{449};
t1960 = ct{450};
t1961 = ct{451};
t1966 = ct{452};
t1967 = ct{453};
t2 = ct{454};
t20 = ct{455};
t200 = ct{456};
t213 = ct{457};
t214 = ct{458};
t215 = ct{459};
t216 = ct{460};
t222 = ct{461};
t230 = ct{462};
t231 = ct{463};
t237 = ct{464};
t238 = ct{465};
t241 = ct{466};
t243 = ct{467};
t245 = ct{468};
t25 = ct{469};
t253 = ct{470};
t254 = ct{471};
t257 = ct{472};
t258 = ct{473};
t26 = ct{474};
t261 = ct{475};
t263 = ct{476};
t266 = ct{477};
t267 = ct{478};
t269 = ct{479};
t270 = ct{480};
t271 = ct{481};
t272 = ct{482};
t276 = ct{483};
t277 = ct{484};
t279 = ct{485};
t29 = ct{486};
t291 = ct{487};
t294 = ct{488};
t295 = ct{489};
t298 = ct{490};
t3 = ct{491};
t30 = ct{492};
t301 = ct{493};
t302 = ct{494};
t31 = ct{495};
t325 = ct{496};
t326 = ct{497};
t327 = ct{498};
t331 = ct{499};
t332 = ct{500};
t334 = ct{501};
t337 = ct{502};
t338 = ct{503};
t339 = ct{504};
t345 = ct{505};
t346 = ct{506};
t347 = ct{507};
t348 = ct{508};
t35 = ct{509};
t350 = ct{510};
t352 = ct{511};
t353 = ct{512};
t356 = ct{513};
t357 = ct{514};
t358 = ct{515};
t36 = ct{516};
t363 = ct{517};
t372 = ct{518};
t373 = ct{519};
t377 = ct{520};
t379 = ct{521};
t380 = ct{522};
t382 = ct{523};
t385 = ct{524};
t387 = ct{525};
t39 = ct{526};
t390 = ct{527};
t393 = ct{528};
t396 = ct{529};
t40 = ct{530};
t403 = ct{531};
t408 = ct{532};
t409 = ct{533};
t417 = ct{534};
t422 = ct{535};
t423 = ct{536};
t424 = ct{537};
t426 = ct{538};
t429 = ct{539};
t432 = ct{540};
t435 = ct{541};
t444 = ct{542};
t445 = ct{543};
t446 = ct{544};
t447 = ct{545};
t452 = ct{546};
t453 = ct{547};
t454 = ct{548};
t456 = ct{549};
t459 = ct{550};
t460 = ct{551};
t473 = ct{552};
t477 = ct{553};
t478 = ct{554};
t480 = ct{555};
t491 = ct{556};
t493 = ct{557};
t494 = ct{558};
t495 = ct{559};
t496 = ct{560};
t497 = ct{561};
t500 = ct{562};
t503 = ct{563};
t504 = ct{564};
t507 = ct{565};
t513 = ct{566};
t514 = ct{567};
t517 = ct{568};
t518 = ct{569};
t520 = ct{570};
t521 = ct{571};
t523 = ct{572};
t529 = ct{573};
t533 = ct{574};
t534 = ct{575};
t535 = ct{576};
t536 = ct{577};
t542 = ct{578};
t544 = ct{579};
t545 = ct{580};
t546 = ct{581};
t547 = ct{582};
t551 = ct{583};
t552 = ct{584};
t553 = ct{585};
t554 = ct{586};
t561 = ct{587};
t567 = ct{588};
t568 = ct{589};
t569 = ct{590};
t570 = ct{591};
t574 = ct{592};
t575 = ct{593};
t577 = ct{594};
t578 = ct{595};
t579 = ct{596};
t580 = ct{597};
t581 = ct{598};
t586 = ct{599};
t587 = ct{600};
t588 = ct{601};
t589 = ct{602};
t590 = ct{603};
t592 = ct{604};
t593 = ct{605};
t594 = ct{606};
t595 = ct{607};
t596 = ct{608};
t597 = ct{609};
t598 = ct{610};
t599 = ct{611};
t6 = ct{612};
t60 = ct{613};
t600 = ct{614};
t601 = ct{615};
t602 = ct{616};
t604 = ct{617};
t609 = ct{618};
t61 = ct{619};
t612 = ct{620};
t613 = ct{621};
t614 = ct{622};
t615 = ct{623};
t617 = ct{624};
t618 = ct{625};
t622 = ct{626};
t624 = ct{627};
t63 = ct{628};
t630 = ct{629};
t631 = ct{630};
t637 = ct{631};
t639 = ct{632};
t643 = ct{633};
t646 = ct{634};
t647 = ct{635};
t657 = ct{636};
t660 = ct{637};
t661 = ct{638};
t663 = ct{639};
t664 = ct{640};
t666 = ct{641};
t667 = ct{642};
t668 = ct{643};
t675 = ct{644};
t676 = ct{645};
t679 = ct{646};
t68 = ct{647};
t682 = ct{648};
t683 = ct{649};
t684 = ct{650};
t687 = ct{651};
t688 = ct{652};
t689 = ct{653};
t690 = ct{654};
t691 = ct{655};
t692 = ct{656};
t693 = ct{657};
t694 = ct{658};
t695 = ct{659};
t696 = ct{660};
t697 = ct{661};
t698 = ct{662};
t699 = ct{663};
t7 = ct{664};
t700 = ct{665};
t702 = ct{666};
t703 = ct{667};
t704 = ct{668};
t706 = ct{669};
t708 = ct{670};
t709 = ct{671};
t71 = ct{672};
t712 = ct{673};
t714 = ct{674};
t716 = ct{675};
t717 = ct{676};
t718 = ct{677};
t719 = ct{678};
t720 = ct{679};
t721 = ct{680};
t722 = ct{681};
t723 = ct{682};
t724 = ct{683};
t725 = ct{684};
t726 = ct{685};
t727 = ct{686};
t731 = ct{687};
t734 = ct{688};
t735 = ct{689};
t736 = ct{690};
t740 = ct{691};
t746 = ct{692};
t748 = ct{693};
t75 = ct{694};
t752 = ct{695};
t755 = ct{696};
t761 = ct{697};
t763 = ct{698};
t765 = ct{699};
t766 = ct{700};
t767 = ct{701};
t769 = ct{702};
t771 = ct{703};
t772 = ct{704};
t773 = ct{705};
t774 = ct{706};
t775 = ct{707};
t776 = ct{708};
t777 = ct{709};
t778 = ct{710};
t779 = ct{711};
t780 = ct{712};
t781 = ct{713};
t782 = ct{714};
t783 = ct{715};
t784 = ct{716};
t785 = ct{717};
t787 = ct{718};
t789 = ct{719};
t790 = ct{720};
t791 = ct{721};
t794 = ct{722};
t795 = ct{723};
t797 = ct{724};
t799 = ct{725};
t8 = ct{726};
t800 = ct{727};
t801 = ct{728};
t802 = ct{729};
t803 = ct{730};
t804 = ct{731};
t810 = ct{732};
t811 = ct{733};
t812 = ct{734};
t813 = ct{735};
t817 = ct{736};
t818 = ct{737};
t819 = ct{738};
t825 = ct{739};
t827 = ct{740};
t828 = ct{741};
t831 = ct{742};
t833 = ct{743};
t842 = ct{744};
t845 = ct{745};
t848 = ct{746};
t849 = ct{747};
t850 = ct{748};
t853 = ct{749};
t854 = ct{750};
t859 = ct{751};
t860 = ct{752};
t863 = ct{753};
t864 = ct{754};
t868 = ct{755};
t869 = ct{756};
t871 = ct{757};
t872 = ct{758};
t874 = ct{759};
t877 = ct{760};
t879 = ct{761};
t880 = ct{762};
t881 = ct{763};
t886 = ct{764};
t887 = ct{765};
t888 = ct{766};
t889 = ct{767};
t890 = ct{768};
t891 = ct{769};
t892 = ct{770};
t896 = ct{771};
t897 = ct{772};
t898 = ct{773};
t9 = ct{774};
t904 = ct{775};
t905 = ct{776};
t906 = ct{777};
t907 = ct{778};
t908 = ct{779};
t909 = ct{780};
t910 = ct{781};
t913 = ct{782};
t914 = ct{783};
t915 = ct{784};
t918 = ct{785};
t920 = ct{786};
t921 = ct{787};
t922 = ct{788};
t923 = ct{789};
t929 = ct{790};
t932 = ct{791};
t933 = ct{792};
t934 = ct{793};
t935 = ct{794};
t936 = ct{795};
t937 = ct{796};
t940 = ct{797};
t941 = ct{798};
t943 = ct{799};
t944 = ct{800};
t945 = ct{801};
t946 = ct{802};
t947 = ct{803};
t948 = ct{804};
t949 = ct{805};
t950 = ct{806};
t951 = ct{807};
t952 = ct{808};
t953 = ct{809};
t954 = ct{810};
t955 = ct{811};
t956 = ct{812};
t957 = ct{813};
t958 = ct{814};
t959 = ct{815};
t960 = ct{816};
t963 = ct{817};
t964 = ct{818};
t965 = ct{819};
t966 = ct{820};
t969 = ct{821};
t970 = ct{822};
t972 = ct{823};
t973 = ct{824};
t974 = ct{825};
t975 = ct{826};
t978 = ct{827};
t979 = ct{828};
t981 = ct{829};
t985 = ct{830};
t986 = ct{831};
t987 = ct{832};
t988 = ct{833};
t990 = ct{834};
t992 = ct{835};
t993 = ct{836};
t994 = ct{837};
t995 = ct{838};
t996 = ct{839};
t1282 = t195.*t1009.*8.084033333333334e-4;
t1285 = t13.*t172.*t1009.*8.084033333333334e-4;
t1290 = (t8.*t491.*t1048)./2.0;
t1291 = t238.*t1009.*8.084033333333334e-4;
t1300 = -t1296;
t1310 = t567.*t1048;
t1313 = (t717.*t915)./2.0;
t1314 = t271.*t1009.*8.084033333333334e-4;
t1315 = t272.*t1009.*8.084033333333334e-4;
t1327 = t270+t294+t353+t357+t393+t417;
t1328 = t327.*t1009.*8.084033333333334e-4;
t1338 = t1009.*(t61-t241).*(-8.084033333333334e-4);
t1340 = (t2.*t1330)./2.0;
t1341 = (t8.*t1329)./2.0;
t1345 = t2.*t29.*t1329;
t1347 = t8.*t29.*t1330;
t1355 = -t1348;
t1360 = t1348./2.0;
t1373 = t909+t918;
t1374 = t325+t825+t849;
t1380 = t8.*t763.*t1048;
t1383 = t8.*t774.*t1048;
t1389 = t818.*t1048;
t1401 = -t1398;
t1402 = t8.*t491.*t1238;
t1405 = -t1400;
t1409 = -t1404;
t1416 = t8.*t863.*t1048;
t1423 = -t1419;
t1424 = t8.*t879.*t1048;
t1425 = t887.*t1048;
t1428 = (t567.*t1238)./2.0;
t1429 = -t1420;
t1437 = t718.*t1187;
t1441 = t8.*t914.*t1048;
t1445 = t979+t1003;
t1446 = t987+t996;
t1449 = t238.*t1279.*4.042016666666667e-4;
t1450 = t238.*t1279.*8.084033333333334e-4;
t1451 = t988+t1005;
t1467 = t327.*t1279.*8.084033333333334e-4;
t1475 = t8.*t763.*t1238;
t1478 = t1279.*(t61-t241).*(-8.084033333333334e-4);
t1482 = t8.*t774.*t1238;
t1493 = (t818.*t1238)./2.0;
t1509 = t1069+t1075;
t1517 = t8.*t863.*t1238;
t1519 = -t1512;
t1526 = t8.*t879.*t1238;
t1527 = (t29.*t1491)./2.0;
t1532 = -t1529;
t1533 = (t887.*t1238)./2.0;
t1535 = t194.*t1386.*4.042016666666667e-4;
t1536 = t194.*t1386.*8.084033333333334e-4;
t1540 = t495+t497+t1262;
t1541 = t8.*t914.*t1238;
t1546 = t238.*t1399.*4.042016666666667e-4;
t1547 = t238.*t1399.*8.084033333333334e-4;
t1549 = (t994.*t1187)./2.0;
t1552 = t735+t794+t986;
t1553 = t736+t779+t995;
t1556 = t1386.*(t60-t192).*(-8.084033333333334e-4);
t1557 = t345.*t1386.*8.084033333333334e-4;
t1559 = t1386.*(t60-t192).*8.084033333333334e-4;
t1565 = t327.*t1399.*8.084033333333334e-4;
t1566 = t631+t647+t740+t752;
t1570 = -t1048.*(t446-t970);
t1572 = t1399.*(t61-t241).*(-8.084033333333334e-4);
t1578 = t1048.*t1238;
t1581 = -t1580;
t1591 = t915.*t1371;
t1599 = t718.*t1452;
t1603 = (t1085.*t1283)./2.0;
t1617 = qd1.*t1614;
t1618 = -t1238.*(t446-t970);
t1625 = t845+t848+t1184;
t1627 = t1187.*t1298;
t1659 = (t8.*t763.*t1522)./2.0;
t1663 = t994.*t1452;
t1669 = (t915.*t1485)./2.0;
t1672 = (t8.*t863.*t1522)./2.0;
t1678 = t643+t646+t1455;
t1679 = (t2.*t763.*t1571)./2.0;
t1680 = t518+t1216+t1221;
t1684 = (t1187.*t1393)./2.0;
t1686 = (t2.*t1677)./2.0;
t1688 = (t8.*t914.*t1522)./2.0;
t1704 = qd1.*t1698;
t1706 = (t2.*t863.*t1571)./2.0;
t1707 = (t132.*t1677)./2.0;
t1709 = -t1283.*(t908-t909);
t1710 = t200+t339+t761+t769+t831+t842;
t1715 = t8.*t1705;
t1731 = t1187.*t1452;
t1734 = (t1048.*t1522)./2.0;
t1736 = (t2.*t914.*t1571)./2.0;
t1738 = (t2.*t29.*t1705)./2.0;
t1747 = (t8.*t763.*t1608)./2.0;
t1751 = (t172.*t1705)./2.0;
t1752 = (t2.*t763.*t1612)./2.0;
t1755 = t346+t348+t1650;
t1759 = (t1187.*t1486)./2.0;
t1764 = (t1051.*t1571)./2.0;
t1767 = (t8.*t863.*t1608)./2.0;
t1769 = t1048.*(t263+t456-t922-t978).*(-1.0./2.0);
t1771 = (t1048.*(t263+t456-t922-t978))./2.0;
t1773 = t1298.*t1452;
t1774 = (t2.*t863.*t1612)./2.0;
t1779 = -t1522.*(t446-t970);
t1781 = (t8.*t914.*t1608)./2.0;
t1786 = (t2.*t914.*t1612)./2.0;
t1805 = t1187.*t1567;
t1809 = -t1571.*(t429-t960);
t1810 = (t1048.*t1608)./2.0;
t1815 = (t1051.*t1612)./2.0;
t1819 = -t2.*(-t675+t1009.*(t61-t241).*8.084033333333334e-4+t345.*(t291-t477+t172.*(t60-t192)).*8.084033333333334e-4);
t1820 = (t1234.*t1571)./2.0;
t1822 = t1238.*(t263+t456-t922-t978).*(-1.0./2.0);
t1823 = (t1238.*(t263+t456-t922-t978))./2.0;
t1826 = t8.*t25.*(-t675+t1009.*(t61-t241).*8.084033333333334e-4+t345.*(t291-t477+t172.*(t60-t192)).*8.084033333333334e-4).*(-1.0./2.0);
t1828 = (t8.*t25.*(-t675+t1009.*(t61-t241).*8.084033333333334e-4+t345.*(t291-t477+t172.*(t60-t192)).*8.084033333333334e-4))./2.0;
t1829 = t29.*t30.*(-t675+t1009.*(t61-t241).*8.084033333333334e-4+t345.*(t291-t477+t172.*(t60-t192)).*8.084033333333334e-4).*(-1.0./2.0);
t1830 = (t29.*t30.*(-t675+t1009.*(t61-t241).*8.084033333333334e-4+t345.*(t291-t477+t172.*(t60-t192)).*8.084033333333334e-4))./2.0;
t1839 = t171.*(-t675+t1009.*(t61-t241).*8.084033333333334e-4+t345.*(t291-t477+t172.*(t60-t192)).*8.084033333333334e-4).*(-1.0./2.0);
t1840 = (t171.*(-t675+t1009.*(t61-t241).*8.084033333333334e-4+t345.*(t291-t477+t172.*(t60-t192)).*8.084033333333334e-4))./2.0;
t1847 = t1612.*(t429-t960).*(-1.0./2.0);
t1848 = t1608.*(t446-t970).*(-1.0./2.0);
t1851 = (t1612.*(t429-t960))./2.0;
t1852 = (t1608.*(t446-t970))./2.0;
t1853 = t1238.*t1608;
t1855 = t1234.*t1612;
t1857 = t237+t517+t542+t1311+t1318;
t1863 = (t1452.*t1486)./2.0;
t1868 = qd1.*t1867;
t1873 = (t1452.*t1567)./2.0;
t1884 = t513+t514+t694+t695+t1576;
t1885 = t493+t494+t513+t514+t1645;
t1898 = t237+t517+t542+t1390+t1395;
t1914 = t237+t517+t542+t1426+t1431;
t1918 = t513+t514+t577+t578+t1675;
t1933 = qd1.*t1930;
t1936 = (t25.*t1921)./2.0;
t1943 = t724+t734+t828+t952+t1001+t1170;
t1944 = t721+t731+t827+t951+t1004+t1163;
t2027 = t941+t946+t1041+t1050+t1227+t1228+t1515+t1524;
t2028 = t985+t1002+t1104+t1107+t1227+t1228+t1515+t1524;
t2030 = t1146+t1148+t1153+t1161+t1272+t1273+t1516+t1523;
t2050 = t692+t693+t709+t716+t787+t799+t813+t937+t950+t1116+t1125+t1126+t1274+t1276+t1656+t1657;
t2055 = t709+t716+t787+t799+t804+t810+t813+t937+t950+t1116+t1125+t1126+t1375+t1378+t1656+t1657;
t2060 = t709+t716+t787+t799+t813+t872+t880+t937+t950+t1116+t1125+t1126+t1411+t1413+t1656+t1657;
t1026 = -t1016;
t1036 = -t1025;
t1065 = -t1060;
t1066 = -t1063;
t1128 = t390.*t947;
t1145 = t6.*t1137;
t1149 = -t1143;
t1150 = -t1144;
t1174 = t2.*t1158;
t1195 = -t1181;
t1198 = -t1191;
t1208 = -t1203;
t1229 = -t1225;
t1239 = -t1233;
t1256 = -t1253;
t1270 = t25.*t1255;
t1288 = -t1282;
t1289 = -t1281;
t1299 = -t1290;
t1319 = -t1313;
t1322 = -t1315;
t1324 = -t1310;
t1339 = -t947.*(t2.*(t298-t2.*t9.*(1.53e+2./2.5e+2))+t8.*(t301-t8.*t9.*(1.53e+2./2.5e+2)));
t1343 = t797.*t947;
t1353 = -t1345;
t1357 = t1345./2.0;
t1359 = t1347./2.0;
t1363 = -t1360;
t1396 = -t1389;
t1410 = -t1402;
t1430 = -t1428;
t1432 = -t1425;
t1436 = t717.*t1186;
t1442 = -t1437;
t1443 = t194.*t1278.*4.042016666666667e-4;
t1444 = t194.*t1278.*8.084033333333334e-4;
t1456 = (t2.*t1445)./2.0;
t1471 = t1278.*(t60-t192).*(-8.084033333333334e-4);
t1472 = t345.*t1278.*8.084033333333334e-4;
t1496 = -t1493;
t1507 = t915.*t1186;
t1508 = t1068+t1074;
t1530 = -t1527;
t1534 = -t1533;
t1548 = (t993.*t1186)./2.0;
t1551 = -t1549;
t1554 = t2.*t1553;
t1555 = t8.*t1552;
t1560 = -t1557;
t1573 = (t2.*t25.*t1552)./2.0;
t1575 = (t8.*t25.*t1553)./2.0;
t1593 = t1175+t1196;
t1595 = t579+t581+t1355;
t1596 = -t1591;
t1598 = t717.*t1451;
t1602 = -t1599;
t1606 = t1599./2.0;
t1607 = -t1603;
t1611 = (t1186.*(t387+t473+t478+t26.*t29.*t132.*1.383e-1))./2.0;
t1619 = t601+t1084+t1093;
t1620 = t588+t1094+t1106;
t1624 = t718.*t1509;
t1626 = t1186.*t1297;
t1642 = t915.*t1451;
t1662 = t993.*t1451;
t1664 = -t1663;
t1666 = t1663./2.0;
t1670 = -t1669;
t1681 = -t1679;
t1682 = qd3.*t1678;
t1683 = (t1186.*t1392)./2.0;
t1690 = -t1684;
t1692 = -t1686;
t1694 = qd1.*t1680;
t1697 = t994.*t1509;
t1708 = -t1706;
t1719 = -t1715;
t1720 = t2.*t1710;
t1721 = (t915.*t1566)./2.0;
t1724 = t1715./2.0;
t1730 = t1186.*t1451;
t1732 = t700+t1202+t1219;
t1737 = -t1734;
t1739 = -t1738;
t1741 = (t8.*t29.*t1710)./2.0;
t1743 = (t1451.*(t387+t473+t478+t26.*t29.*t132.*1.383e-1))./2.0;
t1749 = -t1747;
t1753 = (t132.*t1710)./2.0;
t1754 = -t1751;
t1756 = -t1752;
t1757 = t702+t703+t1519;
t1758 = (t1186.*t1485)./2.0;
t1761 = -t1759;
t1766 = t1187.*t1509;
t1768 = -t1764;
t1770 = -t1767;
t1772 = t1297.*t1451;
t1775 = t599+t1287+t1291;
t1776 = -t1774;
t1780 = t794+t1251+t1254;
t1783 = -t1781;
t1790 = -t1786;
t1792 = -t2.*(t779+t1253+t907.*(t61-t241).*8.084033333333334e-4);
t1795 = t2.*(t779+t1253+t907.*(t61-t241).*8.084033333333334e-4);
t1800 = t8.*t25.*(t779+t1253+t907.*(t61-t241).*8.084033333333334e-4).*(-1.0./2.0);
t1802 = (t8.*t25.*(t779+t1253+t907.*(t61-t241).*8.084033333333334e-4))./2.0;
t1803 = t29.*t30.*(t779+t1253+t907.*(t61-t241).*8.084033333333334e-4).*(-1.0./2.0);
t1804 = t1186.*t1566;
t1807 = t1298.*t1509;
t1812 = t346+t348+t1709;
t1813 = (t1371.*t1451)./2.0;
t1816 = t688+t1328+t1333;
t1817 = t675+t1334+t1338;
t1821 = -t1820;
t1841 = t183+t657+t679+t1215+t1220;
t1844 = qd1.*(-t170+t657+t679+t1215+t1220);
t1846 = (t1393.*t1509)./2.0;
t1854 = -t1853;
t1856 = -t1855;
t1858 = qd1.*t1857;
t1862 = (t1451.*t1485)./2.0;
t1866 = t1452.*t1509;
t1871 = t520+t944+t965+t1034+t1044;
t1872 = (t1451.*t1566)./2.0;
t1875 = -t1873;
t1880 = t521+t536+t897+t905+t973+t975;
t1893 = (t1509.*t1567)./2.0;
t1900 = qd1.*t1898;
t1916 = qd1.*t1914;
t1919 = t593+t618+t953+t957+t1030+t1032;
t1920 = t594+t617+t958+t963+t1017+t1018;
t1923 = t8.*(t589+t602-t953-t1030-t1032+t452.*(t60-t192).*8.084033333333334e-4).*(-1.0./2.0);
t1924 = t2.*(t590+t600-t958-t1017-t1018+t453.*(t61-t241).*8.084033333333334e-4).*(-1.0./2.0);
t1927 = -t8.*t29.*(t590+t600-t958-t1017-t1018+t453.*(t61-t241).*8.084033333333334e-4);
t1931 = -t2.*t29.*(t589+t602-t953-t1030-t1032+t452.*(t60-t192).*8.084033333333334e-4);
t1932 = t8.*t29.*(t590+t600-t958-t1017-t1018+t453.*(t61-t241).*8.084033333333334e-4);
t1935 = t2.*t29.*(t589+t602-t953-t1030-t1032+t452.*(t60-t192).*8.084033333333334e-4).*(-1.0./2.0);
t1937 = (t2.*t29.*(t589+t602-t953-t1030-t1032+t452.*(t60-t192).*8.084033333333334e-4))./2.0;
t1941 = t132.*(t590+t600-t958-t1017-t1018+t453.*(t61-t241).*8.084033333333334e-4).*(-1.0./2.0);
t1942 = t172.*(t589+t602-t953-t1030-t1032+t452.*(t60-t192).*8.084033333333334e-4).*(-1.0./2.0);
t1945 = t8.*t1944;
t1946 = t2.*t1943;
t1953 = (t2.*t29.*t1944)./2.0;
t1954 = (t8.*t29.*t1943)./2.0;
t1958 = t546+t785+t1528+t1532;
t1964 = t8.*(t773-t790-t1089+t1203-t1214+t660.*(t60-t192).*8.084033333333334e-4).*(-1.0./2.0);
t1970 = t889+t890+t1134+t1138+t1773;
t1977 = t708+t949+t1211+t1213+t1465+t1477;
t1979 = t25.*(t697+t945-t1211-t1213+t194.*(-t270-t294+t334+t337+t396+t2.*t25.*(t60-t192)).*8.084033333333334e-4+t238.*(-t269-t295+t352+t356+t385+t8.*t25.*(t61-t241)).*8.084033333333334e-4).*(-1.0./2.0);
t1980 = (t25.*(t697+t945-t1211-t1213+t194.*(-t270-t294+t334+t337+t396+t2.*t25.*(t60-t192)).*8.084033333333334e-4+t238.*(-t269-t295+t352+t356+t385+t8.*t25.*(t61-t241)).*8.084033333333334e-4))./2.0;
t1981 = t12.*t29.*(t697+t945-t1211-t1213+t194.*(-t270-t294+t334+t337+t396+t2.*t25.*(t60-t192)).*8.084033333333334e-4+t238.*(-t269-t295+t352+t356+t385+t8.*t25.*(t61-t241)).*8.084033333333334e-4).*(-1.0./2.0);
t1985 = t8.*(t676+t913-t1285-t1467+t1278.*(t60-t192).*8.084033333333334e-4+t7.*t172.*(t291-t477+t172.*(t60-t192)).*8.084033333333334e-4).*(-1.0./2.0);
t1988 = t721+t1004+t1217+t1230+t1489+t1498;
t1989 = t724+t1001+t1218+t1231+t1492+t1511;
t1997 = t172.*(t676+t913-t1285-t1467+t1278.*(t60-t192).*8.084033333333334e-4+t7.*t172.*(t291-t477+t172.*(t60-t192)).*8.084033333333334e-4).*(-1.0./2.0);
t2010 = t622+t850+t1309+t1314+t1559+t1565;
t2015 = -t2.*(t624-t833+t1315+t1557+t1399.*(t61-t241).*8.084033333333334e-4+t254.*(t291-t477+t172.*(t60-t192)).*8.084033333333334e-4);
t2017 = t2.*(t624-t833+t1315+t1557+t1399.*(t61-t241).*8.084033333333334e-4+t254.*(t291-t477+t172.*(t60-t192)).*8.084033333333334e-4).*(-1.0./2.0);
t2018 = (t2.*(t624-t833+t1315+t1557+t1399.*(t61-t241).*8.084033333333334e-4+t254.*(t291-t477+t172.*(t60-t192)).*8.084033333333334e-4))./2.0;
t2021 = t8.*t29.*(t624-t833+t1315+t1557+t1399.*(t61-t241).*8.084033333333334e-4+t254.*(t291-t477+t172.*(t60-t192)).*8.084033333333334e-4).*(-1.0./2.0);
t2022 = (t8.*t29.*(t624-t833+t1315+t1557+t1399.*(t61-t241).*8.084033333333334e-4+t254.*(t291-t477+t172.*(t60-t192)).*8.084033333333334e-4))./2.0;
t2025 = t132.*(t624-t833+t1315+t1557+t1399.*(t61-t241).*8.084033333333334e-4+t254.*(t291-t477+t172.*(t60-t192)).*8.084033333333334e-4).*(-1.0./2.0);
t2051 = -qd1.*(t689+t691+t706+t725-t787+t791-t813-t937+t956-t1116+t1130+t1131+t1268+t1654+(t568.*(t426-t712))./2.0+(t1049.*(t424-t435-t609+t714))./2.0);
t2056 = -qd1.*(t706+t725-t787+t791+t795+t802-t813-t937+t956-t1116+t1130+t1131+t1372+t1654+(t819.*(t426-t712))./2.0+(t1049.*(t424-t435-t609+t714))./2.0);
t2061 = -qd1.*(t706+t725-t787+t791-t813+t864+t871-t937+t956-t1116+t1130+t1131+t1408+t1654+(t888.*(t426-t712))./2.0+(t1049.*(t424-t435-t609+t714))./2.0);
t2071 = t689+t691+t1022+t1077+t1078+t1079+t1130+t1131+t1176+t1177+t1274+t1276+t1537+t1538+t1656+t1657;
t2078 = t795+t802+t1022+t1077+t1078+t1079+t1130+t1131+t1176+t1177+t1375+t1378+t1537+t1538+t1656+t1657;
t2079 = t864+t871+t1022+t1077+t1078+t1079+t1130+t1131+t1176+t1177+t1411+t1413+t1537+t1538+t1656+t1657;
t1286 = t1270./2.0;
t1361 = -t1357;
t1376 = t454+t459+t1026;
t1447 = -t1444;
t1448 = -t1443;
t1459 = -t1456;
t1480 = t331+t338+t1339;
t1550 = -t1548;
t1562 = -t1555;
t1583 = t523+t1036+t1042;
t1592 = t1174+t1195;
t1601 = -t1598;
t1604 = t213+t214+t447+t460+t1343;
t1605 = t1598./2.0;
t1610 = -t1606;
t1613 = -t1611;
t1621 = t8.*t1619;
t1622 = t2.*t1620;
t1623 = t717.*t1508;
t1629 = t2.*t29.*t1619;
t1631 = -t1624;
t1633 = t1624./2.0;
t1637 = t8.*t29.*t1620;
t1640 = (t2.*t25.*t1619)./2.0;
t1643 = (t26.*t29.*t1619)./2.0;
t1644 = (t8.*t25.*t1620)./2.0;
t1648 = (t29.*t30.*t1620)./2.0;
t1651 = t172.*t1619;
t1652 = t132.*t1620;
t1653 = (t133.*t1619)./2.0;
t1660 = (t171.*t1620)./2.0;
t1665 = t1662./2.0;
t1668 = -t1666;
t1674 = t915.*t1508;
t1689 = -t1683;
t1696 = t993.*t1508;
t1699 = -t1697;
t1701 = t1697./2.0;
t1714 = t718.*t1593;
t1725 = -t1721;
t1728 = -t1724;
t1729 = t1720./2.0;
t1742 = -t1741;
t1744 = -t1743;
t1745 = (t29.*t1732)./2.0;
t1748 = (t12.*t25.*t1732)./2.0;
t1760 = -t1758;
t1762 = qd3.*t1757;
t1765 = t1186.*t1508;
t1778 = (t1508.*(t387+t473+t478+t26.*t29.*t132.*1.383e-1))./2.0;
t1782 = t772+t1256+t1258;
t1784 = (t29.*t1775)./2.0;
t1785 = t8.*t1780;
t1788 = (t12.*t25.*t1775)./2.0;
t1794 = t994.*t1593;
t1797 = (t2.*t25.*t1780)./2.0;
t1799 = (t26.*t29.*t1780)./2.0;
t1806 = t1297.*t1508;
t1808 = -t1804;
t1814 = -t1813;
t1818 = t8.*t1816;
t1824 = (t2.*t25.*t1816)./2.0;
t1827 = (t26.*t29.*t1816)./2.0;
t1833 = t1187.*t1593;
t1834 = (t133.*t1816)./2.0;
t1837 = (t1371.*t1508)./2.0;
t1845 = (t1392.*t1508)./2.0;
t1850 = -t1846;
t1860 = t1298.*t1593;
t1861 = -t1858;
t1864 = -t1862;
t1865 = t1451.*t1508;
t1874 = -t1872;
t1877 = t1393.*t1593;
t1879 = (t25.*t1871)./2.0;
t1881 = (t12.*t29.*t1871)./2.0;
t1883 = t25.*t1880;
t1887 = t245+t746+t748+t1307+t1324;
t1889 = (t12.*t29.*t1880)./2.0;
t1892 = (t1508.*t1566)./2.0;
t1895 = -t1893;
t1897 = t1452.*t1593;
t1899 = t544+t1014+t1020+t1065+t1070;
t1901 = t545+t1011+t1064+t1066+t1071;
t1907 = t1486.*t1593;
t1911 = t1509.*t1593;
t1926 = (t1567.*t1593)./2.0;
t1934 = t1932.*(-1.0./2.0);
t1938 = t245+t746+t748+t1387+t1396;
t1947 = -t1945;
t1948 = t1945./2.0;
t1949 = t1946./2.0;
t1950 = t245+t746+t748+t1421+t1432;
t1959 = t698+t699+t1040+t1053+t1149+t1152;
t1962 = t780+t790+t1089+t1098+t1208+t1214;
t1963 = t771+t800+t1099+t1111+t1198+t1204;
t1968 = t782+t784+t1133+t1139+t1664;
t1971 = qd3.*t1970;
t1972 = t935+t936+t1134+t1138+t1807;
t1982 = t682+t920+t1284+t1285+t1467+t1471;
t1983 = t690+t910+t1275+t1277+t1472+t1478;
t1984 = t929+t932+t1199+t1201+t1866;
t1986 = t2.*(t687+t906-t1277-t1472+t1279.*(t61-t241).*8.084033333333334e-4+t7.*t132.*(t291-t477+t172.*(t60-t192)).*8.084033333333334e-4).*(-1.0./2.0);
t1990 = t8.*t1988;
t1992 = t2.*t1989;
t1996 = t132.*(t687+t906-t1277-t1472+t1279.*(t61-t241).*8.084033333333334e-4+t7.*t132.*(t291-t477+t172.*(t60-t192)).*8.084033333333334e-4).*(-1.0./2.0);
t1998 = t597+t765+t1288+t1293+t1536+t1547;
t1999 = (t2.*t29.*t1988)./2.0;
t2001 = (t8.*t29.*t1989)./2.0;
t2006 = (t172.*t1988)./2.0;
t2007 = (t132.*t1989)./2.0;
t2011 = t495+t497+t1271+t1363+t1580+t1607;
t2012 = t8.*t2010;
t2013 = t637+t833+t1302+t1322+t1560+t1572;
t2019 = (t2.*t29.*t2010)./2.0;
t2023 = t586+t587+t1266+t1360+t1580+t1607;
t2024 = (t172.*t2010)./2.0;
t2029 = t503+t504+t1266+t1360+t1581+t1597+t1607;
t2035 = t1185+t1194+t1259+t1261+t1383+t1384+t1719+t1720;
t2037 = t1235+t1241+t1321+t1326+t1383+t1384+t1719+t1720;
t2043 = t1350+t1354+t1356+t1362+t1424+t1427+t1719+t1720;
t2046 = -qd1.*(-t614+t869-t1249+t1443-t1449+t1733+t1734+(t380.*(t429-t960))./2.0+(t372.*(t446-t970))./2.0+t12.*t39.*(t291-t477+t172.*(t60-t192)).*4.042016666666667e-4);
t2047 = qd1.*(-t614+t869-t1249+t1443-t1449+t1733+t1734+(t380.*(t429-t960))./2.0+(t372.*(t446-t970))./2.0+t12.*t39.*(t291-t477+t172.*(t60-t192)).*4.042016666666667e-4);
t2052 = t613+t767+t1289+t1292+t1394+t1407+t1535+t1546+t1768+t1771;
t2057 = t613+t767+t1289+t1292+t1469+t1479+t1535+t1546+t1768+t1771;
t2064 = t613+t767+t1289+t1292+t1497+t1510+t1535+t1546+t1768+t1771;
t2067 = t1145+t1224+t1342+t1349+t1423+t1434+t1707+t1712+t1735+t1737;
t2068 = qd6.*(t1224+t1342+t1349+t1423+t1434+t1707+t1712+t1735+t1737+(t6.*t29.*t1112)./2.0);
t2069 = t1150+t1325+t1397+t1403+t1409+t1412+t1753+t1754+t1764+t1769;
t2070 = -qd6.*(t1144-t1325+t1394+t1404+t1407+t1751-t1753+t1768+t1771+(t29.*t30.*(t332+t817+t238.*(t61-t241).*8.084033333333334e-4))./2.0);
t2072 = t1150+t1325+t1409+t1412+t1470+t1474+t1753+t1754+t1764+t1769;
t2073 = -qd6.*(t1144-t1325+t1404+t1469+t1479+t1751-t1753+t1768+t1771+(t29.*t30.*(t332+t817+t238.*(t61-t241).*8.084033333333334e-4))./2.0);
t2074 = t1150+t1325+t1409+t1412+t1500+t1506+t1753+t1754+t1764+t1769;
t2075 = -qd6.*(t1144-t1325+t1404+t1497+t1510+t1751-t1753+t1768+t1771+(t29.*t30.*(t332+t817+t238.*(t61-t241).*8.084033333333334e-4))./2.0);
t2084 = t534+t547+t725+t898+t904+t956+t972+t974+t1007+t1012+t1210+t1212+t1299+t1300+t1418+t1430+t1464+t1476+t1810+t1815;
t2087 = t534+t547+t725+t898+t904+t956+t972+t974+t1082+t1090+t1210+t1212+t1299+t1300+t1464+t1476+t1487+t1496+t1810+t1815;
t2090 = t534+t547+t725+t898+t904+t956+t972+t974+t1119+t1120+t1210+t1212+t1299+t1300+t1464+t1476+t1531+t1534+t1810+t1815;
t2094 = t1530+t1573+t1575+t1634+t1635+t1805+t1936+t1953+t1954;
t1584 = t25.*t1583;
t1585 = t12.*t29.*t1583;
t1587 = (t29.*t1583)./2.0;
t1609 = -t1605;
t1630 = -t1623;
t1632 = t1623./2.0;
t1636 = -t1629;
t1639 = -t1633;
t1646 = -t1643;
t1647 = -t1644;
t1649 = -t1648;
t1655 = -t1653;
t1661 = -t1660;
t1667 = -t1665;
t1700 = t1696./2.0;
t1703 = -t1701;
t1713 = t717.*t1592;
t1718 = -t1714;
t1723 = t1714./2.0;
t1746 = -t1745;
t1750 = -t1748;
t1763 = t915.*t1592;
t1787 = -t1784;
t1789 = t6.*t1784;
t1791 = -t1785;
t1793 = t993.*t1592;
t1796 = -t1794;
t1798 = -t1797;
t1801 = -t1799;
t1825 = -t1824;
t1832 = t1186.*t1592;
t1835 = -t1834;
t1838 = -t1837;
t1842 = (t1592.*(t387+t473+t478+t26.*t29.*t132.*1.383e-1))./2.0;
t1849 = -t1845;
t1859 = t1297.*t1592;
t1869 = (t1371.*t1592)./2.0;
t1876 = t1392.*t1592;
t1878 = -t1877;
t1882 = -t1881;
t1886 = t1883./2.0;
t1890 = qd1.*t1887;
t1894 = -t1892;
t1896 = t1451.*t1592;
Yr = ft_4({qd1,qd2,qd3,qd4,qd5,qd6,qrd1,qrd2,qrd3,qrd4,qrd5,qrd6,qrdd1,qrdd2,qrdd3,qrdd4,qrdd5,qrdd6,t1007,t1009,t1012,t1013,t1015,t1016,t1017,t1018,t1019,t1022,t1025,t1030,t1032,t1035,t1041,t1043,t1046,t1048,t1049,t1050,t1051,t1052,t1056,t1059,t1067,t1076,t1077,t1078,t1079,t1082,t1083,t1085,t1086,t1087,t1088,t1089,t1090,t1091,t1096,t1097,t1101,t1102,t1103,t1104,t1107,t1109,t1112,t1113,t1116,t1118,t1119,t1120,t1121,t1122,t1123,t1124,t1125,t1126,t1128,t1129,t1130,t1131,t1132,t1133,t1134,t1135,t1137,t1138,t1139,t1140,t1141,t1144,t1146,t1147,t1148,t1153,t1154,t1155,t1156,t1164,t1167,t1168,t1169,t1171,t1176,t1177,t1180,t1183,t1184,t1185,t1186,t1187,t1190,t1192,t1194,t1197,t1199,t12,t1200,t1201,t1203,t1207,t1209,t1210,t1211,t1212,t1213,t1214,t1215,t1220,t1222,t1223,t1224,t1225,t1226,t1227,t1228,t1229,t1232,t1234,t1235,t1237,t1238,t1239,t1241,t1242,t1243,t1244,t1245,t1246,t1247,t1248,t1249,t1250,t1253,t1257,t1259,t1260,t1263,t1265,t1266,t1267,t1268,t1269,t127,t1270,t1272,t1273,t1277,t1278,t1279,t1283,t1285,t1286,t1290,t1294,t1295,t1296,t1299,t1300,t1303,t1304,t1305,t1306,t1312,t1313,t1316,t1317,t1319,t132,t1320,t1321,t1323,t1325,t133,t1331,t1332,t1336,t1337,t1340,t1341,t1342,t1344,t1346,t1347,t1349,t1350,t1353,t1354,t1355,t1356,t1358,t1359,t1360,t1361,t1364,t1365,t1366,t1367,t1368,t1369,t1370,t1371,t1372,t1375,t1376,t1377,t1378,t1379,t1380,t1381,t1383,t1384,t1385,t1391,t1392,t1393,t1394,t1398,t1400,t1401,t1402,t1404,t1406,t1407,t1408,t1411,t1413,t1414,t1416,t1417,t1418,t1420,t1423,t1424,t1427,t1428,t1429,t1430,t1434,t1435,t1436,t1438,t1439,t144,t1440,t1441,t1442,t1443,t1445,t1447,t1448,t1449,t1450,t1451,t1452,t1454,t1457,t1459,t1460,t1461,t1462,t1463,t1466,t1467,t1468,t1469,t1472,t1473,t1475,t1479,t1480,t1481,t1482,t1483,t1484,t1485,t1486,t1487,t1488,t1491,t1493,t1494,t1496,t1497,t1499,t15,t1501,t1502,t1504,t1507,t1508,t1509,t1510,t1513,t1514,t1515,t1516,t1517,t1518,t1520,t1522,t1523,t1524,t1525,t1526,t1528,t1529,t1531,t1533,t1534,t1537,t1538,t1539,t1540,t1541,t1542,t1543,t1544,t1545,t1548,t1549,t1550,t1551,t1552,t1553,t1554,t1558,t1561,t1562,t1564,t1566,t1567,t1568,t1569,t1571,t1577,t1578,t1579,t1580,t1581,t1582,t1583,t1584,t1585,t1587,t1591,t1592,t1593,t1595,t1596,t1597,t1598,t1600,t1601,t1602,t1603,t1604,t1607,t1608,t1609,t1610,t1611,t1612,t1613,t1614,t1615,t1617,t1621,t1622,t1623,t1625,t1626,t1627,t1630,t1631,t1632,t1636,t1637,t1639,t1640,t1642,t1643,t1646,t1647,t1648,t1649,t1651,t1652,t1653,t1654,t1655,t1656,t1657,t1658,t1659,t1660,t1661,t1662,t1664,t1665,t1666,t1667,t1668,t1669,t1670,t1671,t1672,t1674,t1677,t1678,t1679,t1680,t1681,t1682,t1683,t1684,t1685,t1686,t1687,t1688,t1689,t1690,t1691,t1692,t1693,t1694,t1695,t1696,t1698,t1699,t17,t170,t1700,t1701,t1703,t1704,t1706,t1707,t1708,t171,t1711,t1712,t1713,t1716,t1718,t1719,t172,t1720,t1721,t1723,t1725,t1728,t1729,t1730,t1731,t1732,t1733,t1734,t1735,t1736,t1737,t1738,t1739,t1740,t1741,t1742,t1743,t1744,t1745,t1746,t1747,t1748,t1749,t1750,t1751,t1752,t1753,t1755,t1756,t1757,t1758,t1759,t1760,t1761,t1762,t1763,t1765,t1766,t1767,t1768,t1770,t1771,t1772,t1774,t1775,t1776,t1777,t1778,t1779,t1780,t1781,t1783,t1784,t1786,t1787,t1788,t1789,t179,t1790,t1791,t1793,t1795,t1796,t1797,t1798,t1799,t18,t180,t1800,t1801,t1802,t1803,t1804,t1806,t1808,t1809,t1810,t1811,t1812,t1813,t1814,t1815,t1816,t1818,t1820,t1821,t1822,t1823,t1824,t1825,t1826,t1827,t1828,t1830,t1831,t1832,t1833,t1834,t1835,t1836,t1837,t1838,t1839,t1840,t1842,t1844,t1845,t1846,t1847,t1848,t1849,t1850,t1851,t1852,t1853,t1854,t1855,t1856,t1857,t1858,t1859,t1860,t1861,t1862,t1863,t1864,t1865,t1867,t1868,t1869,t1872,t1873,t1874,t1875,t1876,t1877,t1878,t1879,t1881,t1882,t1883,t1884,t1885,t1886,t1887,t1889,t1890,t1892,t1893,t1894,t1895,t1896,t1897,t1898,t1899,t1900,t1901,t1907,t1911,t1914,t1916,t1918,t192,t1922,t1923,t1924,t1926,t1927,t1930,t1933,t1934,t1937,t1938,t194,t1941,t1942,t1946,t1947,t1948,t1949,t1950,t1956,t1957,t1959,t1960,t1961,t1963,t1964,t1966,t1967,t1968,t1970,t1971,t1972,t1979,t1980,t1981,t1984,t1985,t1986,t1990,t1992,t1996,t1997,t1998,t1999,t2,t20,t2001,t2006,t2007,t2012,t2015,t2017,t2018,t2019,t2021,t2022,t2024,t2025,t2027,t2028,t2029,t2030,t2035,t2037,t2043,t2046,t2051,t2052,t2056,t2057,t2061,t2064,t2068,t2070,t2071,t2073,t2075,t2078,t2079,t2084,t2087,t2090,t2094,t213,t214,t215,t216,t222,t230,t231,t238,t241,t243,t25,t253,t257,t258,t26,t261,t263,t266,t267,t269,t270,t276,t277,t279,t29,t291,t294,t295,t298,t3,t30,t301,t302,t31,t326,t331,t332,t334,t337,t338,t345,t346,t347,t348,t35,t350,t352,t356,t358,t36,t363,t372,t373,t377,t379,t380,t382,t385,t387,t39,t396,t40,t403,t408,t409,t422,t423,t424,t426,t429,t432,t435,t444,t445,t446,t452,t453,t456,t473,t477,t478,t480,t491,t496,t500,t503,t504,t507,t513,t514,t523,t529,t533,t534,t535,t547,t551,t552,t553,t554,t561,t567,t568,t569,t570,t574,t575,t580,t589,t590,t592,t595,t596,t598,t6,t60,t600,t602,t604,t609,t61,t612,t614,t615,t63,t630,t639,t657,t660,t661,t663,t664,t666,t667,t668,t675,t676,t679,t68,t683,t684,t687,t689,t691,t696,t697,t7,t704,t706,t709,t71,t712,t714,t719,t720,t722,t723,t725,t726,t727,t75,t755,t763,t766,t773,t775,t776,t777,t778,t779,t781,t782,t783,t784,t785,t787,t789,t790,t791,t795,t797,t799,t8,t801,t802,t803,t804,t810,t811,t812,t813,t817,t818,t819,t845,t848,t853,t854,t859,t860,t863,t864,t868,t869,t871,t872,t874,t877,t880,t881,t886,t887,t888,t891,t892,t896,t898,t9,t904,t906,t907,t908,t909,t913,t914,t915,t921,t922,t923,t933,t934,t937,t940,t941,t943,t945,t947,t948,t950,t953,t954,t955,t956,t958,t959,t960,t964,t966,t969,t970,t972,t974,t978,t981,t985,t990,t992,t993,t994,t996});
end
function Yr = ft_4(ct)
qd1 = ct{1};
qd2 = ct{2};
qd3 = ct{3};
qd4 = ct{4};
qd5 = ct{5};
qd6 = ct{6};
qrd1 = ct{7};
qrd2 = ct{8};
qrd3 = ct{9};
qrd4 = ct{10};
qrd5 = ct{11};
qrd6 = ct{12};
qrdd1 = ct{13};
qrdd2 = ct{14};
qrdd3 = ct{15};
qrdd4 = ct{16};
qrdd5 = ct{17};
qrdd6 = ct{18};
t1007 = ct{19};
t1009 = ct{20};
t1012 = ct{21};
t1013 = ct{22};
t1015 = ct{23};
t1016 = ct{24};
t1017 = ct{25};
t1018 = ct{26};
t1019 = ct{27};
t1022 = ct{28};
t1025 = ct{29};
t1030 = ct{30};
t1032 = ct{31};
t1035 = ct{32};
t1041 = ct{33};
t1043 = ct{34};
t1046 = ct{35};
t1048 = ct{36};
t1049 = ct{37};
t1050 = ct{38};
t1051 = ct{39};
t1052 = ct{40};
t1056 = ct{41};
t1059 = ct{42};
t1067 = ct{43};
t1076 = ct{44};
t1077 = ct{45};
t1078 = ct{46};
t1079 = ct{47};
t1082 = ct{48};
t1083 = ct{49};
t1085 = ct{50};
t1086 = ct{51};
t1087 = ct{52};
t1088 = ct{53};
t1089 = ct{54};
t1090 = ct{55};
t1091 = ct{56};
t1096 = ct{57};
t1097 = ct{58};
t1101 = ct{59};
t1102 = ct{60};
t1103 = ct{61};
t1104 = ct{62};
t1107 = ct{63};
t1109 = ct{64};
t1112 = ct{65};
t1113 = ct{66};
t1116 = ct{67};
t1118 = ct{68};
t1119 = ct{69};
t1120 = ct{70};
t1121 = ct{71};
t1122 = ct{72};
t1123 = ct{73};
t1124 = ct{74};
t1125 = ct{75};
t1126 = ct{76};
t1128 = ct{77};
t1129 = ct{78};
t1130 = ct{79};
t1131 = ct{80};
t1132 = ct{81};
t1133 = ct{82};
t1134 = ct{83};
t1135 = ct{84};
t1137 = ct{85};
t1138 = ct{86};
t1139 = ct{87};
t1140 = ct{88};
t1141 = ct{89};
t1144 = ct{90};
t1146 = ct{91};
t1147 = ct{92};
t1148 = ct{93};
t1153 = ct{94};
t1154 = ct{95};
t1155 = ct{96};
t1156 = ct{97};
t1164 = ct{98};
t1167 = ct{99};
t1168 = ct{100};
t1169 = ct{101};
t1171 = ct{102};
t1176 = ct{103};
t1177 = ct{104};
t1180 = ct{105};
t1183 = ct{106};
t1184 = ct{107};
t1185 = ct{108};
t1186 = ct{109};
t1187 = ct{110};
t1190 = ct{111};
t1192 = ct{112};
t1194 = ct{113};
t1197 = ct{114};
t1199 = ct{115};
t12 = ct{116};
t1200 = ct{117};
t1201 = ct{118};
t1203 = ct{119};
t1207 = ct{120};
t1209 = ct{121};
t1210 = ct{122};
t1211 = ct{123};
t1212 = ct{124};
t1213 = ct{125};
t1214 = ct{126};
t1215 = ct{127};
t1220 = ct{128};
t1222 = ct{129};
t1223 = ct{130};
t1224 = ct{131};
t1225 = ct{132};
t1226 = ct{133};
t1227 = ct{134};
t1228 = ct{135};
t1229 = ct{136};
t1232 = ct{137};
t1234 = ct{138};
t1235 = ct{139};
t1237 = ct{140};
t1238 = ct{141};
t1239 = ct{142};
t1241 = ct{143};
t1242 = ct{144};
t1243 = ct{145};
t1244 = ct{146};
t1245 = ct{147};
t1246 = ct{148};
t1247 = ct{149};
t1248 = ct{150};
t1249 = ct{151};
t1250 = ct{152};
t1253 = ct{153};
t1257 = ct{154};
t1259 = ct{155};
t1260 = ct{156};
t1263 = ct{157};
t1265 = ct{158};
t1266 = ct{159};
t1267 = ct{160};
t1268 = ct{161};
t1269 = ct{162};
t127 = ct{163};
t1270 = ct{164};
t1272 = ct{165};
t1273 = ct{166};
t1277 = ct{167};
t1278 = ct{168};
t1279 = ct{169};
t1283 = ct{170};
t1285 = ct{171};
t1286 = ct{172};
t1290 = ct{173};
t1294 = ct{174};
t1295 = ct{175};
t1296 = ct{176};
t1299 = ct{177};
t1300 = ct{178};
t1303 = ct{179};
t1304 = ct{180};
t1305 = ct{181};
t1306 = ct{182};
t1312 = ct{183};
t1313 = ct{184};
t1316 = ct{185};
t1317 = ct{186};
t1319 = ct{187};
t132 = ct{188};
t1320 = ct{189};
t1321 = ct{190};
t1323 = ct{191};
t1325 = ct{192};
t133 = ct{193};
t1331 = ct{194};
t1332 = ct{195};
t1336 = ct{196};
t1337 = ct{197};
t1340 = ct{198};
t1341 = ct{199};
t1342 = ct{200};
t1344 = ct{201};
t1346 = ct{202};
t1347 = ct{203};
t1349 = ct{204};
t1350 = ct{205};
t1353 = ct{206};
t1354 = ct{207};
t1355 = ct{208};
t1356 = ct{209};
t1358 = ct{210};
t1359 = ct{211};
t1360 = ct{212};
t1361 = ct{213};
t1364 = ct{214};
t1365 = ct{215};
t1366 = ct{216};
t1367 = ct{217};
t1368 = ct{218};
t1369 = ct{219};
t1370 = ct{220};
t1371 = ct{221};
t1372 = ct{222};
t1375 = ct{223};
t1376 = ct{224};
t1377 = ct{225};
t1378 = ct{226};
t1379 = ct{227};
t1380 = ct{228};
t1381 = ct{229};
t1383 = ct{230};
t1384 = ct{231};
t1385 = ct{232};
t1391 = ct{233};
t1392 = ct{234};
t1393 = ct{235};
t1394 = ct{236};
t1398 = ct{237};
t1400 = ct{238};
t1401 = ct{239};
t1402 = ct{240};
t1404 = ct{241};
t1406 = ct{242};
t1407 = ct{243};
t1408 = ct{244};
t1411 = ct{245};
t1413 = ct{246};
t1414 = ct{247};
t1416 = ct{248};
t1417 = ct{249};
t1418 = ct{250};
t1420 = ct{251};
t1423 = ct{252};
t1424 = ct{253};
t1427 = ct{254};
t1428 = ct{255};
t1429 = ct{256};
t1430 = ct{257};
t1434 = ct{258};
t1435 = ct{259};
t1436 = ct{260};
t1438 = ct{261};
t1439 = ct{262};
t144 = ct{263};
t1440 = ct{264};
t1441 = ct{265};
t1442 = ct{266};
t1443 = ct{267};
t1445 = ct{268};
t1447 = ct{269};
t1448 = ct{270};
t1449 = ct{271};
t1450 = ct{272};
t1451 = ct{273};
t1452 = ct{274};
t1454 = ct{275};
t1457 = ct{276};
t1459 = ct{277};
t1460 = ct{278};
t1461 = ct{279};
t1462 = ct{280};
t1463 = ct{281};
t1466 = ct{282};
t1467 = ct{283};
t1468 = ct{284};
t1469 = ct{285};
t1472 = ct{286};
t1473 = ct{287};
t1475 = ct{288};
t1479 = ct{289};
t1480 = ct{290};
t1481 = ct{291};
t1482 = ct{292};
t1483 = ct{293};
t1484 = ct{294};
t1485 = ct{295};
t1486 = ct{296};
t1487 = ct{297};
t1488 = ct{298};
t1491 = ct{299};
t1493 = ct{300};
t1494 = ct{301};
t1496 = ct{302};
t1497 = ct{303};
t1499 = ct{304};
t15 = ct{305};
t1501 = ct{306};
t1502 = ct{307};
t1504 = ct{308};
t1507 = ct{309};
t1508 = ct{310};
t1509 = ct{311};
t1510 = ct{312};
t1513 = ct{313};
t1514 = ct{314};
t1515 = ct{315};
t1516 = ct{316};
t1517 = ct{317};
t1518 = ct{318};
t1520 = ct{319};
t1522 = ct{320};
t1523 = ct{321};
t1524 = ct{322};
t1525 = ct{323};
t1526 = ct{324};
t1528 = ct{325};
t1529 = ct{326};
t1531 = ct{327};
t1533 = ct{328};
t1534 = ct{329};
t1537 = ct{330};
t1538 = ct{331};
t1539 = ct{332};
t1540 = ct{333};
t1541 = ct{334};
t1542 = ct{335};
t1543 = ct{336};
t1544 = ct{337};
t1545 = ct{338};
t1548 = ct{339};
t1549 = ct{340};
t1550 = ct{341};
t1551 = ct{342};
t1552 = ct{343};
t1553 = ct{344};
t1554 = ct{345};
t1558 = ct{346};
t1561 = ct{347};
t1562 = ct{348};
t1564 = ct{349};
t1566 = ct{350};
t1567 = ct{351};
t1568 = ct{352};
t1569 = ct{353};
t1571 = ct{354};
t1577 = ct{355};
t1578 = ct{356};
t1579 = ct{357};
t1580 = ct{358};
t1581 = ct{359};
t1582 = ct{360};
t1583 = ct{361};
t1584 = ct{362};
t1585 = ct{363};
t1587 = ct{364};
t1591 = ct{365};
t1592 = ct{366};
t1593 = ct{367};
t1595 = ct{368};
t1596 = ct{369};
t1597 = ct{370};
t1598 = ct{371};
t1600 = ct{372};
t1601 = ct{373};
t1602 = ct{374};
t1603 = ct{375};
t1604 = ct{376};
t1607 = ct{377};
t1608 = ct{378};
t1609 = ct{379};
t1610 = ct{380};
t1611 = ct{381};
t1612 = ct{382};
t1613 = ct{383};
t1614 = ct{384};
t1615 = ct{385};
t1617 = ct{386};
t1621 = ct{387};
t1622 = ct{388};
t1623 = ct{389};
t1625 = ct{390};
t1626 = ct{391};
t1627 = ct{392};
t1630 = ct{393};
t1631 = ct{394};
t1632 = ct{395};
t1636 = ct{396};
t1637 = ct{397};
t1639 = ct{398};
t1640 = ct{399};
t1642 = ct{400};
t1643 = ct{401};
t1646 = ct{402};
t1647 = ct{403};
t1648 = ct{404};
t1649 = ct{405};
t1651 = ct{406};
t1652 = ct{407};
t1653 = ct{408};
t1654 = ct{409};
t1655 = ct{410};
t1656 = ct{411};
t1657 = ct{412};
t1658 = ct{413};
t1659 = ct{414};
t1660 = ct{415};
t1661 = ct{416};
t1662 = ct{417};
t1664 = ct{418};
t1665 = ct{419};
t1666 = ct{420};
t1667 = ct{421};
t1668 = ct{422};
t1669 = ct{423};
t1670 = ct{424};
t1671 = ct{425};
t1672 = ct{426};
t1674 = ct{427};
t1677 = ct{428};
t1678 = ct{429};
t1679 = ct{430};
t1680 = ct{431};
t1681 = ct{432};
t1682 = ct{433};
t1683 = ct{434};
t1684 = ct{435};
t1685 = ct{436};
t1686 = ct{437};
t1687 = ct{438};
t1688 = ct{439};
t1689 = ct{440};
t1690 = ct{441};
t1691 = ct{442};
t1692 = ct{443};
t1693 = ct{444};
t1694 = ct{445};
t1695 = ct{446};
t1696 = ct{447};
t1698 = ct{448};
t1699 = ct{449};
t17 = ct{450};
t170 = ct{451};
t1700 = ct{452};
t1701 = ct{453};
t1703 = ct{454};
t1704 = ct{455};
t1706 = ct{456};
t1707 = ct{457};
t1708 = ct{458};
t171 = ct{459};
t1711 = ct{460};
t1712 = ct{461};
t1713 = ct{462};
t1716 = ct{463};
t1718 = ct{464};
t1719 = ct{465};
t172 = ct{466};
t1720 = ct{467};
t1721 = ct{468};
t1723 = ct{469};
t1725 = ct{470};
t1728 = ct{471};
t1729 = ct{472};
t1730 = ct{473};
t1731 = ct{474};
t1732 = ct{475};
t1733 = ct{476};
t1734 = ct{477};
t1735 = ct{478};
t1736 = ct{479};
t1737 = ct{480};
t1738 = ct{481};
t1739 = ct{482};
t1740 = ct{483};
t1741 = ct{484};
t1742 = ct{485};
t1743 = ct{486};
t1744 = ct{487};
t1745 = ct{488};
t1746 = ct{489};
t1747 = ct{490};
t1748 = ct{491};
t1749 = ct{492};
t1750 = ct{493};
t1751 = ct{494};
t1752 = ct{495};
t1753 = ct{496};
t1755 = ct{497};
t1756 = ct{498};
t1757 = ct{499};
t1758 = ct{500};
t1759 = ct{501};
t1760 = ct{502};
t1761 = ct{503};
t1762 = ct{504};
t1763 = ct{505};
t1765 = ct{506};
t1766 = ct{507};
t1767 = ct{508};
t1768 = ct{509};
t1770 = ct{510};
t1771 = ct{511};
t1772 = ct{512};
t1774 = ct{513};
t1775 = ct{514};
t1776 = ct{515};
t1777 = ct{516};
t1778 = ct{517};
t1779 = ct{518};
t1780 = ct{519};
t1781 = ct{520};
t1783 = ct{521};
t1784 = ct{522};
t1786 = ct{523};
t1787 = ct{524};
t1788 = ct{525};
t1789 = ct{526};
t179 = ct{527};
t1790 = ct{528};
t1791 = ct{529};
t1793 = ct{530};
t1795 = ct{531};
t1796 = ct{532};
t1797 = ct{533};
t1798 = ct{534};
t1799 = ct{535};
t18 = ct{536};
t180 = ct{537};
t1800 = ct{538};
t1801 = ct{539};
t1802 = ct{540};
t1803 = ct{541};
t1804 = ct{542};
t1806 = ct{543};
t1808 = ct{544};
t1809 = ct{545};
t1810 = ct{546};
t1811 = ct{547};
t1812 = ct{548};
t1813 = ct{549};
t1814 = ct{550};
t1815 = ct{551};
t1816 = ct{552};
t1818 = ct{553};
t1820 = ct{554};
t1821 = ct{555};
t1822 = ct{556};
t1823 = ct{557};
t1824 = ct{558};
t1825 = ct{559};
t1826 = ct{560};
t1827 = ct{561};
t1828 = ct{562};
t1830 = ct{563};
t1831 = ct{564};
t1832 = ct{565};
t1833 = ct{566};
t1834 = ct{567};
t1835 = ct{568};
t1836 = ct{569};
t1837 = ct{570};
t1838 = ct{571};
t1839 = ct{572};
t1840 = ct{573};
t1842 = ct{574};
t1844 = ct{575};
t1845 = ct{576};
t1846 = ct{577};
t1847 = ct{578};
t1848 = ct{579};
t1849 = ct{580};
t1850 = ct{581};
t1851 = ct{582};
t1852 = ct{583};
t1853 = ct{584};
t1854 = ct{585};
t1855 = ct{586};
t1856 = ct{587};
t1857 = ct{588};
t1858 = ct{589};
t1859 = ct{590};
t1860 = ct{591};
t1861 = ct{592};
t1862 = ct{593};
t1863 = ct{594};
t1864 = ct{595};
t1865 = ct{596};
t1867 = ct{597};
t1868 = ct{598};
t1869 = ct{599};
t1872 = ct{600};
t1873 = ct{601};
t1874 = ct{602};
t1875 = ct{603};
t1876 = ct{604};
t1877 = ct{605};
t1878 = ct{606};
t1879 = ct{607};
t1881 = ct{608};
t1882 = ct{609};
t1883 = ct{610};
t1884 = ct{611};
t1885 = ct{612};
t1886 = ct{613};
t1887 = ct{614};
t1889 = ct{615};
t1890 = ct{616};
t1892 = ct{617};
t1893 = ct{618};
t1894 = ct{619};
t1895 = ct{620};
t1896 = ct{621};
t1897 = ct{622};
t1898 = ct{623};
t1899 = ct{624};
t1900 = ct{625};
t1901 = ct{626};
t1907 = ct{627};
t1911 = ct{628};
t1914 = ct{629};
t1916 = ct{630};
t1918 = ct{631};
t192 = ct{632};
t1922 = ct{633};
t1923 = ct{634};
t1924 = ct{635};
t1926 = ct{636};
t1927 = ct{637};
t1930 = ct{638};
t1933 = ct{639};
t1934 = ct{640};
t1937 = ct{641};
t1938 = ct{642};
t194 = ct{643};
t1941 = ct{644};
t1942 = ct{645};
t1946 = ct{646};
t1947 = ct{647};
t1948 = ct{648};
t1949 = ct{649};
t1950 = ct{650};
t1956 = ct{651};
t1957 = ct{652};
t1959 = ct{653};
t1960 = ct{654};
t1961 = ct{655};
t1963 = ct{656};
t1964 = ct{657};
t1966 = ct{658};
t1967 = ct{659};
t1968 = ct{660};
t1970 = ct{661};
t1971 = ct{662};
t1972 = ct{663};
t1979 = ct{664};
t1980 = ct{665};
t1981 = ct{666};
t1984 = ct{667};
t1985 = ct{668};
t1986 = ct{669};
t1990 = ct{670};
t1992 = ct{671};
t1996 = ct{672};
t1997 = ct{673};
t1998 = ct{674};
t1999 = ct{675};
t2 = ct{676};
t20 = ct{677};
t2001 = ct{678};
t2006 = ct{679};
t2007 = ct{680};
t2012 = ct{681};
t2015 = ct{682};
t2017 = ct{683};
t2018 = ct{684};
t2019 = ct{685};
t2021 = ct{686};
t2022 = ct{687};
t2024 = ct{688};
t2025 = ct{689};
t2027 = ct{690};
t2028 = ct{691};
t2029 = ct{692};
t2030 = ct{693};
t2035 = ct{694};
t2037 = ct{695};
t2043 = ct{696};
t2046 = ct{697};
t2051 = ct{698};
t2052 = ct{699};
t2056 = ct{700};
t2057 = ct{701};
t2061 = ct{702};
t2064 = ct{703};
t2068 = ct{704};
t2070 = ct{705};
t2071 = ct{706};
t2073 = ct{707};
t2075 = ct{708};
t2078 = ct{709};
t2079 = ct{710};
t2084 = ct{711};
t2087 = ct{712};
t2090 = ct{713};
t2094 = ct{714};
t213 = ct{715};
t214 = ct{716};
t215 = ct{717};
t216 = ct{718};
t222 = ct{719};
t230 = ct{720};
t231 = ct{721};
t238 = ct{722};
t241 = ct{723};
t243 = ct{724};
t25 = ct{725};
t253 = ct{726};
t257 = ct{727};
t258 = ct{728};
t26 = ct{729};
t261 = ct{730};
t263 = ct{731};
t266 = ct{732};
t267 = ct{733};
t269 = ct{734};
t270 = ct{735};
t276 = ct{736};
t277 = ct{737};
t279 = ct{738};
t29 = ct{739};
t291 = ct{740};
t294 = ct{741};
t295 = ct{742};
t298 = ct{743};
t3 = ct{744};
t30 = ct{745};
t301 = ct{746};
t302 = ct{747};
t31 = ct{748};
t326 = ct{749};
t331 = ct{750};
t332 = ct{751};
t334 = ct{752};
t337 = ct{753};
t338 = ct{754};
t345 = ct{755};
t346 = ct{756};
t347 = ct{757};
t348 = ct{758};
t35 = ct{759};
t350 = ct{760};
t352 = ct{761};
t356 = ct{762};
t358 = ct{763};
t36 = ct{764};
t363 = ct{765};
t372 = ct{766};
t373 = ct{767};
t377 = ct{768};
t379 = ct{769};
t380 = ct{770};
t382 = ct{771};
t385 = ct{772};
t387 = ct{773};
t39 = ct{774};
t396 = ct{775};
t40 = ct{776};
t403 = ct{777};
t408 = ct{778};
t409 = ct{779};
t422 = ct{780};
t423 = ct{781};
t424 = ct{782};
t426 = ct{783};
t429 = ct{784};
t432 = ct{785};
t435 = ct{786};
t444 = ct{787};
t445 = ct{788};
t446 = ct{789};
t452 = ct{790};
t453 = ct{791};
t456 = ct{792};
t473 = ct{793};
t477 = ct{794};
t478 = ct{795};
t480 = ct{796};
t491 = ct{797};
t496 = ct{798};
t500 = ct{799};
t503 = ct{800};
t504 = ct{801};
t507 = ct{802};
t513 = ct{803};
t514 = ct{804};
t523 = ct{805};
t529 = ct{806};
t533 = ct{807};
t534 = ct{808};
t535 = ct{809};
t547 = ct{810};
t551 = ct{811};
t552 = ct{812};
t553 = ct{813};
t554 = ct{814};
t561 = ct{815};
t567 = ct{816};
t568 = ct{817};
t569 = ct{818};
t570 = ct{819};
t574 = ct{820};
t575 = ct{821};
t580 = ct{822};
t589 = ct{823};
t590 = ct{824};
t592 = ct{825};
t595 = ct{826};
t596 = ct{827};
t598 = ct{828};
t6 = ct{829};
t60 = ct{830};
t600 = ct{831};
t602 = ct{832};
t604 = ct{833};
t609 = ct{834};
t61 = ct{835};
t612 = ct{836};
t614 = ct{837};
t615 = ct{838};
t63 = ct{839};
t630 = ct{840};
t639 = ct{841};
t657 = ct{842};
t660 = ct{843};
t661 = ct{844};
t663 = ct{845};
t664 = ct{846};
t666 = ct{847};
t667 = ct{848};
t668 = ct{849};
t675 = ct{850};
t676 = ct{851};
t679 = ct{852};
t68 = ct{853};
t683 = ct{854};
t684 = ct{855};
t687 = ct{856};
t689 = ct{857};
t691 = ct{858};
t696 = ct{859};
t697 = ct{860};
t7 = ct{861};
t704 = ct{862};
t706 = ct{863};
t709 = ct{864};
t71 = ct{865};
t712 = ct{866};
t714 = ct{867};
t719 = ct{868};
t720 = ct{869};
t722 = ct{870};
t723 = ct{871};
t725 = ct{872};
t726 = ct{873};
t727 = ct{874};
t75 = ct{875};
t755 = ct{876};
t763 = ct{877};
t766 = ct{878};
t773 = ct{879};
t775 = ct{880};
t776 = ct{881};
t777 = ct{882};
t778 = ct{883};
t779 = ct{884};
t781 = ct{885};
t782 = ct{886};
t783 = ct{887};
t784 = ct{888};
t785 = ct{889};
t787 = ct{890};
t789 = ct{891};
t790 = ct{892};
t791 = ct{893};
t795 = ct{894};
t797 = ct{895};
t799 = ct{896};
t8 = ct{897};
t801 = ct{898};
t802 = ct{899};
t803 = ct{900};
t804 = ct{901};
t810 = ct{902};
t811 = ct{903};
t812 = ct{904};
t813 = ct{905};
t817 = ct{906};
t818 = ct{907};
t819 = ct{908};
t845 = ct{909};
t848 = ct{910};
t853 = ct{911};
t854 = ct{912};
t859 = ct{913};
t860 = ct{914};
t863 = ct{915};
t864 = ct{916};
t868 = ct{917};
t869 = ct{918};
t871 = ct{919};
t872 = ct{920};
t874 = ct{921};
t877 = ct{922};
t880 = ct{923};
t881 = ct{924};
t886 = ct{925};
t887 = ct{926};
t888 = ct{927};
t891 = ct{928};
t892 = ct{929};
t896 = ct{930};
t898 = ct{931};
t9 = ct{932};
t904 = ct{933};
t906 = ct{934};
t907 = ct{935};
t908 = ct{936};
t909 = ct{937};
t913 = ct{938};
t914 = ct{939};
t915 = ct{940};
t921 = ct{941};
t922 = ct{942};
t923 = ct{943};
t933 = ct{944};
t934 = ct{945};
t937 = ct{946};
t940 = ct{947};
t941 = ct{948};
t943 = ct{949};
t945 = ct{950};
t947 = ct{951};
t948 = ct{952};
t950 = ct{953};
t953 = ct{954};
t954 = ct{955};
t955 = ct{956};
t956 = ct{957};
t958 = ct{958};
t959 = ct{959};
t960 = ct{960};
t964 = ct{961};
t966 = ct{962};
t969 = ct{963};
t970 = ct{964};
t972 = ct{965};
t974 = ct{966};
t978 = ct{967};
t981 = ct{968};
t985 = ct{969};
t990 = ct{970};
t992 = ct{971};
t993 = ct{972};
t994 = ct{973};
t996 = ct{974};
t1902 = (t8.*t1899)./2.0;
t1903 = (t2.*t1901)./2.0;
t1904 = (t2.*t29.*t1899)./2.0;
t1906 = t1485.*t1592;
t1908 = (t8.*t29.*t1901)./2.0;
t1909 = -t1907;
t1910 = t1508.*t1592;
t1912 = (t172.*t1899)./2.0;
t1915 = (t132.*t1901)./2.0;
t1925 = (t1566.*t1592)./2.0;
t1929 = -t1926;
t1939 = qd1.*t1938;
t1951 = -t1948;
t1952 = qd1.*t1950;
t1965 = (t2.*t1963)./2.0;
t1969 = t859+t860+t1133+t1139+t1699;
t1973 = qd3.*t1972;
t1975 = t598+t868+t1248+t1250+t1447+t1450;
t1987 = t775+t776+t1199+t1201+t1897;
t1991 = -t1990;
t1993 = t1990./2.0;
t1995 = t1992./2.0;
t2000 = -t1999;
t2002 = -t2001;
t2003 = (t25.*t1998)./2.0;
t2005 = (t12.*t29.*t1998)./2.0;
t2008 = -t2006;
t2009 = t853+t854+t1199+t1201+t1911;
t2014 = t2012./2.0;
t2020 = -t2019;
t2026 = t533+t943+t964+t1035+t1043+t1728+t1729;
t2031 = t1364+t1365+t1621+t1622+t1865;
t2045 = t614+t874+t1247+t1249+t1342+t1349+t1448+t1449+t1735+t1737;
t2048 = t801+t803+t1134+t1138+t1666+t1701+t1850+t1863;
t2053 = qd1.*t2052;
t2058 = qd1.*t2057;
t2062 = t1708+t1716+t1736+t1740+t1744+t1778;
t2063 = -qd6.*(t1706+t1711-t1736+t1743-t1778+(t8.*t914.*(t263+t456-t922-t978))./2.0);
t2065 = qd1.*t2064;
t2085 = qd1.*t2084;
t2088 = qd1.*t2087;
t2091 = qd1.*t2090;
t2095 = t1013+t1015+t1137+t1290+t1296+t1316+t1401+t1406+t1418+t1430+t1691+t1692+t1739+t1742+t1810+t1815;
t2096 = t1088+t1097+t1137+t1290+t1296+t1316+t1401+t1406+t1487+t1496+t1691+t1692+t1739+t1742+t1810+t1815;
t2097 = t1121+t1124+t1137+t1290+t1296+t1316+t1401+t1406+t1531+t1534+t1691+t1692+t1739+t1742+t1810+t1815;
t2099 = t1286+t1359+t1361+t1459+t1460+t2094;
t2102 = t1484+t1494+t1569+t1706+t1711+t1736+t1740+t1743+t1778+t2012+t2015;
et1 = t1313+t1613+t1653+t1660-t1672+t1725+t1748+t1799+t1813+t1821+t1823+t1847+t1848-t1889+t2006-t2007+(t132.*(t590+t600-t958-t1017-t1018+t453.*(t61-t241).*8.084033333333334e-4))./2.0+(t172.*(t589+t602-t953-t1030-t1032+t452.*(t60-t192).*8.084033333333334e-4))./2.0;
et2 = (t12.*t29.*(t697+t945-t1211-t1213+t194.*(-t270-t294+t334+t337+t396+t2.*t25.*(t60-t192)).*8.084033333333334e-4+t238.*(-t269-t295+t352+t356+t385+t8.*t25.*(t61-t241)).*8.084033333333334e-4))./2.0+(t2.*t863.*(t444-t445-t639+t969))./2.0-(t6.*t29.*t1583)./2.0;
et3 = (t29.*t30.*(t779+t1253+t907.*(t61-t241).*8.084033333333334e-4))./2.0+(t2.*t491.*(t429-t960))./2.0+(t8.*t491.*(t446-t970))./2.0;
t2123 = -qd6.*(et1+et2+et3);
et4 = t1313+t1613+t1653+t1660-t1688+t1725+t1748+t1799+t1821+t1823+t1837+t1847+t1848-t1889+t2006-t2007+(t132.*(t590+t600-t958-t1017-t1018+t453.*(t61-t241).*8.084033333333334e-4))./2.0+(t172.*(t589+t602-t953-t1030-t1032+t452.*(t60-t192).*8.084033333333334e-4))./2.0;
et5 = (t12.*t29.*(t697+t945-t1211-t1213+t194.*(-t270-t294+t334+t337+t396+t2.*t25.*(t60-t192)).*8.084033333333334e-4+t238.*(-t269-t295+t352+t356+t385+t8.*t25.*(t61-t241)).*8.084033333333334e-4))./2.0+(t2.*t914.*(t444-t445-t639+t969))./2.0-(t6.*t29.*t1583)./2.0;
et6 = (t29.*t30.*(t779+t1253+t907.*(t61-t241).*8.084033333333334e-4))./2.0+(t2.*t491.*(t429-t960))./2.0+(t8.*t491.*(t446-t970))./2.0;
t2125 = -qd6.*(et4+et5+et6);
t1586 = -t1584;
t1588 = -t1587;
t1589 = (t12.*t1584)./2.0;
t1590 = t6.*t1587;
t1638 = -t1632;
t1702 = -t1700;
t1717 = -t1713;
t1722 = t1713./2.0;
t1727 = -t1723;
t1843 = -t1842;
t1870 = -t1869;
t1888 = -t1886;
t1891 = -t1890;
t1905 = -t1903;
t1913 = -t1912;
t1917 = -t1915;
t1928 = -t1925;
t1940 = -t1939;
t1955 = -t1952;
t1974 = t683+t684+t1133+t1139+t1878;
t1976 = (t12.*t29.*t1975)./2.0;
t1978 = t683+t684+t1133+t1139+t1909;
t1994 = -t1993;
t2004 = -t2003;
t2016 = -t2014;
t2032 = t1294+t1295+t1621+t1622+t1896;
t2033 = t1331+t1332+t1621+t1622+t1910;
t2049 = t859+t860+t1133+t1139+t1668+t1703+t1850+t1863;
t2054 = -t2053;
t2059 = -t2058;
t2066 = t781+t783+t1134+t1138+t1668+t1703+t1846+t1860+t1863;
t2076 = t1429+t1615+t1679+t1693+t1708+t1716+t1744+t1842;
t2086 = -t2085;
t2089 = -t2088;
t2092 = -t2091;
t2100 = qd5.*t2099;
t2103 = t664+t667+t720+t723+t1243+t1244+t1340+t1341+t1543+t1544+t1561+t1564+t1610+t1627+t1639+t1873+t1893+t1946+t1947;
t2106 = t1420+t1457+t1462+t1615+t1679+t1693+t1706+t1711+t1743+t1842+t2012+t2015;
t2107 = t1420+t1457+t1462+t1669+t1679+t1693+t1736+t1740+t1778+t1842+t2012+t2015;
t2109 = t1518+t1788+t1809+t1811+t1827+t1830+t2005+t2024+t2025;
t2111 = t1745+t1798+t1800+t1808+t1853+t1855+t1979+t2000+t2002;
t2119 = t1319+t1379+t1385+t1613+t1671+t1672+t1725+t1787+t1814+t1821+t1823+t1824+t1828+t1847+t1848+t1985+t1986+t2003+t2019+t2022;
t2120 = t1319+t1379+t1385+t1613+t1687+t1688+t1725+t1787+t1821+t1823+t1824+t1828+t1838+t1847+t1848+t1985+t1986+t2003+t2019+t2022;
et7 = t1313+t1613+t1653-t1659+t1660+t1725+t1748+t1799+t1821+t1823+t1847+t1848+t1869-t1889+t2006-t2007+(t132.*(t590+t600-t958-t1017-t1018+t453.*(t61-t241).*8.084033333333334e-4))./2.0+(t172.*(t589+t602-t953-t1030-t1032+t452.*(t60-t192).*8.084033333333334e-4))./2.0;
et8 = (t12.*t29.*(t697+t945-t1211-t1213+t194.*(-t270-t294+t334+t337+t396+t2.*t25.*(t60-t192)).*8.084033333333334e-4+t238.*(-t269-t295+t352+t356+t385+t8.*t25.*(t61-t241)).*8.084033333333334e-4))./2.0+(t2.*t763.*(t444-t445-t639+t969))./2.0-(t6.*t29.*t1583)./2.0;
et9 = (t29.*t30.*(t779+t1253+t907.*(t61-t241).*8.084033333333334e-4))./2.0+(t2.*t491.*(t429-t960))./2.0+(t8.*t491.*(t446-t970))./2.0;
t2127 = -qd6.*(et7+et8+et9);
t1594 = -t1589;
t1726 = -t1722;
t2034 = t1304+t1306+t1662+t1902+t1905;
t2036 = t1336+t1337+t1696+t1902+t1905;
t2038 = t1344+t1346+t1772+t1902+t1905;
t2040 = t1368+t1369+t1806+t1902+t1905;
t2042 = t1245+t1246+t1876+t1902+t1905;
t2044 = t1245+t1246+t1902+t1905+t1906;
t2077 = -qd6.*(t1420-t1615+t1681+t1695+t1706+t1711+t1743+t1843);
t2080 = t1420+t1670+t1681+t1695+t1736+t1740+t1778+t1843;
t2082 = t1304+t1306+t1665+t1700+t1849+t1862+t1902+t1905;
t2083 = t1336+t1337+t1665+t1700+t1845+t1864+t1902+t1905;
t2093 = t1303+t1305+t1667+t1702+t1845+t1859+t1862+t1902+t1905;
t2101 = -t2100;
t2104 = t1596+t1777+t1779+t1789+t1835+t1840+t1976+t1996+t1997;
et10 = t1591-t1777+t1834+t1839-t1976+(t132.*(t687+t906-t1277-t1472+t1279.*(t61-t241).*8.084033333333334e-4+t7.*t132.*(t291-t477+t172.*(t60-t192)).*8.084033333333334e-4))./2.0;
et11 = (t172.*(t676+t913-t1285-t1467+t1278.*(t60-t192).*8.084033333333334e-4+t7.*t172.*(t291-t477+t172.*(t60-t192)).*8.084033333333334e-4))./2.0+t1522.*(t446-t970)-(t6.*t29.*t1775)./2.0;
t2105 = -qd6.*(et10+et11);
t2108 = t552+t554+t664+t667+t1180+t1183+t1340+t1341+t1501+t1502+t1543+t1544+t1549+t1610+t1684+t1727+t1873+t1926+t1946+t1947;
t2110 = qd6.*t2109;
t2112 = t552+t554+t720+t723+t1180+t1183+t1340+t1341+t1501+t1502+t1549+t1561+t1564+t1639+t1727+t1759+t1893+t1926+t1946+t1947;
t2113 = t1154+t1155+t1207+t1209+t1520+t1526+t1609+t1626+t1638+t1770+t1776+t1783+t1790+t1872+t1892+t1923+t1924+t1991+t1992;
t2116 = t1746+t1797+t1802+t1804+t1854+t1856+t1888+t1934+t1937+t1964+t1965+t1980+t1999+t2001;
t2121 = t1319+t1379+t1385+t1613+t1658+t1659+t1725+t1787+t1821+t1823+t1824+t1828+t1847+t1848+t1870+t1985+t1986+t2003+t2019+t2022;
t2122 = t1319+t1379+t1385+t1590+t1611+t1655+t1661+t1671+t1672+t1721+t1750+t1801+t1803+t1814+t1820+t1822+t1851+t1852+t1889+t1941+t1942+t1981+t2007+t2008;
t2124 = t1319+t1379+t1385+t1590+t1611+t1655+t1661+t1687+t1688+t1721+t1750+t1801+t1803+t1820+t1822+t1838+t1851+t1852+t1889+t1941+t1942+t1981+t2007+t2008;
t2126 = t1319+t1379+t1385+t1590+t1611+t1655+t1658+t1659+t1661+t1721+t1750+t1801+t1803+t1820+t1822+t1851+t1852+t1870+t1889+t1941+t1942+t1981+t2007+t2008;
t2039 = qd3.*t2038;
t2041 = qd3.*t2040;
t2081 = qd6.*t2080;
t2098 = t1594+t1646+t1648+t1882+t1913+t1915+t2014+t2017;
t2114 = t1101+t1103+t1154+t1155+t1481+t1482+t1548+t1609+t1683+t1726+t1749+t1756+t1770+t1776+t1872+t1923+t1924+t1925+t1991+t1992;
t2115 = t1101+t1103+t1207+t1209+t1481+t1482+t1548+t1638+t1726+t1749+t1756+t1758+t1783+t1790+t1892+t1923+t1924+t1925+t1991+t1992;
t2117 = qd5.*t2116;
t2118 = -t2117;
et12 = qrdd4.*(t1135+t1147+t1222+t1223)+qrdd3.*(t1135+t1147+t1263+t1267)+qrdd2.*(t1135+t1147+t1317+t1320)+qrd1.*(-qd5.*t1680+qd4.*t1857+qd3.*t1898+qd2.*t1914)+qrdd1.*(t966+t1049.^2+t1052.^2)+qrd2.*(t1916+qd2.*(t1516+t1523-t2.*t574.*t892+t8.*t574.*t888+t2.*t575.*t1052+t8.*t575.*t1049)-qd4.*t2028+qd3.*t2030-qd5.*t2079)-qrdd5.*(t1463+t1466+t25.*t966+t2.*t29.*t1122+t8.*t29.*t1123);
et13 = -qrd5.*(t1694+qd4.*t2071+qd2.*t2079+qd3.*t2078+qd5.*(-t382.*t990-t592.*t1049+t373.*(t426-t712)+t1052.*(t243-t422)-t12.*t25.*t68.*2.031081666666667e-3+t2.*t29.*t1046+t8.*t29.*(t604-t630)))-qrd4.*(t1861+qd2.*t2028+qd3.*t2027+qd5.*t2071+qd4.*(t1227+t1228+t1515+t1524+t2.*t363.*t570-t8.*t363.*t568))+qrd3.*(t1900-qd4.*t2027+qd2.*t2030-qd5.*t2078+qd3.*(t1272+t1273+t1516+t1523-t2.*t480.*t812+t8.*t480.*t819));
et14 = t1844+t2068-qd5.*(-t25.*t1168+t372.*t1238+t380.*t1234+t877.*t1048+t886.*t1051+t8.*t29.*t1677+t2.*t29.*(t326-t350+t726-t727-t755+t12.*t39.*(t60-t192).*8.084033333333334e-4))+qd4.*(t1007+t1012-t1137+t1299+t1300-t1316+t1398-t1418+t1428+t1685+t1686+t1738+t1741-t1810-t1815+(t8.*t25.*(t332+t817+t238.*(t61-t241).*8.084033333333334e-4))./2.0);
et15 = qd3.*(t1082+t1090-t1137+t1299+t1300-t1316+t1398-t1487+t1493+t1685+t1686+t1738+t1741-t1810-t1815+(t8.*t25.*(t332+t817+t238.*(t61-t241).*8.084033333333334e-4))./2.0)+qd2.*(t1119+t1120-t1137+t1299+t1300-t1316+t1398-t1531+t1533+t1685+t1686+t1738+t1741-t1810-t1815+(t8.*t25.*(t332+t817+t238.*(t61-t241).*8.084033333333334e-4))./2.0);
et16 = qrd4;
et17 = t1890-qd3.*t2035-qd2.*t2037-qd4.*(t1383+t1384+t1719+t1720-t2.*t569.*t763+t8.*t567.*t763)+qd5.*(t1007+t1012-t1137+t1299+t1300-t1316+t1398-t1418+t1428+t1685+t1686+t1738+t1741-t1810-t1815+(t8.*t25.*(t332+t817+t238.*(t61-t241).*8.084033333333334e-4))./2.0)+qd6.*(t1144-t1325+t1394+t1404+t1407+t1751-t1753+t1768+t1771+(t29.*t30.*(t332+t817+t238.*(t61-t241).*8.084033333333334e-4))./2.0);
et18 = -1.0;
et19 = qrd3;
et20 = t1939-qd4.*t2035-qd2.*t2043-qd3.*(t1424+t1427+t1719+t1720-t2.*t811.*t863+t8.*t818.*t863)+qd5.*(t1082+t1090-t1137+t1299+t1300-t1316+t1398-t1487+t1493+t1685+t1686+t1738+t1741-t1810-t1815+(t8.*t25.*(t332+t817+t238.*(t61-t241).*8.084033333333334e-4))./2.0)+qd6.*(t1144-t1325+t1404+t1469+t1479+t1751-t1753+t1768+t1771+(t29.*t30.*(t332+t817+t238.*(t61-t241).*8.084033333333334e-4))./2.0);
et21 = -1.0;
et22 = qd4.*(t1144-t1325+t1394+t1404+t1407+t1751-t1753+t1768+t1771+(t29.*t30.*(t332+t817+t238.*(t61-t241).*8.084033333333334e-4))./2.0)+qd3.*(t1144-t1325+t1404+t1469+t1479+t1751-t1753+t1768+t1771+(t29.*t30.*(t332+t817+t238.*(t61-t241).*8.084033333333334e-4))./2.0);
et23 = qd2.*(t1144-t1325+t1404+t1497+t1510+t1751-t1753+t1768+t1771+(t29.*t30.*(t332+t817+t238.*(t61-t241).*8.084033333333334e-4))./2.0)+qd5.*(t1224+t1342+t1349+t1423+t1434+t1707+t1712+t1735+t1737+(t6.*t29.*t1112)./2.0);
et24 = t1952-qd2.*(t1719+t1720-t2.*t891.*t914+t8.*t887.*t914+t2.*t921.*t1051+t8.*t921.*t1048)-qd4.*t2037-qd3.*t2043+qd5.*(t1119+t1120-t1137+t1299+t1300-t1316+t1398-t1531+t1533+t1685+t1686+t1738+t1741-t1810-t1815+(t8.*t25.*(t332+t817+t238.*(t61-t241).*8.084033333333334e-4))./2.0);
et25 = qd6.*(t1144-t1325+t1404+t1497+t1510+t1751-t1753+t1768+t1771+(t29.*t30.*(t332+t817+t238.*(t61-t241).*8.084033333333334e-4))./2.0);
et26 = -qrd5.*(et14+et15)+et16.*et17.*et18+et19.*et20.*et21+qrdd4.*(-t1377+t1380+t1381+t2.*(t332+t817+t238.*(t61-t241).*8.084033333333334e-4))+qrdd3.*(-t1377+t1416+t1417+t2.*(t332+t817+t238.*(t61-t241).*8.084033333333334e-4));
et27 = qrdd2.*(-t1377+t1439+t1441+t2.*(t332+t817+t238.*(t61-t241).*8.084033333333334e-4))+qrdd1.*(t1112+t1048.^2+t1051.^2)-qrdd6.*(t172.*t1370-t132.*(t332+t817+t238.*(t61-t241).*8.084033333333334e-4)+t1051.*(t429-t960)+t1048.*(t446-t970)+t12.*t29.*t1112)-qrd6.*(et22+et23)-qrd2.*(et24+et25)-qrd1.*(qd4.*t1887+qd3.*t1938+qd2.*t1950+qd5.*(-t170+t657+t679+t1215+t1220));
et28 = -qrdd5.*(t1577+t1578+t25.*t1112+t2.*t29.*t1370+t8.*t29.*(t332+t817+t238.*(t61-t241).*8.084033333333334e-4));
et29 = t127+t222+t230+t258+t267-qrd4.*(t1868+qd2.*t1969+qd3.*t2049-qd5.*(t552+t554+t720+t723+t1340+t1341+t1501+t1502+t1551+t1558+t1568+t1639+t1727+t1759+t1895+t1926)+qd4.*(t1796+t1907+t1969))+qrd2.*(t1973-qd4.*t1969+qd5.*(t719+t722+t1340+t1341+t1631)+qd2.*(t1134+t1138+t1367.*t1509+t15.*t574.*t575+t17.*t574.*t575))-qrd1.*(t1916+qd4.*(t533-t785-t1528+t1529+t1867)+qd3.*(t533-t785-t1528+t1529+t1930)-qd5.*(t787+t799+t872+t880+t1022+t1079+t1125+t1126+t1176+t1177+t1411+t1413+t1537+t1538+t1656+t1657)+qd2.*(t533-t785-t1528+t1529));
et30 = qrd5.*(t2061+qd4.*(t552+t554+t720+t723+t1129+t1132+t1167+t1169+t1232+t1239+t1340+t1341+t1501+t1502+t1551+t1558+t1568+t1639+t1727+t1759+t1895+t1926+t1949+t1951)+qd2.*(t719+t722+t1129+t1132+t1167+t1169+t1232+t1239+t1340+t1341+t1631+t1949+t1951)+qd3.*(t664+t667+t720+t723+t1129+t1132+t1167+t1169+t1232+t1239+t1340+t1341+t1543+t1544+t1558+t1568+t1610+t1639+t1873+t1895+t1949+t1951)-qd5.*(t1096+t1102+t1270+t1347+t1353+t1442+t2094-t778.*t1509-t8.*t574.*t592+t2.*t574.*(t243-t422)))+qrdd3.*t1984+qrdd4.*t2009+qrdd2.*(t1199+t1201+t15.*t580+t17.*t580+t1509.^2)+qrdd5.*(t1225-t1226-t1265-t1766+t25.*(t523-t789)+t8.*t574.*(t426-t712))+qrd3.*(-t1933+t1973+qd2.*t1972-qd4.*t2049+qd5.*(t664+t667+t720+t723+t1340+t1341+t1543+t1544+t1558+t1568+t1610+t1639+t1873+t1895))+qrdd1.*(t1109+t1317+t1320);
et31 = t1313+t1613+t1653+t1660-t1688+t1725+t1748+t1799+t1821+t1823+t1837+t1847+t1848-t1889+t2006-t2007+(t132.*(t590+t600-t958-t1017-t1018+t453.*(t61-t241).*8.084033333333334e-4))./2.0+(t172.*(t589+t602-t953-t1030-t1032+t452.*(t60-t192).*8.084033333333334e-4))./2.0;
et32 = (t12.*t29.*(t697+t945-t1211-t1213+t194.*(-t270-t294+t334+t337+t396+t2.*t25.*(t60-t192)).*8.084033333333334e-4+t238.*(-t269-t295+t352+t356+t385+t8.*t25.*(t61-t241)).*8.084033333333334e-4))./2.0+(t2.*t914.*(t444-t445-t639+t969))./2.0-(t6.*t29.*t1583)./2.0;
et33 = (t29.*t30.*(t779+t1253+t907.*(t61-t241).*8.084033333333334e-4))./2.0+(t2.*t491.*(t429-t960))./2.0+(t8.*t491.*(t446-t970))./2.0;
et34 = t1313+t1613+t1653+t1660-t1688+t1725+t1787+t1821+t1823+t1824+t1828+t1837+t1847+t1848-t1889+t2003+t2019+t2022+(t132.*(t590+t600-t958-t1017-t1018+t453.*(t61-t241).*8.084033333333334e-4))./2.0+(t172.*(t589+t602-t953-t1030-t1032+t452.*(t60-t192).*8.084033333333334e-4))./2.0+(t2.*t914.*(t444-t445-t639+t969))./2.0-(t6.*t29.*t1583)./2.0;
et35 = (t2.*t491.*(t429-t960))./2.0+(t8.*t491.*(t446-t970))./2.0;
et36 = t127+t222+t230+t257+t266-qrd5.*(t2091-qd4.*(t1101+t1103+t1207+t1209+t1550+t1588+t1638+t1640+t1647+t1726+t1749+t1756+t1758+t1781+t1786+t1879+t1894+t1904+t1908+t1923+t1924+t1925+t1994+t1995)-qd2.*(t1190+t1192+t1588+t1630+t1640+t1647+t1879+t1904+t1908+t1923+t1924+t1994+t1995)-qd3.*(t1154+t1155+t1207+t1209+t1588+t1609+t1638+t1640+t1647+t1770+t1776+t1781+t1786+t1872+t1879+t1894+t1904+t1908+t1923+t1924+t1994+t1995)+qd5.*(t1400+t1402-t1436+t1746+t1797+t1802+t1804+t1854+t1856-t1883+t1927+t1980+t1999+t2001-t777.*t1508+t2.*t29.*(t589+t602-t953-t1030-t1032+t452.*(t60-t192).*8.084033333333334e-4)-t8.*t877.*t914-t2.*t886.*t914)+qd6.*(et31+et32+et33));
et37 = qrdd3.*t2031+qrdd4.*t2033+qrd6.*(t2065-t2110+qd3.*(t1589+t1643+t1649+t1881+t1912+t1917+t2016+t2018+t2062)+qd4.*(t1589+t1643+t1649+t1881+t1912+t1917+t2016+t2018+t2080)-qd5.*(et34+et35)+qd2.*(t1589+t1643+t1649+t1881+t1912+t1917+t2016+t2018))+qrdd1.*(t535+t1025+t1056+t1439+t1441)+qrdd2.*(t1621+t1622+t15.*t923+t17.*t923+t1508.^2)+qrd3.*(t2041+t2063+qd2.*t2040+qd4.*t2083+qd1.*(t1350+t1354-t1356+t1358)+qd5.*(t1154+t1155+t1207+t1209+t1609+t1638+t1770+t1776+t1781+t1786+t1872+t1894+t1923+t1924));
et38 = qrd2.*(t2041+qd4.*t2036+qd2.*(t1902+t1905+t1366.*t1508+t15.*t914.*t921+t17.*t914.*t921)-qd5.*(-t1190-t1192+t1623+(t8.*(t589+t602-t953-t1030-t1032+t452.*(t60-t192).*8.084033333333334e-4))./2.0+(t2.*(t590+t600-t958-t1017-t1018+t453.*(t61-t241).*8.084033333333334e-4))./2.0));
et39 = -qrd1.*(t1955+t2075+qd4.*(t1960+t2026)+qd3.*(t1966+t2026)+qd5.*(t534+t547+t898+t904+t972+t974+t1119+t1120+t1137+t1299+t1300+t1316+t1401+t1406+t1531+t1534+t1739+t1742+t1810+t1815)+qd2.*t2026)+qrdd6.*(t1513+t1525+t1585+t1651+t1652+t1674)-qrdd5.*(t1539+t1541+t1586+t1636+t1637+t1765)+qrd4.*(t2081+qd2.*t2036+qd3.*t2083+qd1.*(t1235+t1241-t1321+t1323)+qd5.*(t1101+t1103+t1207+t1209+t1550+t1638+t1726+t1749+t1756+t1758+t1781+t1786+t1894+t1923+t1924+t1925)+qd4.*(t1793-t1906+t2036));
et40 = t222+t230+t258+t267-qrd4.*(t1836+qd2.*(t782+t784+t1133+t1139+t1668+t1703+t1846-t1863)+qd3.*t1968-qd5.*(t552+t554+t664+t667+t1340+t1341+t1501+t1502+t1542+t1545+t1551+t1610+t1684+t1727+t1875+t1926)+qd4.*(t1796+t1877+t1968))+qrd5.*(t2056+qd4.*(t552+t554+t664+t667+t1129+t1132+t1167+t1169+t1232+t1239+t1340+t1341+t1501+t1502+t1542+t1545+t1551+t1610+t1684+t1727+t1875+t1926+t1949+t1951)+qd3.*(t663+t666+t1129+t1132+t1167+t1169+t1232+t1239+t1340+t1341+t1602+t1949+t1951)+qd2.*(t664+t667+t720+t723+t1129+t1132+t1167+t1169+t1232+t1239+t1340+t1341+t1542+t1545+t1561+t1564+t1610+t1639+t1875+t1893+t1949+t1951)-qd5.*(t1096+t1102+t1270+t1347+t1353+t1442+t2094-t778.*t1452-t8.*t480.*t592+t2.*t480.*(t243-t422)))+qrdd2.*t1984+qrdd4.*t1987+qrdd3.*(t1199+t1201+t15.*t496+t17.*t496+t1452.^2);
et41 = qrdd5.*(t1225-t1226-t1237-t1731+t25.*(t523-t789)+t8.*t480.*(t426-t712))+qrdd1.*(t1109+t1263+t1267)+qrd3.*(t1971+qd2.*t1970-qd4.*t1968+qd5.*(t663+t666+t1340+t1341+t1602))+qrd2.*(t1933+t1971-qd4.*(t782+t784+t1133+t1139+t1668+t1703+t1846-t1863)+qd5.*(t664+t667+t720+t723+t1340+t1341+t1542+t1545+t1561+t1564+t1610+t1639+t1875+t1893)+qd2.*(t1134+t1138+t1367.*t1452+t15.*t480.*t575+t17.*t480.*t575))-qrd1.*(t1900+qd4.*(t533-t785-t1528+t1529+t1831)-qd5.*(t787+t799+t804+t810+t1022+t1079+t1125+t1126+t1176+t1177+t1375+t1378+t1537+t1538+t1656+t1657)+qd3.*(t533-t785-t1528+t1529)+qd2.*(t533-t785+t1146+t1148-t1153+t1156-t1528+t1529));
et42 = t1313+t1613+t1653+t1660-t1672+t1725+t1748+t1799+t1813+t1821+t1823+t1847+t1848-t1889+t2006-t2007+(t132.*(t590+t600-t958-t1017-t1018+t453.*(t61-t241).*8.084033333333334e-4))./2.0+(t172.*(t589+t602-t953-t1030-t1032+t452.*(t60-t192).*8.084033333333334e-4))./2.0;
et43 = (t12.*t29.*(t697+t945-t1211-t1213+t194.*(-t270-t294+t334+t337+t396+t2.*t25.*(t60-t192)).*8.084033333333334e-4+t238.*(-t269-t295+t352+t356+t385+t8.*t25.*(t61-t241)).*8.084033333333334e-4))./2.0+(t2.*t863.*(t444-t445-t639+t969))./2.0-(t6.*t29.*t1583)./2.0;
et44 = (t29.*t30.*(t779+t1253+t907.*(t61-t241).*8.084033333333334e-4))./2.0+(t2.*t491.*(t429-t960))./2.0+(t8.*t491.*(t446-t970))./2.0;
et45 = t1313+t1613+t1653+t1660-t1672+t1725+t1787+t1813+t1821+t1823+t1824+t1828+t1847+t1848-t1889+t2003+t2019+t2022+(t132.*(t590+t600-t958-t1017-t1018+t453.*(t61-t241).*8.084033333333334e-4))./2.0+(t172.*(t589+t602-t953-t1030-t1032+t452.*(t60-t192).*8.084033333333334e-4))./2.0+(t2.*t863.*(t444-t445-t639+t969))./2.0-(t6.*t29.*t1583)./2.0;
et46 = (t2.*t491.*(t429-t960))./2.0+(t8.*t491.*(t446-t970))./2.0;
et47 = t222+t230+t257+t266-qrd5.*(t2088-qd4.*(t1101+t1103+t1154+t1155+t1550+t1588+t1609+t1640+t1647+t1683+t1726+t1749+t1756+t1767+t1774+t1874+t1879+t1904+t1908+t1923+t1924+t1925+t1994+t1995)-qd3.*(t1140+t1141+t1588+t1601+t1640+t1647+t1879+t1904+t1908+t1923+t1924+t1994+t1995)-qd2.*(t1154+t1155+t1207+t1209+t1588+t1609+t1638+t1640+t1647+t1767+t1774+t1783+t1790+t1874+t1879+t1892+t1904+t1908+t1923+t1924+t1994+t1995)+qd5.*(t1400+t1402-t1436+t1746+t1797+t1802+t1804+t1854+t1856-t1883+t1927+t1980+t1999+t2001-t777.*t1451+t2.*t29.*(t589+t602-t953-t1030-t1032+t452.*(t60-t192).*8.084033333333334e-4)-t8.*t863.*t877-t2.*t863.*t886)+qd6.*(et42+et43+et44));
et48 = qrd3.*(t2039+qd4.*t2034+qd2.*t2038-qd5.*(-t1140-t1141+t1598+(t8.*(t589+t602-t953-t1030-t1032+t452.*(t60-t192).*8.084033333333334e-4))./2.0+(t2.*(t590+t600-t958-t1017-t1018+t453.*(t61-t241).*8.084033333333334e-4))./2.0));
et49 = qrd2.*(t1967+t2039+qd4.*t2082+qd6.*(t1706+t1711-t1736+t1743-t1778+(t8.*t914.*(t263+t456-t922-t978))./2.0)+qd5.*(t1154+t1155+t1207+t1209+t1609+t1638+t1767+t1774+t1783+t1790+t1874+t1892+t1923+t1924)+qd2.*(t1902+t1905+t1366.*t1451+t15.*t863.*t921+t17.*t863.*t921))+qrdd2.*t2031+qrdd4.*t2032+qrdd1.*(t535+t1025+t1056+t1416+t1417)+qrdd3.*(t1621+t1622+t15.*t881+t17.*t881+t1451.^2)-qrd1.*(t1940+t2073+qd4.*(t1956+t2026)+qd5.*(t534+t547+t898+t904+t972+t974+t1082+t1090+t1137+t1299+t1300+t1316+t1401+t1406+t1487+t1496+t1739+t1742+t1810+t1815)+qd3.*t2026+qd2.*(t1350+t1354-t1356+t1358+t2026));
et50 = qrd4.*(qd6.*(t1420-t1615+t1681+t1695+t1706+t1711+t1743+t1843)+qd3.*t2034+qd2.*t2082+qd1.*(t1185+t1194-t1259+t1260)+qd5.*(t1101+t1103+t1154+t1155+t1550+t1609+t1683+t1726+t1749+t1756+t1767+t1774+t1874+t1923+t1924+t1925)+qd4.*(t1793-t1876+t2034))+qrd6.*(t2058-t2110+qd2.*(t1589+t1643+t1649+t1706+t1711-t1736+t1743-t1778+t1881+t1912+t1917+t2016+t2018+(t8.*t914.*(t263+t456-t922-t978))./2.0)-qd5.*(et45+et46)+qd4.*(t1420+t1589-t1615+t1643+t1649+t1681+t1695+t1706+t1711+t1743+t1843+t1881+t1912+t1917+t2016+t2018)+qd3.*(t1589+t1643+t1649+t1881+t1912+t1917+t2016+t2018))+qrdd6.*(t1483+t1488+t1585+t1642+t1651+t1652)-qrdd5.*(t1514+t1517+t1586+t1636+t1637+t1730);
et51 = t230+t258+t267+qrd5.*(t2051+qd3.*(t552+t554+t664+t667+t1129+t1132+t1167+t1169+t1232+t1239+t1340+t1341+t1499+t1504+t1543+t1544+t1549+t1610+t1690+t1727+t1873+t1929+t1949+t1951)+qd2.*(t552+t554+t720+t723+t1129+t1132+t1167+t1169+t1232+t1239+t1340+t1341+t1499+t1504+t1549+t1561+t1564+t1639+t1727+t1761+t1893+t1929+t1949+t1951)+qd4.*(t551+t553+t1129+t1132+t1167+t1169+t1232+t1239+t1340+t1341+t1718+t1949+t1951)-qd5.*(t1096+t1102+t1270+t1347+t1353+t1442+t2094-t778.*t1593-t8.*t363.*t592+t2.*t363.*(t243-t422)))+qrd2.*(t1868-qd4.*t1978+qd3.*t2066+qd5.*(t552+t554+t720+t723+t1340+t1341+t1499+t1504+t1549+t1561+t1564+t1639+t1727+t1761+t1893+t1929)+qd2.*(t1134+t1138+t1699+t1367.*t1593+t1486.*t1509+t15.*t363.*t575+t17.*t363.*t575));
